simulink model "model"  (R2014a)
(part 7 of 8)

  房総線_CN_151379730_500000_CN_168727982_500000 : powerlib/Elements/Distributed Parameters Line  Phases=3  Frequency=60  Resistance=[0.01273 0.3864]  Inductance="[0.9337e-3  4.1264e-3]"  Capacitance=[12.74e-9 7.751e-9]  Length=39.9619  x1=[0 0 0 0; 0.0001244 0 0 0; 0.0002488 0 0 0; 0.0003733 0 0 0; 0.0004977 0 0 0; 0.0006221 0 0 0]  x2=[0 0 0 0; 0.0001244 0 0 0; 0.0002488 0 0 0; 0.0003733 0 0 0; 0.0004977 0 0 0; 0.0006221 0 0 0]  x3=[0 0 0 0; 0.0001244 0 0 0; 0.0002488 0 0 0; 0.0003733 0 0 0; 0.0004977 0 0 0; 0.0006221 0 0 0]  x4=[0 0 0 0; 0.0001244 0 0 0; 0.0002488 0 0 0; 0.0003733 0 0 0; 0.0004977 0 0 0; 0.0006221 0 0 0]  x5=0  V1=ones(3,3)  V2=ones(3,3)  I1=ones(3,3)  I2=ones(3,3)  nHarmo=1  Measurements=None
  新京葉線_CN_133135172_500000_CN_151706977_500000 : powerlib/Elements/Distributed Parameters Line  Phases=3  Frequency=60  Resistance=[0.01273 0.3864]  Inductance="[0.9337e-3  4.1264e-3]"  Capacitance=[12.74e-9 7.751e-9]  Length=22.6829  x1=[0 0 0 0; 0.0001244 0 0 0; 0.0002488 0 0 0; 0.0003733 0 0 0; 0.0004977 0 0 0; 0.0006221 0 0 0]  x2=[0 0 0 0; 0.0001244 0 0 0; 0.0002488 0 0 0; 0.0003733 0 0 0; 0.0004977 0 0 0; 0.0006221 0 0 0]  x3=[0 0 0 0; 0.0001244 0 0 0; 0.0002488 0 0 0; 0.0003733 0 0 0; 0.0004977 0 0 0; 0.0006221 0 0 0]  x4=[0 0 0 0; 0.0001244 0 0 0; 0.0002488 0 0 0; 0.0003733 0 0 0; 0.0004977 0 0 0; 0.0006221 0 0 0]  x5=0  V1=ones(3,3)  V2=ones(3,3)  I1=ones(3,3)  I2=ones(3,3)  nHarmo=1  Measurements=None
  新京葉線_CN_133135172_500000_CN_168727982_500000 : powerlib/Elements/Distributed Parameters Line  Phases=3  Frequency=60  Resistance=[0.01273 0.3864]  Inductance="[0.9337e-3  4.1264e-3]"  Capacitance=[12.74e-9 7.751e-9]  Length=45.831  x1=[0 0 0 0; 0.0001244 0 0 0; 0.0002488 0 0 0; 0.0003733 0 0 0; 0.0004977 0 0 0; 0.0006221 0 0 0]  x2=[0 0 0 0; 0.0001244 0 0 0; 0.0002488 0 0 0; 0.0003733 0 0 0; 0.0004977 0 0 0; 0.0006221 0 0 0]  x3=[0 0 0 0; 0.0001244 0 0 0; 0.0002488 0 0 0; 0.0003733 0 0 0; 0.0004977 0 0 0; 0.0006221 0 0 0]  x4=[0 0 0 0; 0.0001244 0 0 0; 0.0002488 0 0 0; 0.0003733 0 0 0; 0.0004977 0 0 0; 0.0006221 0 0 0]  x5=0  V1=ones(3,3)  V2=ones(3,3)  I1=ones(3,3)  I2=ones(3,3)  nHarmo=1  Measurements=None
  新京葉線_CN_151706977_275000_CN_168852840_275000 : powerlib/Elements/Distributed Parameters Line  Phases=3  Frequency=60  Resistance=[0.01273 0.3864]  Inductance="[0.9337e-3  4.1264e-3]"  Capacitance=[12.74e-9 7.751e-9]  Length=70.4447  x1=[0 0 0 0; 0.0001244 0 0 0; 0.0002488 0 0 0; 0.0003733 0 0 0; 0.0004977 0 0 0; 0.0006221 0 0 0]  x2=[0 0 0 0; 0.0001244 0 0 0; 0.0002488 0 0 0; 0.0003733 0 0 0; 0.0004977 0 0 0; 0.0006221 0 0 0]  x3=[0 0 0 0; 0.0001244 0 0 0; 0.0002488 0 0 0; 0.0003733 0 0 0; 0.0004977 0 0 0; 0.0006221 0 0 0]  x4=[0 0 0 0; 0.0001244 0 0 0; 0.0002488 0 0 0; 0.0003733 0 0 0; 0.0004977 0 0 0; 0.0006221 0 0 0]  x5=0  V1=ones(3,3)  V2=ones(3,3)  I1=ones(3,3)  I2=ones(3,3)  nHarmo=1  Measurements=None
  新古河線_(Shin_Koga_Sen)_CN_133135172_500000_CN_133641619_500000 : powerlib/Elements/Distributed Parameters Line  Phases=3  Frequency=60  Resistance=[0.01273 0.3864]  Inductance="[0.9337e-3  4.1264e-3]"  Capacitance=[12.74e-9 7.751e-9]  Length=56.7109  x1=[0 0 0 0; 0.0001244 0 0 0; 0.0002488 0 0 0; 0.0003733 0 0 0; 0.0004977 0 0 0; 0.0006221 0 0 0]  x2=[0 0 0 0; 0.0001244 0 0 0; 0.0002488 0 0 0; 0.0003733 0 0 0; 0.0004977 0 0 0; 0.0006221 0 0 0]  x3=[0 0 0 0; 0.0001244 0 0 0; 0.0002488 0 0 0; 0.0003733 0 0 0; 0.0004977 0 0 0; 0.0006221 0 0 0]  x4=[0 0 0 0; 0.0001244 0 0 0; 0.0002488 0 0 0; 0.0003733 0 0 0; 0.0004977 0 0 0; 0.0006221 0 0 0]  x5=0  V1=ones(3,3)  V2=ones(3,3)  I1=ones(3,3)  I2=ones(3,3)  nHarmo=1  Measurements=None
  新吾妻線_CN_169963236_500000_CN_66098469_500000 : powerlib/Elements/Distributed Parameters Line  Phases=3  Frequency=60  Resistance=[0.01273 0.3864]  Inductance="[0.9337e-3  4.1264e-3]"  Capacitance=[12.74e-9 7.751e-9]  Length=6.9915  x1=[0 0 0 0; 0.0001244 0 0 0; 0.0002488 0 0 0; 0.0003733 0 0 0; 0.0004977 0 0 0; 0.0006221 0 0 0]  x2=[0 0 0 0; 0.0001244 0 0 0; 0.0002488 0 0 0; 0.0003733 0 0 0; 0.0004977 0 0 0; 0.0006221 0 0 0]  x3=[0 0 0 0; 0.0001244 0 0 0; 0.0002488 0 0 0; 0.0003733 0 0 0; 0.0004977 0 0 0; 0.0006221 0 0 0]  x4=[0 0 0 0; 0.0001244 0 0 0; 0.0002488 0 0 0; 0.0003733 0 0 0; 0.0004977 0 0 0; 0.0006221 0 0 0]  x5=0  V1=ones(3,3)  V2=ones(3,3)  I1=ones(3,3)  I2=ones(3,3)  nHarmo=1  Measurements=None
  新坂戸線_CN_128581912_500000_CN_133641619_500000 : powerlib/Elements/Distributed Parameters Line  Phases=3  Frequency=60  Resistance=[0.01273 0.3864]  Inductance="[0.9337e-3  4.1264e-3]"  Capacitance=[12.74e-9 7.751e-9]  Length=7.2466  x1=[0 0 0 0; 0.0001244 0 0 0; 0.0002488 0 0 0; 0.0003733 0 0 0; 0.0004977 0 0 0; 0.0006221 0 0 0]  x2=[0 0 0 0; 0.0001244 0 0 0; 0.0002488 0 0 0; 0.0003733 0 0 0; 0.0004977 0 0 0; 0.0006221 0 0 0]  x3=[0 0 0 0; 0.0001244 0 0 0; 0.0002488 0 0 0; 0.0003733 0 0 0; 0.0004977 0 0 0; 0.0006221 0 0 0]  x4=[0 0 0 0; 0.0001244 0 0 0; 0.0002488 0 0 0; 0.0003733 0 0 0; 0.0004977 0 0 0; 0.0006221 0 0 0]  x5=0  V1=ones(3,3)  V2=ones(3,3)  I1=ones(3,3)  I2=ones(3,3)  nHarmo=1  Measurements=None
  新多摩線_(Shin_Tama_Sen)_CN_149843487_500000_CN_145079972_500000 : powerlib/Elements/Distributed Parameters Line  Phases=3  Frequency=60  Resistance=[0.01273 0.3864]  Inductance="[0.9337e-3  4.1264e-3]"  Capacitance=[12.74e-9 7.751e-9]  Length=39.8761  x1=[0 0 0 0; 0.0001244 0 0 0; 0.0002488 0 0 0; 0.0003733 0 0 0; 0.0004977 0 0 0; 0.0006221 0 0 0]  x2=[0 0 0 0; 0.0001244 0 0 0; 0.0002488 0 0 0; 0.0003733 0 0 0; 0.0004977 0 0 0; 0.0006221 0 0 0]  x3=[0 0 0 0; 0.0001244 0 0 0; 0.0002488 0 0 0; 0.0003733 0 0 0; 0.0004977 0 0 0; 0.0006221 0 0 0]  x4=[0 0 0 0; 0.0001244 0 0 0; 0.0002488 0 0 0; 0.0003733 0 0 0; 0.0004977 0 0 0; 0.0006221 0 0 0]  x5=0  V1=ones(3,3)  V2=ones(3,3)  I1=ones(3,3)  I2=ones(3,3)  nHarmo=1  Measurements=None
  新所沢線_(Shin_Tokorozawa_Sen)_CN_145079972_500000_CN_133641619_500000 : powerlib/Elements/Distributed Parameters Line  Phases=3  Frequency=60  Resistance=[0.01273 0.3864]  Inductance="[0.9337e-3  4.1264e-3]"  Capacitance=[12.74e-9 7.751e-9]  Length=34.7552  x1=[0 0 0 0; 0.0001244 0 0 0; 0.0002488 0 0 0; 0.0003733 0 0 0; 0.0004977 0 0 0; 0.0006221 0 0 0]  x2=[0 0 0 0; 0.0001244 0 0 0; 0.0002488 0 0 0; 0.0003733 0 0 0; 0.0004977 0 0 0; 0.0006221 0 0 0]  x3=[0 0 0 0; 0.0001244 0 0 0; 0.0002488 0 0 0; 0.0003733 0 0 0; 0.0004977 0 0 0; 0.0006221 0 0 0]  x4=[0 0 0 0; 0.0001244 0 0 0; 0.0002488 0 0 0; 0.0003733 0 0 0; 0.0004977 0 0 0; 0.0006221 0 0 0]  x5=0  V1=ones(3,3)  V2=ones(3,3)  I1=ones(3,3)  I2=ones(3,3)  nHarmo=1  Measurements=None
  新榛名線_CN_169963227_500000_CN_195615141_500000 : powerlib/Elements/Distributed Parameters Line  Phases=3  Frequency=60  Resistance=[0.01273 0.3864]  Inductance="[0.9337e-3  4.1264e-3]"  Capacitance=[12.74e-9 7.751e-9]  Length=67.752  x1=[0 0 0 0; 0.0001244 0 0 0; 0.0002488 0 0 0; 0.0003733 0 0 0; 0.0004977 0 0 0; 0.0006221 0 0 0]  x2=[0 0 0 0; 0.0001244 0 0 0; 0.0002488 0 0 0; 0.0003733 0 0 0; 0.0004977 0 0 0; 0.0006221 0 0 0]  x3=[0 0 0 0; 0.0001244 0 0 0; 0.0002488 0 0 0; 0.0003733 0 0 0; 0.0004977 0 0 0; 0.0006221 0 0 0]  x4=[0 0 0 0; 0.0001244 0 0 0; 0.0002488 0 0 0; 0.0003733 0 0 0; 0.0004977 0 0 0; 0.0006221 0 0 0]  x5=0  V1=ones(3,3)  V2=ones(3,3)  I1=ones(3,3)  I2=ones(3,3)  nHarmo=1  Measurements=None
  新筑波線_(Shin_Tsukuba_Sen)_CN_133135172_500000_CN_132913106_500000 : powerlib/Elements/Distributed Parameters Line  Phases=3  Frequency=60  Resistance=[0.01273 0.3864]  Inductance="[0.9337e-3  4.1264e-3]"  Capacitance=[12.74e-9 7.751e-9]  Length=9.3755  x1=[0 0 0 0; 0.0001244 0 0 0; 0.0002488 0 0 0; 0.0003733 0 0 0; 0.0004977 0 0 0; 0.0006221 0 0 0]  x2=[0 0 0 0; 0.0001244 0 0 0; 0.0002488 0 0 0; 0.0003733 0 0 0; 0.0004977 0 0 0; 0.0006221 0 0 0]  x3=[0 0 0 0; 0.0001244 0 0 0; 0.0002488 0 0 0; 0.0003733 0 0 0; 0.0004977 0 0 0; 0.0006221 0 0 0]  x4=[0 0 0 0; 0.0001244 0 0 0; 0.0002488 0 0 0; 0.0003733 0 0 0; 0.0004977 0 0 0; 0.0006221 0 0 0]  x5=0  V1=ones(3,3)  V2=ones(3,3)  I1=ones(3,3)  I2=ones(3,3)  nHarmo=1  Measurements=None
  新茂木線_(Shin_Motegi_Sen)_CN_104530060_500000_CN_168839127_500000 : powerlib/Elements/Distributed Parameters Line  Phases=3  Frequency=60  Resistance=[0.01273 0.3864]  Inductance="[0.9337e-3  4.1264e-3]"  Capacitance=[12.74e-9 7.751e-9]  Length=27.1693  x1=[0 0 0 0; 0.0001244 0 0 0; 0.0002488 0 0 0; 0.0003733 0 0 0; 0.0004977 0 0 0; 0.0006221 0 0 0]  x2=[0 0 0 0; 0.0001244 0 0 0; 0.0002488 0 0 0; 0.0003733 0 0 0; 0.0004977 0 0 0; 0.0006221 0 0 0]  x3=[0 0 0 0; 0.0001244 0 0 0; 0.0002488 0 0 0; 0.0003733 0 0 0; 0.0004977 0 0 0; 0.0006221 0 0 0]  x4=[0 0 0 0; 0.0001244 0 0 0; 0.0002488 0 0 0; 0.0003733 0 0 0; 0.0004977 0 0 0; 0.0006221 0 0 0]  x5=0  V1=ones(3,3)  V2=ones(3,3)  I1=ones(3,3)  I2=ones(3,3)  nHarmo=1  Measurements=None
  東京中線_CN_133137636_275000_CN_128581912_275000 : powerlib/Elements/Distributed Parameters Line  Phases=3  Frequency=60  Resistance=[0.01273 0.3864]  Inductance="[0.9337e-3  4.1264e-3]"  Capacitance=[12.74e-9 7.751e-9]  Length=25.3762  x1=[0 0 0 0; 0.0001244 0 0 0; 0.0002488 0 0 0; 0.0003733 0 0 0; 0.0004977 0 0 0; 0.0006221 0 0 0]  x2=[0 0 0 0; 0.0001244 0 0 0; 0.0002488 0 0 0; 0.0003733 0 0 0; 0.0004977 0 0 0; 0.0006221 0 0 0]  x3=[0 0 0 0; 0.0001244 0 0 0; 0.0002488 0 0 0; 0.0003733 0 0 0; 0.0004977 0 0 0; 0.0006221 0 0 0]  x4=[0 0 0 0; 0.0001244 0 0 0; 0.0002488 0 0 0; 0.0003733 0 0 0; 0.0004977 0 0 0; 0.0006221 0 0 0]  x5=0  V1=ones(3,3)  V2=ones(3,3)  I1=ones(3,3)  I2=ones(3,3)  nHarmo=1  Measurements=None
  東京北線_(Tōkyō_Kita_Sen)_CN_133137636_275000_CN_151706977_275000 : powerlib/Elements/Distributed Parameters Line  Phases=3  Frequency=60  Resistance=[0.01273 0.3864]  Inductance="[0.9337e-3  4.1264e-3]"  Capacitance=[12.74e-9 7.751e-9]  Length=25.1708  x1=[0 0 0 0; 0.0001244 0 0 0; 0.0002488 0 0 0; 0.0003733 0 0 0; 0.0004977 0 0 0; 0.0006221 0 0 0]  x2=[0 0 0 0; 0.0001244 0 0 0; 0.0002488 0 0 0; 0.0003733 0 0 0; 0.0004977 0 0 0; 0.0006221 0 0 0]  x3=[0 0 0 0; 0.0001244 0 0 0; 0.0002488 0 0 0; 0.0003733 0 0 0; 0.0004977 0 0 0; 0.0006221 0 0 0]  x4=[0 0 0 0; 0.0001244 0 0 0; 0.0002488 0 0 0; 0.0003733 0 0 0; 0.0004977 0 0 0; 0.0006221 0 0 0]  x5=0  V1=ones(3,3)  V2=ones(3,3)  I1=ones(3,3)  I2=ones(3,3)  nHarmo=1  Measurements=None
  東京南線3;4号線_CN_128364781_275000_CN_379474501_275000 : powerlib/Elements/Distributed Parameters Line  Phases=3  Frequency=60  Resistance=[0.01273 0.3864]  Inductance="[0.9337e-3  4.1264e-3]"  Capacitance=[12.74e-9 7.751e-9]  Length=35.3731  x1=[0 0 0 0; 0.0001244 0 0 0; 0.0002488 0 0 0; 0.0003733 0 0 0; 0.0004977 0 0 0; 0.0006221 0 0 0]  x2=[0 0 0 0; 0.0001244 0 0 0; 0.0002488 0 0 0; 0.0003733 0 0 0; 0.0004977 0 0 0; 0.0006221 0 0 0]  x3=[0 0 0 0; 0.0001244 0 0 0; 0.0002488 0 0 0; 0.0003733 0 0 0; 0.0004977 0 0 0; 0.0006221 0 0 0]  x4=[0 0 0 0; 0.0001244 0 0 0; 0.0002488 0 0 0; 0.0003733 0 0 0; 0.0004977 0 0 0; 0.0006221 0 0 0]  x5=0  V1=ones(3,3)  V2=ones(3,3)  I1=ones(3,3)  I2=ones(3,3)  nHarmo=1  Measurements=None
  東京西線_CN_145080115_275000_CN_47110637_275000 : powerlib/Elements/Distributed Parameters Line  Phases=3  Frequency=60  Resistance=[0.01273 0.3864]  Inductance="[0.9337e-3  4.1264e-3]"  Capacitance=[12.74e-9 7.751e-9]  Length=13.2046  x1=[0 0 0 0; 0.0001244 0 0 0; 0.0002488 0 0 0; 0.0003733 0 0 0; 0.0004977 0 0 0; 0.0006221 0 0 0]  x2=[0 0 0 0; 0.0001244 0 0 0; 0.0002488 0 0 0; 0.0003733 0 0 0; 0.0004977 0 0 0; 0.0006221 0 0 0]  x3=[0 0 0 0; 0.0001244 0 0 0; 0.0002488 0 0 0; 0.0003733 0 0 0; 0.0004977 0 0 0; 0.0006221 0 0 0]  x4=[0 0 0 0; 0.0001244 0 0 0; 0.0002488 0 0 0; 0.0003733 0 0 0; 0.0004977 0 0 0; 0.0006221 0 0 0]  x5=0  V1=ones(3,3)  V2=ones(3,3)  I1=ones(3,3)  I2=ones(3,3)  nHarmo=1  Measurements=None
  東群馬幹線_CN_250540807_500000_CN_66098469_500000 : powerlib/Elements/Distributed Parameters Line  Phases=3  Frequency=60  Resistance=[0.01273 0.3864]  Inductance="[0.9337e-3  4.1264e-3]"  Capacitance=[12.74e-9 7.751e-9]  Length=44.432  x1=[0 0 0 0; 0.0001244 0 0 0; 0.0002488 0 0 0; 0.0003733 0 0 0; 0.0004977 0 0 0; 0.0006221 0 0 0]  x2=[0 0 0 0; 0.0001244 0 0 0; 0.0002488 0 0 0; 0.0003733 0 0 0; 0.0004977 0 0 0; 0.0006221 0 0 0]  x3=[0 0 0 0; 0.0001244 0 0 0; 0.0002488 0 0 0; 0.0003733 0 0 0; 0.0004977 0 0 0; 0.0006221 0 0 0]  x4=[0 0 0 0; 0.0001244 0 0 0; 0.0002488 0 0 0; 0.0003733 0 0 0; 0.0004977 0 0 0; 0.0006221 0 0 0]  x5=0  V1=ones(3,3)  V2=ones(3,3)  I1=ones(3,3)  I2=ones(3,3)  nHarmo=1  Measurements=None
  河北1・2線_(Kahoku_1・2_Sen)_CN_133137636_275000_CN_133135172_275000 : powerlib/Elements/Distributed Parameters Line  Phases=3  Frequency=60  Resistance=[0.01273 0.3864]  Inductance="[0.9337e-3  4.1264e-3]"  Capacitance=[12.74e-9 7.751e-9]  Length=16.922  x1=[0 0 0 0; 0.0001244 0 0 0; 0.0002488 0 0 0; 0.0003733 0 0 0; 0.0004977 0 0 0; 0.0006221 0 0 0]  x2=[0 0 0 0; 0.0001244 0 0 0; 0.0002488 0 0 0; 0.0003733 0 0 0; 0.0004977 0 0 0; 0.0006221 0 0 0]  x3=[0 0 0 0; 0.0001244 0 0 0; 0.0002488 0 0 0; 0.0003733 0 0 0; 0.0004977 0 0 0; 0.0006221 0 0 0]  x4=[0 0 0 0; 0.0001244 0 0 0; 0.0002488 0 0 0; 0.0003733 0 0 0; 0.0004977 0 0 0; 0.0006221 0 0 0]  x5=0  V1=ones(3,3)  V2=ones(3,3)  I1=ones(3,3)  I2=ones(3,3)  nHarmo=1  Measurements=None
  泉南東大阪線_(Sennan_Higashiōsaka_sen)_CN_108199478_275000_CN_158522649_275000 : powerlib/Elements/Distributed Parameters Line  Phases=3  Frequency=60  Resistance=[0.01273 0.3864]  Inductance="[0.9337e-3  4.1264e-3]"  Capacitance=[12.74e-9 7.751e-9]  Length=43.4062  x1=[0 0 0 0; 0.0001244 0 0 0; 0.0002488 0 0 0; 0.0003733 0 0 0; 0.0004977 0 0 0; 0.0006221 0 0 0]  x2=[0 0 0 0; 0.0001244 0 0 0; 0.0002488 0 0 0; 0.0003733 0 0 0; 0.0004977 0 0 0; 0.0006221 0 0 0]  x3=[0 0 0 0; 0.0001244 0 0 0; 0.0002488 0 0 0; 0.0003733 0 0 0; 0.0004977 0 0 0; 0.0006221 0 0 0]  x4=[0 0 0 0; 0.0001244 0 0 0; 0.0002488 0 0 0; 0.0003733 0 0 0; 0.0004977 0 0 0; 0.0006221 0 0 0]  x5=0  V1=ones(3,3)  V2=ones(3,3)  I1=ones(3,3)  I2=ones(3,3)  nHarmo=1  Measurements=None
  湖西三河線_CN_170247308_275000_CN_170260165_275000 : powerlib/Elements/Distributed Parameters Line  Phases=3  Frequency=60  Resistance=[0.01273 0.3864]  Inductance="[0.9337e-3  4.1264e-3]"  Capacitance=[12.74e-9 7.751e-9]  Length=17.3479  x1=[0 0 0 0; 0.0001244 0 0 0; 0.0002488 0 0 0; 0.0003733 0 0 0; 0.0004977 0 0 0; 0.0006221 0 0 0]  x2=[0 0 0 0; 0.0001244 0 0 0; 0.0002488 0 0 0; 0.0003733 0 0 0; 0.0004977 0 0 0; 0.0006221 0 0 0]  x3=[0 0 0 0; 0.0001244 0 0 0; 0.0002488 0 0 0; 0.0003733 0 0 0; 0.0004977 0 0 0; 0.0006221 0 0 0]  x4=[0 0 0 0; 0.0001244 0 0 0; 0.0002488 0 0 0; 0.0003733 0 0 0; 0.0004977 0 0 0; 0.0006221 0 0 0]  x5=0  V1=ones(3,3)  V2=ones(3,3)  I1=ones(3,3)  I2=ones(3,3)  nHarmo=1  Measurements=None
  田原湖西線_CN_170260165_275000_CN_170260169_275000 : powerlib/Elements/Distributed Parameters Line  Phases=3  Frequency=60  Resistance=[0.01273 0.3864]  Inductance="[0.9337e-3  4.1264e-3]"  Capacitance=[12.74e-9 7.751e-9]  Length=20.2601  x1=[0 0 0 0; 0.0001244 0 0 0; 0.0002488 0 0 0; 0.0003733 0 0 0; 0.0004977 0 0 0; 0.0006221 0 0 0]  x2=[0 0 0 0; 0.0001244 0 0 0; 0.0002488 0 0 0; 0.0003733 0 0 0; 0.0004977 0 0 0; 0.0006221 0 0 0]  x3=[0 0 0 0; 0.0001244 0 0 0; 0.0002488 0 0 0; 0.0003733 0 0 0; 0.0004977 0 0 0; 0.0006221 0 0 0]  x4=[0 0 0 0; 0.0001244 0 0 0; 0.0002488 0 0 0; 0.0003733 0 0 0; 0.0004977 0 0 0; 0.0006221 0 0 0]  x5=0  V1=ones(3,3)  V2=ones(3,3)  I1=ones(3,3)  I2=ones(3,3)  nHarmo=1  Measurements=None
  福島幹線_CN_104391636_500000_CN_168839127_500000 : powerlib/Elements/Distributed Parameters Line  Phases=3  Frequency=60  Resistance=[0.01273 0.3864]  Inductance="[0.9337e-3  4.1264e-3]"  Capacitance=[12.74e-9 7.751e-9]  Length=79.9432  x1=[0 0 0 0; 0.0001244 0 0 0; 0.0002488 0 0 0; 0.0003733 0 0 0; 0.0004977 0 0 0; 0.0006221 0 0 0]  x2=[0 0 0 0; 0.0001244 0 0 0; 0.0002488 0 0 0; 0.0003733 0 0 0; 0.0004977 0 0 0; 0.0006221 0 0 0]  x3=[0 0 0 0; 0.0001244 0 0 0; 0.0002488 0 0 0; 0.0003733 0 0 0; 0.0004977 0 0 0; 0.0006221 0 0 0]  x4=[0 0 0 0; 0.0001244 0 0 0; 0.0002488 0 0 0; 0.0003733 0 0 0; 0.0004977 0 0 0; 0.0006221 0 0 0]  x5=0  V1=ones(3,3)  V2=ones(3,3)  I1=ones(3,3)  I2=ones(3,3)  nHarmo=1  Measurements=None
  福島幹線_CN_133135172_500000_CN_168839127_500000 : powerlib/Elements/Distributed Parameters Line  Phases=3  Frequency=60  Resistance=[0.01273 0.3864]  Inductance="[0.9337e-3  4.1264e-3]"  Capacitance=[12.74e-9 7.751e-9]  Length=59.1144  x1=[0 0 0 0; 0.0001244 0 0 0; 0.0002488 0 0 0; 0.0003733 0 0 0; 0.0004977 0 0 0; 0.0006221 0 0 0]  x2=[0 0 0 0; 0.0001244 0 0 0; 0.0002488 0 0 0; 0.0003733 0 0 0; 0.0004977 0 0 0; 0.0006221 0 0 0]  x3=[0 0 0 0; 0.0001244 0 0 0; 0.0002488 0 0 0; 0.0003733 0 0 0; 0.0004977 0 0 0; 0.0006221 0 0 0]  x4=[0 0 0 0; 0.0001244 0 0 0; 0.0002488 0 0 0; 0.0003733 0 0 0; 0.0004977 0 0 0; 0.0006221 0 0 0]  x5=0  V1=ones(3,3)  V2=ones(3,3)  I1=ones(3,3)  I2=ones(3,3)  nHarmo=1  Measurements=None
  福島東幹線2_CN_106309481_500000_CN_104391636_500000 : powerlib/Elements/Distributed Parameters Line  Phases=3  Frequency=60  Resistance=[0.01273 0.3864]  Inductance="[0.9337e-3  4.1264e-3]"  Capacitance=[12.74e-9 7.751e-9]  Length=33.091  x1=[0 0 0 0; 0.0001244 0 0 0; 0.0002488 0 0 0; 0.0003733 0 0 0; 0.0004977 0 0 0; 0.0006221 0 0 0]  x2=[0 0 0 0; 0.0001244 0 0 0; 0.0002488 0 0 0; 0.0003733 0 0 0; 0.0004977 0 0 0; 0.0006221 0 0 0]  x3=[0 0 0 0; 0.0001244 0 0 0; 0.0002488 0 0 0; 0.0003733 0 0 0; 0.0004977 0 0 0; 0.0006221 0 0 0]  x4=[0 0 0 0; 0.0001244 0 0 0; 0.0002488 0 0 0; 0.0003733 0 0 0; 0.0004977 0 0 0; 0.0006221 0 0 0]  x5=0  V1=ones(3,3)  V2=ones(3,3)  I1=ones(3,3)  I2=ones(3,3)  nHarmo=1  Measurements=None
  秦浜線_CN_162844704_275000_CN_128364781_275000 : powerlib/Elements/Distributed Parameters Line  Phases=3  Frequency=60  Resistance=[0.01273 0.3864]  Inductance="[0.9337e-3  4.1264e-3]"  Capacitance=[12.74e-9 7.751e-9]  Length=9.0606  x1=[0 0 0 0; 0.0001244 0 0 0; 0.0002488 0 0 0; 0.0003733 0 0 0; 0.0004977 0 0 0; 0.0006221 0 0 0]  x2=[0 0 0 0; 0.0001244 0 0 0; 0.0002488 0 0 0; 0.0003733 0 0 0; 0.0004977 0 0 0; 0.0006221 0 0 0]  x3=[0 0 0 0; 0.0001244 0 0 0; 0.0002488 0 0 0; 0.0003733 0 0 0; 0.0004977 0 0 0; 0.0006221 0 0 0]  x4=[0 0 0 0; 0.0001244 0 0 0; 0.0002488 0 0 0; 0.0003733 0 0 0; 0.0004977 0 0 0; 0.0006221 0 0 0]  x5=0  V1=ones(3,3)  V2=ones(3,3)  I1=ones(3,3)  I2=ones(3,3)  nHarmo=1  Measurements=None
  脊振鳥栖線_CN_172601929_220000_CN_173793392_220000 : powerlib/Elements/Distributed Parameters Line  Phases=3  Frequency=60  Resistance=[0.01273 0.3864]  Inductance="[0.9337e-3  4.1264e-3]"  Capacitance=[12.74e-9 7.751e-9]  Length=18.4331  x1=[0 0 0 0; 0.0001244 0 0 0; 0.0002488 0 0 0; 0.0003733 0 0 0; 0.0004977 0 0 0; 0.0006221 0 0 0]  x2=[0 0 0 0; 0.0001244 0 0 0; 0.0002488 0 0 0; 0.0003733 0 0 0; 0.0004977 0 0 0; 0.0006221 0 0 0]  x3=[0 0 0 0; 0.0001244 0 0 0; 0.0002488 0 0 0; 0.0003733 0 0 0; 0.0004977 0 0 0; 0.0006221 0 0 0]  x4=[0 0 0 0; 0.0001244 0 0 0; 0.0002488 0 0 0; 0.0003733 0 0 0; 0.0004977 0 0 0; 0.0006221 0 0 0]  x5=0  V1=ones(3,3)  V2=ones(3,3)  I1=ones(3,3)  I2=ones(3,3)  nHarmo=1  Measurements=None
  脊振鳥栖線_CN_172601929_220000_CN_174915836_220000 : powerlib/Elements/Distributed Parameters Line  Phases=3  Frequency=60  Resistance=[0.01273 0.3864]  Inductance="[0.9337e-3  4.1264e-3]"  Capacitance=[12.74e-9 7.751e-9]  Length=42.4891  x1=[0 0 0 0; 0.0001244 0 0 0; 0.0002488 0 0 0; 0.0003733 0 0 0; 0.0004977 0 0 0; 0.0006221 0 0 0]  x2=[0 0 0 0; 0.0001244 0 0 0; 0.0002488 0 0 0; 0.0003733 0 0 0; 0.0004977 0 0 0; 0.0006221 0 0 0]  x3=[0 0 0 0; 0.0001244 0 0 0; 0.0002488 0 0 0; 0.0003733 0 0 0; 0.0004977 0 0 0; 0.0006221 0 0 0]  x4=[0 0 0 0; 0.0001244 0 0 0; 0.0002488 0 0 0; 0.0003733 0 0 0; 0.0004977 0 0 0; 0.0006221 0 0 0]  x5=0  V1=ones(3,3)  V2=ones(3,3)  I1=ones(3,3)  I2=ones(3,3)  nHarmo=1  Measurements=None
  花見川線_CN_210765350_275000_CN_211241774_275000 : powerlib/Elements/Distributed Parameters Line  Phases=3  Frequency=60  Resistance=[0.01273 0.3864]  Inductance="[0.9337e-3  4.1264e-3]"  Capacitance=[12.74e-9 7.751e-9]  Length=41.8493  x1=[0 0 0 0; 0.0001244 0 0 0; 0.0002488 0 0 0; 0.0003733 0 0 0; 0.0004977 0 0 0; 0.0006221 0 0 0]  x2=[0 0 0 0; 0.0001244 0 0 0; 0.0002488 0 0 0; 0.0003733 0 0 0; 0.0004977 0 0 0; 0.0006221 0 0 0]  x3=[0 0 0 0; 0.0001244 0 0 0; 0.0002488 0 0 0; 0.0003733 0 0 0; 0.0004977 0 0 0; 0.0006221 0 0 0]  x4=[0 0 0 0; 0.0001244 0 0 0; 0.0002488 0 0 0; 0.0003733 0 0 0; 0.0004977 0 0 0; 0.0006221 0 0 0]  x5=0  V1=ones(3,3)  V2=ones(3,3)  I1=ones(3,3)  I2=ones(3,3)  nHarmo=1  Measurements=None
  西越谷線_(Nishi_Koshigaya_Sen)_CN_155411568_275000_CN_133137636_275000 : powerlib/Elements/Distributed Parameters Line  Phases=3  Frequency=60  Resistance=[0.01273 0.3864]  Inductance="[0.9337e-3  4.1264e-3]"  Capacitance=[12.74e-9 7.751e-9]  Length=12.7535  x1=[0 0 0 0; 0.0001244 0 0 0; 0.0002488 0 0 0; 0.0003733 0 0 0; 0.0004977 0 0 0; 0.0006221 0 0 0]  x2=[0 0 0 0; 0.0001244 0 0 0; 0.0002488 0 0 0; 0.0003733 0 0 0; 0.0004977 0 0 0; 0.0006221 0 0 0]  x3=[0 0 0 0; 0.0001244 0 0 0; 0.0002488 0 0 0; 0.0003733 0 0 0; 0.0004977 0 0 0; 0.0006221 0 0 0]  x4=[0 0 0 0; 0.0001244 0 0 0; 0.0002488 0 0 0; 0.0003733 0 0 0; 0.0004977 0 0 0; 0.0006221 0 0 0]  x5=0  V1=ones(3,3)  V2=ones(3,3)  I1=ones(3,3)  I2=ones(3,3)  nHarmo=1  Measurements=None
  西越谷線_(Nishi_Koshigaya_Sen)_CN_155411568_275000_CN_153521822_275000 : powerlib/Elements/Distributed Parameters Line  Phases=3  Frequency=60  Resistance=[0.01273 0.3864]  Inductance="[0.9337e-3  4.1264e-3]"  Capacitance=[12.74e-9 7.751e-9]  Length=4.8337  x1=[0 0 0 0; 0.0001244 0 0 0; 0.0002488 0 0 0; 0.0003733 0 0 0; 0.0004977 0 0 0; 0.0006221 0 0 0]  x2=[0 0 0 0; 0.0001244 0 0 0; 0.0002488 0 0 0; 0.0003733 0 0 0; 0.0004977 0 0 0; 0.0006221 0 0 0]  x3=[0 0 0 0; 0.0001244 0 0 0; 0.0002488 0 0 0; 0.0003733 0 0 0; 0.0004977 0 0 0; 0.0006221 0 0 0]  x4=[0 0 0 0; 0.0001244 0 0 0; 0.0002488 0 0 0; 0.0003733 0 0 0; 0.0004977 0 0 0; 0.0006221 0 0 0]  x5=0  V1=ones(3,3)  V2=ones(3,3)  I1=ones(3,3)  I2=ones(3,3)  nHarmo=1  Measurements=None
  西部西濃線_(Seibu_Seinō_Sen)_CN_170537514_275000_CN_161948515_275000 : powerlib/Elements/Distributed Parameters Line  Phases=3  Frequency=60  Resistance=[0.01273 0.3864]  Inductance="[0.9337e-3  4.1264e-3]"  Capacitance=[12.74e-9 7.751e-9]  Length=31.9925  x1=[0 0 0 0; 0.0001244 0 0 0; 0.0002488 0 0 0; 0.0003733 0 0 0; 0.0004977 0 0 0; 0.0006221 0 0 0]  x2=[0 0 0 0; 0.0001244 0 0 0; 0.0002488 0 0 0; 0.0003733 0 0 0; 0.0004977 0 0 0; 0.0006221 0 0 0]  x3=[0 0 0 0; 0.0001244 0 0 0; 0.0002488 0 0 0; 0.0003733 0 0 0; 0.0004977 0 0 0; 0.0006221 0 0 0]  x4=[0 0 0 0; 0.0001244 0 0 0; 0.0002488 0 0 0; 0.0003733 0 0 0; 0.0004977 0 0 0; 0.0006221 0 0 0]  x5=0  V1=ones(3,3)  V2=ones(3,3)  I1=ones(3,3)  I2=ones(3,3)  nHarmo=1  Measurements=None
  豊根幹線_CN_142662111_500000_CN_170850727_500000 : powerlib/Elements/Distributed Parameters Line  Phases=3  Frequency=60  Resistance=[0.01273 0.3864]  Inductance="[0.9337e-3  4.1264e-3]"  Capacitance=[12.74e-9 7.751e-9]  Length=43.3502  x1=[0 0 0 0; 0.0001244 0 0 0; 0.0002488 0 0 0; 0.0003733 0 0 0; 0.0004977 0 0 0; 0.0006221 0 0 0]  x2=[0 0 0 0; 0.0001244 0 0 0; 0.0002488 0 0 0; 0.0003733 0 0 0; 0.0004977 0 0 0; 0.0006221 0 0 0]  x3=[0 0 0 0; 0.0001244 0 0 0; 0.0002488 0 0 0; 0.0003733 0 0 0; 0.0004977 0 0 0; 0.0006221 0 0 0]  x4=[0 0 0 0; 0.0001244 0 0 0; 0.0002488 0 0 0; 0.0003733 0 0 0; 0.0004977 0 0 0; 0.0006221 0 0 0]  x5=0  V1=ones(3,3)  V2=ones(3,3)  I1=ones(3,3)  I2=ones(3,3)  nHarmo=1  Measurements=None
  道央北幹線_CN_179863079_275000_CN_168524732_275000 : powerlib/Elements/Distributed Parameters Line  Phases=3  Frequency=60  Resistance=[0.01273 0.3864]  Inductance="[0.9337e-3  4.1264e-3]"  Capacitance=[12.74e-9 7.751e-9]  Length=32.9195  x1=[0 0 0 0; 0.0001244 0 0 0; 0.0002488 0 0 0; 0.0003733 0 0 0; 0.0004977 0 0 0; 0.0006221 0 0 0]  x2=[0 0 0 0; 0.0001244 0 0 0; 0.0002488 0 0 0; 0.0003733 0 0 0; 0.0004977 0 0 0; 0.0006221 0 0 0]  x3=[0 0 0 0; 0.0001244 0 0 0; 0.0002488 0 0 0; 0.0003733 0 0 0; 0.0004977 0 0 0; 0.0006221 0 0 0]  x4=[0 0 0 0; 0.0001244 0 0 0; 0.0002488 0 0 0; 0.0003733 0 0 0; 0.0004977 0 0 0; 0.0006221 0 0 0]  x5=0  V1=ones(3,3)  V2=ones(3,3)  I1=ones(3,3)  I2=ones(3,3)  nHarmo=1  Measurements=None
  那珂線_(Naka_Sen)_CN_105291887_275000_CN_168839127_275000 : powerlib/Elements/Distributed Parameters Line  Phases=3  Frequency=60  Resistance=[0.01273 0.3864]  Inductance="[0.9337e-3  4.1264e-3]"  Capacitance=[12.74e-9 7.751e-9]  Length=27.9495  x1=[0 0 0 0; 0.0001244 0 0 0; 0.0002488 0 0 0; 0.0003733 0 0 0; 0.0004977 0 0 0; 0.0006221 0 0 0]  x2=[0 0 0 0; 0.0001244 0 0 0; 0.0002488 0 0 0; 0.0003733 0 0 0; 0.0004977 0 0 0; 0.0006221 0 0 0]  x3=[0 0 0 0; 0.0001244 0 0 0; 0.0002488 0 0 0; 0.0003733 0 0 0; 0.0004977 0 0 0; 0.0006221 0 0 0]  x4=[0 0 0 0; 0.0001244 0 0 0; 0.0002488 0 0 0; 0.0003733 0 0 0; 0.0004977 0 0 0; 0.0006221 0 0 0]  x5=0  V1=ones(3,3)  V2=ones(3,3)  I1=ones(3,3)  I2=ones(3,3)  nHarmo=1  Measurements=None
  金剛線_(Kongō_sen)_CN_109834508_275000_CN_291678103_275000 : powerlib/Elements/Distributed Parameters Line  Phases=3  Frequency=60  Resistance=[0.01273 0.3864]  Inductance="[0.9337e-3  4.1264e-3]"  Capacitance=[12.74e-9 7.751e-9]  Length=41.6756  x1=[0 0 0 0; 0.0001244 0 0 0; 0.0002488 0 0 0; 0.0003733 0 0 0; 0.0004977 0 0 0; 0.0006221 0 0 0]  x2=[0 0 0 0; 0.0001244 0 0 0; 0.0002488 0 0 0; 0.0003733 0 0 0; 0.0004977 0 0 0; 0.0006221 0 0 0]  x3=[0 0 0 0; 0.0001244 0 0 0; 0.0002488 0 0 0; 0.0003733 0 0 0; 0.0004977 0 0 0; 0.0006221 0 0 0]  x4=[0 0 0 0; 0.0001244 0 0 0; 0.0002488 0 0 0; 0.0003733 0 0 0; 0.0004977 0 0 0; 0.0006221 0 0 0]  x5=0  V1=ones(3,3)  V2=ones(3,3)  I1=ones(3,3)  I2=ones(3,3)  nHarmo=1  Measurements=None
  関門連系線_CN_204258596_500000_CN_187988970_500000 : powerlib/Elements/Distributed Parameters Line  Phases=3  Frequency=60  Resistance=[0.01273 0.3864]  Inductance="[0.9337e-3  4.1264e-3]"  Capacitance=[12.74e-9 7.751e-9]  Length=64.174  x1=[0 0 0 0; 0.0001244 0 0 0; 0.0002488 0 0 0; 0.0003733 0 0 0; 0.0004977 0 0 0; 0.0006221 0 0 0]  x2=[0 0 0 0; 0.0001244 0 0 0; 0.0002488 0 0 0; 0.0003733 0 0 0; 0.0004977 0 0 0; 0.0006221 0 0 0]  x3=[0 0 0 0; 0.0001244 0 0 0; 0.0002488 0 0 0; 0.0003733 0 0 0; 0.0004977 0 0 0; 0.0006221 0 0 0]  x4=[0 0 0 0; 0.0001244 0 0 0; 0.0002488 0 0 0; 0.0003733 0 0 0; 0.0004977 0 0 0; 0.0006221 0 0 0]  x5=0  V1=ones(3,3)  V2=ones(3,3)  I1=ones(3,3)  I2=ones(3,3)  nHarmo=1  Measurements=None
  阿南紀北直流幹線_CN_109850439_500000_CN_217885658_500000 : powerlib/Elements/Distributed Parameters Line  Phases=3  Frequency=60  Resistance=[0.01273 0.3864]  Inductance="[0.9337e-3  4.1264e-3]"  Capacitance=[12.74e-9 7.751e-9]  Length=50.9846  x1=[0 0 0 0; 0.0001244 0 0 0; 0.0002488 0 0 0; 0.0003733 0 0 0; 0.0004977 0 0 0; 0.0006221 0 0 0]  x2=[0 0 0 0; 0.0001244 0 0 0; 0.0002488 0 0 0; 0.0003733 0 0 0; 0.0004977 0 0 0; 0.0006221 0 0 0]  x3=[0 0 0 0; 0.0001244 0 0 0; 0.0002488 0 0 0; 0.0003733 0 0 0; 0.0004977 0 0 0; 0.0006221 0 0 0]  x4=[0 0 0 0; 0.0001244 0 0 0; 0.0002488 0 0 0; 0.0003733 0 0 0; 0.0004977 0 0 0; 0.0006221 0 0 0]  x5=0  V1=ones(3,3)  V2=ones(3,3)  I1=ones(3,3)  I2=ones(3,3)  nHarmo=1  Measurements=None
  青梅線_(Ōme_Sen)_CN_133644487_275000_CN_145084773_275000 : powerlib/Elements/Distributed Parameters Line  Phases=3  Frequency=60  Resistance=[0.01273 0.3864]  Inductance="[0.9337e-3  4.1264e-3]"  Capacitance=[12.74e-9 7.751e-9]  Length=11.1139  x1=[0 0 0 0; 0.0001244 0 0 0; 0.0002488 0 0 0; 0.0003733 0 0 0; 0.0004977 0 0 0; 0.0006221 0 0 0]  x2=[0 0 0 0; 0.0001244 0 0 0; 0.0002488 0 0 0; 0.0003733 0 0 0; 0.0004977 0 0 0; 0.0006221 0 0 0]  x3=[0 0 0 0; 0.0001244 0 0 0; 0.0002488 0 0 0; 0.0003733 0 0 0; 0.0004977 0 0 0; 0.0006221 0 0 0]  x4=[0 0 0 0; 0.0001244 0 0 0; 0.0002488 0 0 0; 0.0003733 0 0 0; 0.0004977 0 0 0; 0.0006221 0 0 0]  x5=0  V1=ones(3,3)  V2=ones(3,3)  I1=ones(3,3)  I2=ones(3,3)  nHarmo=1  Measurements=None
  駿遠幹線_CN_116559939_500000_CN_210090094_500000 : powerlib/Elements/Distributed Parameters Line  Phases=3  Frequency=60  Resistance=[0.01273 0.3864]  Inductance="[0.9337e-3  4.1264e-3]"  Capacitance=[12.74e-9 7.751e-9]  Length=46.0694  x1=[0 0 0 0; 0.0001244 0 0 0; 0.0002488 0 0 0; 0.0003733 0 0 0; 0.0004977 0 0 0; 0.0006221 0 0 0]  x2=[0 0 0 0; 0.0001244 0 0 0; 0.0002488 0 0 0; 0.0003733 0 0 0; 0.0004977 0 0 0; 0.0006221 0 0 0]  x3=[0 0 0 0; 0.0001244 0 0 0; 0.0002488 0 0 0; 0.0003733 0 0 0; 0.0004977 0 0 0; 0.0006221 0 0 0]  x4=[0 0 0 0; 0.0001244 0 0 0; 0.0002488 0 0 0; 0.0003733 0 0 0; 0.0004977 0 0 0; 0.0006221 0 0 0]  x5=0  V1=ones(3,3)  V2=ones(3,3)  I1=ones(3,3)  I2=ones(3,3)  nHarmo=1  Measurements=None
  connections:
  _CN_201293312_220000_CN_216809817_220000/LConn1 -- T_201293312_500000;220000_/RConn1 -- _CN_201293312_220000_CN_259056356_220000/LConn1 -- _CN_201293312_220000_CN_90806466_220000/LConn1 -- L_201293312/LConn1
  _CN_201293312_220000_CN_216809817_220000/LConn2 -- T_201293312_500000;220000_/RConn2 -- _CN_201293312_220000_CN_259056356_220000/LConn2 -- _CN_201293312_220000_CN_90806466_220000/LConn2 -- L_201293312/LConn2
  _CN_201293312_220000_CN_216809817_220000/LConn3 -- T_201293312_500000;220000_/RConn3 -- _CN_201293312_220000_CN_259056356_220000/LConn3 -- _CN_201293312_220000_CN_90806466_220000/LConn3 -- L_201293312/LConn3 -- bus1/LConn1
  _CN_201293312_220000_CN_216809817_220000/RConn1 -- G_216809817_豊前火力発電所/RConn1 -- _CN_405806514_220000_CN_216809817_220000/LConn1
  _CN_201293312_220000_CN_216809817_220000/RConn2 -- G_216809817_豊前火力発電所/RConn2 -- _CN_405806514_220000_CN_216809817_220000/LConn2
  _CN_201293312_220000_CN_216809817_220000/RConn3 -- G_216809817_豊前火力発電所/RConn3 -- _CN_405806514_220000_CN_216809817_220000/LConn3 -- bus2/LConn1
  T_259056356__/LConn1 -- _CN_201293312_220000_CN_259056356_220000/RConn1
  T_259056356__/LConn2 -- _CN_201293312_220000_CN_259056356_220000/RConn2
  _CN_201293312_220000_CN_259056356_220000/RConn3 -- T_259056356__/LConn3 -- bus3/LConn1
  _CN_201293312_220000_CN_90806466_220000/RConn1 -- T_90806466_220000;66000_/LConn1 -- _CN_90806466_220000_CN_216949339_220000/LConn1
  _CN_201293312_220000_CN_90806466_220000/RConn2 -- T_90806466_220000;66000_/LConn2 -- _CN_90806466_220000_CN_216949339_220000/LConn2
  _CN_201293312_220000_CN_90806466_220000/RConn3 -- T_90806466_220000;66000_/LConn3 -- _CN_90806466_220000_CN_216949339_220000/LConn3 -- bus4/LConn1
  _CN_216498433_220000_CN_405626236_220000/LConn1 -- T_216498433_220000;110000;66000_九州電力_南熊本変電所/LConn1 -- _CN_216498433_220000_CN_203776442_220000/LConn1 -- _CN_216498433_220000_CN_216502300_220000/LConn1 -- _CN_216498433_220000_CN_216496817_220000/LConn1
  _CN_216498433_220000_CN_405626236_220000/LConn2 -- T_216498433_220000;110000;66000_九州電力_南熊本変電所/LConn2 -- _CN_216498433_220000_CN_203776442_220000/LConn2 -- _CN_216498433_220000_CN_216502300_220000/LConn2 -- _CN_216498433_220000_CN_216496817_220000/LConn2
  _CN_216498433_220000_CN_405626236_220000/LConn3 -- T_216498433_220000;110000;66000_九州電力_南熊本変電所/LConn3 -- _CN_216498433_220000_CN_203776442_220000/LConn3 -- _CN_216498433_220000_CN_216502300_220000/LConn3 -- _CN_216498433_220000_CN_216496817_220000/LConn3 -- bus5/LConn1
  _CN_216498433_220000_CN_405626236_220000/RConn1 -- T_405626236_220000_熊本変電所/RConn1 -- L_405626236/LConn1
  _CN_216498433_220000_CN_405626236_220000/RConn2 -- T_405626236_220000_熊本変電所/RConn2 -- L_405626236/LConn2
  _CN_216498433_220000_CN_405626236_220000/RConn3 -- T_405626236_220000_熊本変電所/RConn3 -- L_405626236/LConn3 -- bus6/LConn1
  _CN_216498433_220000_CN_203776442_220000/RConn1 -- T_203776442__/LConn1 -- _CN_203776442_220000_CN_174915836_220000/LConn1
  _CN_216498433_220000_CN_203776442_220000/RConn2 -- T_203776442__/LConn2 -- _CN_203776442_220000_CN_174915836_220000/LConn2
  _CN_216498433_220000_CN_203776442_220000/RConn3 -- T_203776442__/LConn3 -- _CN_203776442_220000_CN_174915836_220000/LConn3 -- bus7/LConn1
  _CN_216498433_220000_CN_216502300_220000/RConn1 -- T_216502300__九州電力_中九州変電所/RConn1 -- L_216502300/LConn1
  _CN_216498433_220000_CN_216502300_220000/RConn2 -- T_216502300__九州電力_中九州変電所/RConn2 -- L_216502300/LConn2
  _CN_216498433_220000_CN_216502300_220000/RConn3 -- T_216502300__九州電力_中九州変電所/RConn3 -- L_216502300/LConn3 -- bus8/LConn1
  _CN_216498433_220000_CN_216496817_220000/RConn1 -- T_216496817_220000;66000_九州電力人吉変電所/LConn1 -- _CN_216496817_220000_CN_216953915_220000/LConn1 -- _CN_216496817_220000_CN_373870139_220000/LConn1 -- _CN_216496817_220000_CN_231759891_220000/LConn1
  _CN_216498433_220000_CN_216496817_220000/RConn2 -- T_216496817_220000;66000_九州電力人吉変電所/LConn2 -- _CN_216496817_220000_CN_216953915_220000/LConn2 -- _CN_216496817_220000_CN_373870139_220000/LConn2 -- _CN_216496817_220000_CN_231759891_220000/LConn2
  _CN_216498433_220000_CN_216496817_220000/RConn3 -- T_216496817_220000;66000_九州電力人吉変電所/LConn3 -- _CN_216496817_220000_CN_216953915_220000/LConn3 -- _CN_216496817_220000_CN_373870139_220000/LConn3 -- _CN_216496817_220000_CN_231759891_220000/LConn3 -- bus9/LConn1
  T_373882198__/LConn1 -- _CN_373882198_220000_CN_218035208_220000/LConn1
  T_373882198__/LConn2 -- _CN_373882198_220000_CN_218035208_220000/LConn2
  _CN_373882198_220000_CN_218035208_220000/LConn3 -- T_373882198__/LConn3 -- bus10/LConn1
  _CN_373882198_220000_CN_218035208_220000/RConn1 -- T_218035208_220000_高野変電所/LConn1 -- _CN_218035208_220000_CN_405705606_220000/LConn1
  _CN_373882198_220000_CN_218035208_220000/RConn2 -- T_218035208_220000_高野変電所/LConn2 -- _CN_218035208_220000_CN_405705606_220000/LConn2
  _CN_373882198_220000_CN_218035208_220000/RConn3 -- T_218035208_220000_高野変電所/LConn3 -- _CN_218035208_220000_CN_405705606_220000/LConn3 -- bus11/LConn1
  T_189776902_220000;66000_九州電力_門司変電所/LConn1 -- _CN_189776902_220000_CN_296958054_220000/LConn1
  T_189776902_220000;66000_九州電力_門司変電所/LConn2 -- _CN_189776902_220000_CN_296958054_220000/LConn2
  _CN_189776902_220000_CN_296958054_220000/LConn3 -- T_189776902_220000;66000_九州電力_門司変電所/LConn3 -- bus12/LConn1
  T_296958054_220000;25000_JR西日本_新門司変電所/LConn1 -- _CN_189776902_220000_CN_296958054_220000/RConn1
  T_296958054_220000;25000_JR西日本_新門司変電所/LConn2 -- _CN_189776902_220000_CN_296958054_220000/RConn2
  _CN_189776902_220000_CN_296958054_220000/RConn3 -- T_296958054_220000;25000_JR西日本_新門司変電所/LConn3 -- bus13/LConn1
  T_405705606_220000;66000_/LConn1 -- _CN_218035208_220000_CN_405705606_220000/RConn1
  T_405705606_220000;66000_/LConn2 -- _CN_218035208_220000_CN_405705606_220000/RConn2
  _CN_218035208_220000_CN_405705606_220000/RConn3 -- T_405705606_220000;66000_/LConn3 -- bus14/LConn1
  T_239024744_220000;110000;66000_九州電力_西谷変電所/LConn1 -- _CN_239024744_220000_CN_187988970_220000/LConn1
  T_239024744_220000;110000;66000_九州電力_西谷変電所/LConn2 -- _CN_239024744_220000_CN_187988970_220000/LConn2
  _CN_239024744_220000_CN_187988970_220000/LConn3 -- T_239024744_220000;110000;66000_九州電力_西谷変電所/LConn3 -- bus15/LConn1
  _CN_239024744_220000_CN_187988970_220000/RConn1 -- T_187988970_500000;220000_/RConn1 -- _CN_187988970_220000_CN_296788490_220000/LConn1 -- L_187988970/LConn1 -- _CN_187988970_220000_CN_297939963_220000/LConn1
  _CN_239024744_220000_CN_187988970_220000/RConn2 -- T_187988970_500000;220000_/RConn2 -- _CN_187988970_220000_CN_296788490_220000/LConn2 -- L_187988970/LConn2 -- _CN_187988970_220000_CN_297939963_220000/LConn2
  _CN_239024744_220000_CN_187988970_220000/RConn3 -- T_187988970_500000;220000_/RConn3 -- _CN_187988970_220000_CN_296788490_220000/LConn3 -- L_187988970/LConn3 -- bus16/LConn1 -- _CN_187988970_220000_CN_297939963_220000/LConn3
  _CN_317951887_220000_CN_170974372_220000/LConn1 -- T_317951887_500000_/LConn1 -- _CN_317951887_220000_CN_317980483_220000/LConn1
  _CN_317951887_220000_CN_170974372_220000/LConn2 -- T_317951887_500000_/LConn2 -- _CN_317951887_220000_CN_317980483_220000/LConn2
  _CN_317951887_220000_CN_170974372_220000/LConn3 -- T_317951887_500000_/LConn3 -- _CN_317951887_220000_CN_317980483_220000/LConn3 -- bus17/LConn1
  _CN_317951887_220000_CN_170974372_220000/RConn1 -- T_170974372_220000;110000_広島変電所/LConn1 -- _CN_170974372_220000_CN_193544791_220000/LConn1
  _CN_317951887_220000_CN_170974372_220000/RConn2 -- T_170974372_220000;110000_広島変電所/LConn2 -- _CN_170974372_220000_CN_193544791_220000/LConn2
  _CN_317951887_220000_CN_170974372_220000/RConn3 -- T_170974372_220000;110000_広島変電所/LConn3 -- _CN_170974372_220000_CN_193544791_220000/LConn3 -- bus18/LConn1
  T_317980483_220000_/LConn1 -- _CN_317951887_220000_CN_317980483_220000/RConn1
  T_317980483_220000_/LConn2 -- _CN_317951887_220000_CN_317980483_220000/RConn2
  _CN_317951887_220000_CN_317980483_220000/RConn3 -- T_317980483_220000_/LConn3 -- bus19/LConn1
  T_319463514_220000;110000_下松発電所/LConn1 -- _CN_319463514_220000_CN_243471278_220000/LConn1
  T_319463514_220000;110000_下松発電所/LConn2 -- _CN_319463514_220000_CN_243471278_220000/LConn2
  _CN_319463514_220000_CN_243471278_220000/LConn3 -- T_319463514_220000;110000_下松発電所/LConn3 -- bus20/LConn1
  _CN_319463514_220000_CN_243471278_220000/RConn1 -- T_243471278_220000_/LConn1 -- _CN_243471278_220000_CN_193544791_220000/LConn1 -- _CN_243471278_220000_CN_242253500_220000/LConn1 -- _CN_243471278_220000_CN_319371122_220000/LConn1 -- _CN_243471278_220000_CN_318438125_220000/LConn1
  _CN_319463514_220000_CN_243471278_220000/RConn2 -- T_243471278_220000_/LConn2 -- _CN_243471278_220000_CN_193544791_220000/LConn2 -- _CN_243471278_220000_CN_242253500_220000/LConn2 -- _CN_243471278_220000_CN_319371122_220000/LConn2 -- _CN_243471278_220000_CN_318438125_220000/LConn2
  _CN_319463514_220000_CN_243471278_220000/RConn3 -- T_243471278_220000_/LConn3 -- _CN_243471278_220000_CN_193544791_220000/LConn3 -- _CN_243471278_220000_CN_242253500_220000/LConn3 -- bus21/LConn1 -- _CN_243471278_220000_CN_319371122_220000/LConn3 -- _CN_243471278_220000_CN_318438125_220000/LConn3
  _CN_215451416_220000_CN_406052986_220000/LConn1 -- T_215451416_500000;220000_九州電力南九州変電所/RConn1 -- L_215451416/LConn1
  _CN_215451416_220000_CN_406052986_220000/LConn2 -- T_215451416_500000;220000_九州電力南九州変電所/RConn2 -- L_215451416/LConn2
  _CN_215451416_220000_CN_406052986_220000/LConn3 -- T_215451416_500000;220000_九州電力南九州変電所/RConn3 -- L_215451416/LConn3 -- bus22/LConn1
  T_406052986_220000_/LConn1 -- _CN_215451416_220000_CN_406052986_220000/RConn1
  T_406052986_220000_/LConn2 -- _CN_215451416_220000_CN_406052986_220000/RConn2
  _CN_215451416_220000_CN_406052986_220000/RConn3 -- T_406052986_220000_/LConn3 -- bus23/LConn1
  _CN_241822623_220000_CN_242159178_220000/LConn1 -- T_241822623_500000;220000;110000_/RConn1 -- L_241822623/LConn1
  _CN_241822623_220000_CN_242159178_220000/LConn2 -- T_241822623_500000;220000;110000_/RConn2 -- L_241822623/LConn2
  _CN_241822623_220000_CN_242159178_220000/LConn3 -- T_241822623_500000;220000;110000_/RConn3 -- L_241822623/LConn3 -- bus24/LConn1
  _CN_241822623_220000_CN_242159178_220000/RConn1 -- T_242159178_220000_/LConn1 -- _CN_242159178_220000_CN_241828221_220000/LConn1
  _CN_241822623_220000_CN_242159178_220000/RConn2 -- T_242159178_220000_/LConn2 -- _CN_242159178_220000_CN_241828221_220000/LConn2
  _CN_241822623_220000_CN_242159178_220000/RConn3 -- T_242159178_220000_/LConn3 -- _CN_242159178_220000_CN_241828221_220000/LConn3 -- bus25/LConn1
  _CN_170974372_220000_CN_193544791_220000/RConn1 -- T_193544791_500000_新西広島変電所_(Shin_Nishi_Hiroshima_Hendensho)/RConn1 -- _CN_243471278_220000_CN_193544791_220000/RConn1 -- L_193544791/LConn1
  _CN_170974372_220000_CN_193544791_220000/RConn2 -- T_193544791_500000_新西広島変電所_(Shin_Nishi_Hiroshima_Hendensho)/RConn2 -- _CN_243471278_220000_CN_193544791_220000/RConn2 -- L_193544791/LConn2
  _CN_170974372_220000_CN_193544791_220000/RConn3 -- T_193544791_500000_新西広島変電所_(Shin_Nishi_Hiroshima_Hendensho)/RConn3 -- _CN_243471278_220000_CN_193544791_220000/RConn3 -- L_193544791/LConn3 -- bus26/LConn1
  _CN_216496817_220000_CN_216953915_220000/RConn1 -- G_216953915_/RConn1 -- 小丸川幹線_CN_216956620_500000_CN_216953915_220000/LConn1
  _CN_216496817_220000_CN_216953915_220000/RConn2 -- G_216953915_/RConn2 -- 小丸川幹線_CN_216956620_500000_CN_216953915_220000/LConn2
  _CN_216496817_220000_CN_216953915_220000/RConn3 -- G_216953915_/RConn3 -- 小丸川幹線_CN_216956620_500000_CN_216953915_220000/LConn3 -- bus27/LConn1
  T_373870139__/LConn1 -- _CN_216496817_220000_CN_373870139_220000/RConn1
  T_373870139__/LConn2 -- _CN_216496817_220000_CN_373870139_220000/RConn2
  _CN_216496817_220000_CN_373870139_220000/RConn3 -- T_373870139__/LConn3 -- bus28/LConn1
  G_231759891_一ツ瀬水力発電所/RConn1 -- _CN_216496817_220000_CN_231759891_220000/RConn1
  G_231759891_一ツ瀬水力発電所/RConn2 -- _CN_216496817_220000_CN_231759891_220000/RConn2
  _CN_216496817_220000_CN_231759891_220000/RConn3 -- G_231759891_一ツ瀬水力発電所/RConn3 -- bus29/LConn1
  T_173152424_220000;66000_九州電力_西福岡変電所/LConn1 -- _CN_173152424_220000_CN_172601929_220000/LConn1
  T_173152424_220000;66000_九州電力_西福岡変電所/LConn2 -- _CN_173152424_220000_CN_172601929_220000/LConn2
  _CN_173152424_220000_CN_172601929_220000/LConn3 -- T_173152424_220000;66000_九州電力_西福岡変電所/LConn3 -- bus30/LConn1
  _CN_173152424_220000_CN_172601929_220000/RConn1 -- T_172601929_500000;220000_/RConn1 -- 脊振鳥栖線_CN_172601929_220000_CN_174915836_220000/LConn1 -- 脊振鳥栖線_CN_172601929_220000_CN_173793392_220000/LConn1 -- L_172601929/LConn1
  _CN_173152424_220000_CN_172601929_220000/RConn2 -- T_172601929_500000;220000_/RConn2 -- 脊振鳥栖線_CN_172601929_220000_CN_174915836_220000/LConn2 -- 脊振鳥栖線_CN_172601929_220000_CN_173793392_220000/LConn2 -- L_172601929/LConn2
  _CN_173152424_220000_CN_172601929_220000/RConn3 -- T_172601929_500000;220000_/RConn3 -- 脊振鳥栖線_CN_172601929_220000_CN_174915836_220000/LConn3 -- 脊振鳥栖線_CN_172601929_220000_CN_173793392_220000/LConn3 -- L_172601929/LConn3 -- bus31/LConn1
  T_238089516_220000_九州新幹線_新鳥栖変電所/LConn1 -- _CN_238089516_220000_CN_173793392_220000/LConn1
  T_238089516_220000_九州新幹線_新鳥栖変電所/LConn2 -- _CN_238089516_220000_CN_173793392_220000/LConn2
  _CN_238089516_220000_CN_173793392_220000/LConn3 -- T_238089516_220000_九州新幹線_新鳥栖変電所/LConn3 -- bus32/LConn1
  _CN_238089516_220000_CN_173793392_220000/RConn1 -- T_173793392__鳥栖変電所/LConn1 -- 脊振鳥栖線_CN_172601929_220000_CN_173793392_220000/RConn1
  _CN_238089516_220000_CN_173793392_220000/RConn2 -- T_173793392__鳥栖変電所/LConn2 -- 脊振鳥栖線_CN_172601929_220000_CN_173793392_220000/RConn2
  _CN_238089516_220000_CN_173793392_220000/RConn3 -- T_173793392__鳥栖変電所/LConn3 -- 脊振鳥栖線_CN_172601929_220000_CN_173793392_220000/RConn3 -- bus33/LConn1
  T_319371122_220000_/LConn1 -- _CN_243471278_220000_CN_319371122_220000/RConn1
  T_319371122_220000_/LConn2 -- _CN_243471278_220000_CN_319371122_220000/RConn2
  _CN_243471278_220000_CN_319371122_220000/RConn3 -- T_319371122_220000_/LConn3 -- bus34/LConn1
  _CN_243471278_220000_CN_318438125_220000/RConn1 -- T_318438125_220000_/LConn1 -- _CN_204258596_220000_CN_318438125_220000/LConn1
  _CN_243471278_220000_CN_318438125_220000/RConn2 -- T_318438125_220000_/LConn2 -- _CN_204258596_220000_CN_318438125_220000/LConn2
  _CN_243471278_220000_CN_318438125_220000/RConn3 -- T_318438125_220000_/LConn3 -- _CN_204258596_220000_CN_318438125_220000/LConn3 -- bus35/LConn1
  _CN_243471278_220000_CN_242253500_220000/RConn1 -- T_242253500_500000_東山口変電所_(Higashi_Yamaguchi_Hendensho)/RConn1 -- L_242253500/LConn1
  _CN_243471278_220000_CN_242253500_220000/RConn2 -- T_242253500_500000_東山口変電所_(Higashi_Yamaguchi_Hendensho)/RConn2 -- L_242253500/LConn2
  _CN_243471278_220000_CN_242253500_220000/RConn3 -- T_242253500_500000_東山口変電所_(Higashi_Yamaguchi_Hendensho)/RConn3 -- L_242253500/LConn3 -- bus36/LConn1
  T_172143432__/LConn1 -- _CN_172143432_220000_CN_184180157_220000/LConn1
  T_172143432__/LConn2 -- _CN_172143432_220000_CN_184180157_220000/LConn2
  _CN_172143432_220000_CN_184180157_220000/LConn3 -- T_172143432__/LConn3 -- bus37/LConn1
  T_184180157_220000;66000_東福岡変電所/LConn1 -- _CN_172143432_220000_CN_184180157_220000/RConn1
  T_184180157_220000;66000_東福岡変電所/LConn2 -- _CN_172143432_220000_CN_184180157_220000/RConn2
  _CN_172143432_220000_CN_184180157_220000/RConn3 -- T_184180157_220000;66000_東福岡変電所/LConn3 -- bus38/LConn1
  T_405806514_220000;66000_/LConn1 -- _CN_405806514_220000_CN_216809817_220000/RConn1
  T_405806514_220000;66000_/LConn2 -- _CN_405806514_220000_CN_216809817_220000/RConn2
  _CN_405806514_220000_CN_216809817_220000/RConn3 -- T_405806514_220000;66000_/LConn3 -- bus39/LConn1
  T_189777972__/LConn1 -- _CN_189777972_220000_CN_296789326_220000/LConn1
  T_189777972__/LConn2 -- _CN_189777972_220000_CN_296789326_220000/LConn2
  _CN_189777972_220000_CN_296789326_220000/LConn3 -- T_189777972__/LConn3 -- bus40/LConn1
  T_296789326__/LConn1 -- _CN_189777972_220000_CN_296789326_220000/RConn1
  T_296789326__/LConn2 -- _CN_189777972_220000_CN_296789326_220000/RConn2
  _CN_189777972_220000_CN_296789326_220000/RConn3 -- T_296789326__/LConn3 -- bus41/LConn1
  T_201289289_220000_九州電力_唐津変電所/LConn1 -- 唐津西九州線_CN_201289289_220000_CN_185029969_220000/LConn1
  T_201289289_220000_九州電力_唐津変電所/LConn2 -- 唐津西九州線_CN_201289289_220000_CN_185029969_220000/LConn2
  唐津西九州線_CN_201289289_220000_CN_185029969_220000/LConn3 -- T_201289289_220000_九州電力_唐津変電所/LConn3 -- bus42/LConn1
  唐津西九州線_CN_201289289_220000_CN_185029969_220000/RConn1 -- T_185029969_500000;220000_/RConn1 -- _CN_185029969_220000_CN_185504478_220000/LConn1 -- _CN_185029969_220000_CN_172644773_220000/LConn1 -- L_185029969/LConn1
  唐津西九州線_CN_201289289_220000_CN_185029969_220000/RConn2 -- T_185029969_500000;220000_/RConn2 -- _CN_185029969_220000_CN_185504478_220000/LConn2 -- _CN_185029969_220000_CN_172644773_220000/LConn2 -- L_185029969/LConn2
  唐津西九州線_CN_201289289_220000_CN_185029969_220000/RConn3 -- T_185029969_500000;220000_/RConn3 -- _CN_185029969_220000_CN_185504478_220000/LConn3 -- _CN_185029969_220000_CN_172644773_220000/LConn3 -- L_185029969/LConn3 -- bus43/LConn1
  _CN_203776442_220000_CN_174915836_220000/RConn1 -- T_174915836_220000;66000_九州電力_木佐木変電所/LConn1 -- 脊振鳥栖線_CN_172601929_220000_CN_174915836_220000/RConn1 -- _CN_185504478_220000_CN_174915836_220000/LConn1
  _CN_203776442_220000_CN_174915836_220000/RConn2 -- T_174915836_220000;66000_九州電力_木佐木変電所/LConn2 -- 脊振鳥栖線_CN_172601929_220000_CN_174915836_220000/RConn2 -- _CN_185504478_220000_CN_174915836_220000/LConn2
  _CN_203776442_220000_CN_174915836_220000/RConn3 -- T_174915836_220000;66000_九州電力_木佐木変電所/LConn3 -- 脊振鳥栖線_CN_172601929_220000_CN_174915836_220000/RConn3 -- _CN_185504478_220000_CN_174915836_220000/LConn3 -- bus44/LConn1
  _CN_90806466_220000_CN_216949339_220000/RConn1 -- T_216949339_220000;110000;66000_/LConn1 -- _CN_216949339_220000_CN_216781917_220000/LConn1
  _CN_90806466_220000_CN_216949339_220000/RConn2 -- T_216949339_220000;110000;66000_/LConn2 -- _CN_216949339_220000_CN_216781917_220000/LConn2
  _CN_90806466_220000_CN_216949339_220000/RConn3 -- T_216949339_220000;110000;66000_/LConn3 -- _CN_216949339_220000_CN_216781917_220000/LConn3 -- bus45/LConn1
  T_186510275_500000_3_4号_開閉所/LConn1 -- 予備電源線_CN_186510275_220000_CN_172644773_220000/LConn1
  T_186510275_500000_3_4号_開閉所/LConn2 -- 予備電源線_CN_186510275_220000_CN_172644773_220000/LConn2
  予備電源線_CN_186510275_220000_CN_172644773_220000/LConn3 -- T_186510275_500000_3_4号_開閉所/LConn3 -- bus46/LConn1
  予備電源線_CN_186510275_220000_CN_172644773_220000/RConn1 -- G_172644773_玄海原子力発電所/RConn1 -- _CN_172601929_500000_CN_172644773_220000/LConn1 -- _CN_185029969_220000_CN_172644773_220000/RConn1
  予備電源線_CN_186510275_220000_CN_172644773_220000/RConn2 -- G_172644773_玄海原子力発電所/RConn2 -- _CN_172601929_500000_CN_172644773_220000/LConn2 -- _CN_185029969_220000_CN_172644773_220000/RConn2
  予備電源線_CN_186510275_220000_CN_172644773_220000/RConn3 -- G_172644773_玄海原子力発電所/RConn3 -- _CN_172601929_500000_CN_172644773_220000/LConn3 -- bus47/LConn1 -- _CN_185029969_220000_CN_172644773_220000/RConn3
  _CN_242159178_220000_CN_241828221_220000/RConn1 -- T_241828221_500000_新岡山変電所_(Shin_Okayama_Hendensho)/RConn1 -- _CN_242389846_220000_CN_241828221_220000/LConn1 -- L_241828221/LConn1
  _CN_242159178_220000_CN_241828221_220000/RConn2 -- T_241828221_500000_新岡山変電所_(Shin_Okayama_Hendensho)/RConn2 -- _CN_242389846_220000_CN_241828221_220000/LConn2 -- L_241828221/LConn2
  _CN_242159178_220000_CN_241828221_220000/RConn3 -- T_241828221_500000_新岡山変電所_(Shin_Okayama_Hendensho)/RConn3 -- _CN_242389846_220000_CN_241828221_220000/LConn3 -- L_241828221/LConn3 -- bus48/LConn1
  _CN_220698807_220000_CN_219579624_220000/LConn1 -- T_220698807__/LConn1 -- _CN_220698807_220000_CN_241875111_220000/LConn1
  _CN_220698807_220000_CN_219579624_220000/LConn2 -- T_220698807__/LConn2 -- _CN_220698807_220000_CN_241875111_220000/LConn2
  _CN_220698807_220000_CN_219579624_220000/LConn3 -- T_220698807__/LConn3 -- _CN_220698807_220000_CN_241875111_220000/LConn3 -- bus49/LConn1
  T_219579624_220000_/LConn1 -- _CN_220698807_220000_CN_219579624_220000/RConn1
  T_219579624_220000_/LConn2 -- _CN_220698807_220000_CN_219579624_220000/RConn2
  _CN_220698807_220000_CN_219579624_220000/RConn3 -- T_219579624_220000_/LConn3 -- bus50/LConn1
  T_241875111_220000_/LConn1 -- _CN_220698807_220000_CN_241875111_220000/RConn1
  T_241875111_220000_/LConn2 -- _CN_220698807_220000_CN_241875111_220000/RConn2
  _CN_220698807_220000_CN_241875111_220000/RConn3 -- T_241875111_220000_/LConn3 -- bus51/LConn1
  _CN_185029969_220000_CN_185504478_220000/RConn1 -- T_185504478_220000;66000_/LConn1 -- _CN_185504478_220000_CN_174915836_220000/RConn1
  _CN_185029969_220000_CN_185504478_220000/RConn2 -- T_185504478_220000;66000_/LConn2 -- _CN_185504478_220000_CN_174915836_220000/RConn2
  _CN_185029969_220000_CN_185504478_220000/RConn3 -- T_185504478_220000;66000_/LConn3 -- _CN_185504478_220000_CN_174915836_220000/RConn3 -- bus52/LConn1
  T_242389846__/LConn1 -- _CN_242389846_220000_CN_241828221_220000/RConn1
  T_242389846__/LConn2 -- _CN_242389846_220000_CN_241828221_220000/RConn2
  _CN_242389846_220000_CN_241828221_220000/RConn3 -- T_242389846__/LConn3 -- bus53/LConn1
  _CN_204258596_220000_CN_318438125_220000/RConn1 -- T_204258596_500000_/RConn1 -- L_204258596/LConn1
  _CN_204258596_220000_CN_318438125_220000/RConn2 -- T_204258596_500000_/RConn2 -- L_204258596/LConn2
  _CN_204258596_220000_CN_318438125_220000/RConn3 -- T_204258596_500000_/RConn3 -- L_204258596/LConn3 -- bus54/LConn1
  G_216781917_新大分火力発電所/RConn1 -- _CN_216949339_220000_CN_216781917_220000/RConn1
  G_216781917_新大分火力発電所/RConn2 -- _CN_216949339_220000_CN_216781917_220000/RConn2
  _CN_216949339_220000_CN_216781917_220000/RConn3 -- G_216781917_新大分火力発電所/RConn3 -- bus55/LConn1
  T_172144358_500000;220000_/LConn1 -- _CN_172144358_220000_CN_172144359_220000/LConn1
  T_172144358_500000;220000_/LConn2 -- _CN_172144358_220000_CN_172144359_220000/LConn2
  _CN_172144358_220000_CN_172144359_220000/LConn3 -- T_172144358_500000;220000_/LConn3 -- bus56/LConn1
  T_172144359_500000;220000_/LConn1 -- _CN_172144358_220000_CN_172144359_220000/RConn1
  T_172144359_500000;220000_/LConn2 -- _CN_172144358_220000_CN_172144359_220000/RConn2
  _CN_172144358_220000_CN_172144359_220000/RConn3 -- T_172144359_500000;220000_/LConn3 -- bus57/LConn1
  T_297939963_220000_/LConn1 -- _CN_187988970_220000_CN_297939963_220000/RConn1
  T_297939963_220000_/LConn2 -- _CN_187988970_220000_CN_297939963_220000/RConn2
  _CN_187988970_220000_CN_297939963_220000/RConn3 -- T_297939963_220000_/LConn3 -- bus58/LConn1
  T_296788490_220000;66000_九州電力_上津役変電所/LConn1 -- _CN_187988970_220000_CN_296788490_220000/RConn1
  T_296788490_220000;66000_九州電力_上津役変電所/LConn2 -- _CN_187988970_220000_CN_296788490_220000/RConn2
  _CN_187988970_220000_CN_296788490_220000/RConn3 -- T_296788490_220000;66000_九州電力_上津役変電所/LConn3 -- bus59/LConn1
  _CN_238813045_220000_CN_238813048_220000/LConn1 -- T_238813045_220000_/LConn1 -- _CN_238813045_220000_CN_365487155_220000/LConn1
  _CN_238813045_220000_CN_238813048_220000/LConn2 -- T_238813045_220000_/LConn2 -- _CN_238813045_220000_CN_365487155_220000/LConn2
  _CN_238813045_220000_CN_238813048_220000/LConn3 -- T_238813045_220000_/LConn3 -- _CN_238813045_220000_CN_365487155_220000/LConn3 -- bus60/LConn1
  T_238813048_220000_出水変電所/LConn1 -- _CN_238813045_220000_CN_238813048_220000/RConn1
  T_238813048_220000_出水変電所/LConn2 -- _CN_238813045_220000_CN_238813048_220000/RConn2
  _CN_238813045_220000_CN_238813048_220000/RConn3 -- T_238813048_220000_出水変電所/LConn3 -- bus61/LConn1
  _CN_238813045_220000_CN_365487155_220000/RConn1 -- G_365487155_川内発電所/RConn1 -- _CN_237475191_220000_CN_365487155_220000/LConn1
  _CN_238813045_220000_CN_365487155_220000/RConn2 -- G_365487155_川内発電所/RConn2 -- _CN_237475191_220000_CN_365487155_220000/LConn2
  _CN_238813045_220000_CN_365487155_220000/RConn3 -- G_365487155_川内発電所/RConn3 -- _CN_237475191_220000_CN_365487155_220000/LConn3 -- bus62/LConn1
  _CN_237475191_220000_CN_365487155_220000/RConn1 -- T_237475191_220000_九州電力_新鹿児島変電所/LConn1 -- _CN_237475191_220000_CN_215429864_220000/LConn1
  _CN_237475191_220000_CN_365487155_220000/RConn2 -- T_237475191_220000_九州電力_新鹿児島変電所/LConn2 -- _CN_237475191_220000_CN_215429864_220000/LConn2
  _CN_237475191_220000_CN_365487155_220000/RConn3 -- T_237475191_220000_九州電力_新鹿児島変電所/LConn3 -- _CN_237475191_220000_CN_215429864_220000/LConn3 -- bus63/LConn1
  _CN_237475191_220000_CN_215429864_220000/RConn1 -- G_215429864_川内原子力発電所/RConn1 -- _CN_215451416_500000_CN_215429864_220000/LConn1
  _CN_237475191_220000_CN_215429864_220000/RConn2 -- G_215429864_川内原子力発電所/RConn2 -- _CN_215451416_500000_CN_215429864_220000/LConn2
  _CN_237475191_220000_CN_215429864_220000/RConn3 -- G_215429864_川内原子力発電所/RConn3 -- _CN_215451416_500000_CN_215429864_220000/LConn3 -- bus64/LConn1
  _CN_169121281_275000_CN_169121284_275000/LConn1 -- T_169121281__北豊田変電所_(Kita_Toyota_Hendensho)/LConn1 -- _CN_169121281_275000_CN_169122898_275000/LConn1
  _CN_169121281_275000_CN_169121284_275000/LConn2 -- T_169121281__北豊田変電所_(Kita_Toyota_Hendensho)/LConn2 -- _CN_169121281_275000_CN_169122898_275000/LConn2
  _CN_169121281_275000_CN_169121284_275000/LConn3 -- T_169121281__北豊田変電所_(Kita_Toyota_Hendensho)/LConn3 -- _CN_169121281_275000_CN_169122898_275000/LConn3 -- bus65/LConn1
  _CN_169121281_275000_CN_169121284_275000/RConn1 -- T_169121284_275000_/LConn1 -- _CN_169121284_275000_CN_170850727_275000/LConn1 -- _CN_169121284_275000_CN_169121278_275000/LConn1
  _CN_169121281_275000_CN_169121284_275000/RConn2 -- T_169121284_275000_/LConn2 -- _CN_169121284_275000_CN_170850727_275000/LConn2 -- _CN_169121284_275000_CN_169121278_275000/LConn2
  _CN_169121281_275000_CN_169121284_275000/RConn3 -- T_169121284_275000_/LConn3 -- _CN_169121284_275000_CN_170850727_275000/LConn3 -- bus66/LConn1 -- _CN_169121284_275000_CN_169121278_275000/LConn3
  _CN_169121281_275000_CN_169122898_275000/RConn1 -- T_169122898_500000_東部変電所/RConn1 -- _CN_169122898_275000_CN_179417733_275000/LConn1 -- L_169122898/LConn1 -- _CN_169122898_275000_CN_134376414_275000/LConn1 -- _CN_169122898_275000_CN_170850727_275000/LConn1 -- _CN_169122898_275000_CN_170247359_275000/LConn1
  _CN_169121281_275000_CN_169122898_275000/RConn2 -- T_169122898_500000_東部変電所/RConn2 -- _CN_169122898_275000_CN_179417733_275000/LConn2 -- L_169122898/LConn2 -- _CN_169122898_275000_CN_134376414_275000/LConn2 -- _CN_169122898_275000_CN_170850727_275000/LConn2 -- _CN_169122898_275000_CN_170247359_275000/LConn2
  _CN_169121281_275000_CN_169122898_275000/RConn3 -- T_169122898_500000_東部変電所/RConn3 -- _CN_169122898_275000_CN_179417733_275000/LConn3 -- L_169122898/LConn3 -- bus67/LConn1 -- _CN_169122898_275000_CN_134376414_275000/LConn3 -- _CN_169122898_275000_CN_170850727_275000/LConn3 -- _CN_169122898_275000_CN_170247359_275000/LConn3
  佐久間東幹線_CN_116828675_275000_CN_150065045_275000/LConn1 -- T_116828675_275000_北相模変電所_(Kita_Sagami_Hendensho)/LConn1 -- 佐久間東幹線_CN_116828675_275000_CN_134376414_275000/LConn1
  佐久間東幹線_CN_116828675_275000_CN_150065045_275000/LConn2 -- T_116828675_275000_北相模変電所_(Kita_Sagami_Hendensho)/LConn2 -- 佐久間東幹線_CN_116828675_275000_CN_134376414_275000/LConn2
  佐久間東幹線_CN_116828675_275000_CN_150065045_275000/LConn3 -- T_116828675_275000_北相模変電所_(Kita_Sagami_Hendensho)/LConn3 -- 佐久間東幹線_CN_116828675_275000_CN_134376414_275000/LConn3 -- bus68/LConn1
  佐久間東幹線_CN_116828675_275000_CN_150065045_275000/RConn1 -- T_150065045_500000_新富士変電所/RConn1 -- L_150065045/LConn1
  佐久間東幹線_CN_116828675_275000_CN_150065045_275000/RConn2 -- T_150065045_500000_新富士変電所/RConn2 -- L_150065045/LConn2
  佐久間東幹線_CN_116828675_275000_CN_150065045_275000/RConn3 -- T_150065045_500000_新富士変電所/RConn3 -- L_150065045/LConn3 -- bus69/LConn1
  佐久間東幹線_CN_116828675_275000_CN_134376414_275000/RConn1 -- G_134376414_佐久間発電所/RConn1 -- _CN_169122898_275000_CN_134376414_275000/RConn1
  佐久間東幹線_CN_116828675_275000_CN_134376414_275000/RConn2 -- G_134376414_佐久間発電所/RConn2 -- _CN_169122898_275000_CN_134376414_275000/RConn2
  佐久間東幹線_CN_116828675_275000_CN_134376414_275000/RConn3 -- G_134376414_佐久間発電所/RConn3 -- _CN_169122898_275000_CN_134376414_275000/RConn3 -- bus70/LConn1
  _CN_169121284_275000_CN_169121278_275000/RConn1 -- T_169121278_275000_電源名古屋/LConn1 -- _CN_170366038_275000_CN_169121278_275000/LConn1
  _CN_169121284_275000_CN_169121278_275000/RConn2 -- T_169121278_275000_電源名古屋/LConn2 -- _CN_170366038_275000_CN_169121278_275000/LConn2
  _CN_169121284_275000_CN_169121278_275000/RConn3 -- T_169121278_275000_電源名古屋/LConn3 -- _CN_170366038_275000_CN_169121278_275000/LConn3 -- bus71/LConn1
  _CN_169121284_275000_CN_170850727_275000/RConn1 -- T_170850727_500000_愛知変電所/RConn1 -- _CN_169122898_275000_CN_170850727_275000/RConn1 -- L_170850727/LConn1
  _CN_169121284_275000_CN_170850727_275000/RConn2 -- T_170850727_500000_愛知変電所/RConn2 -- _CN_169122898_275000_CN_170850727_275000/RConn2 -- L_170850727/LConn2
  _CN_169121284_275000_CN_170850727_275000/RConn3 -- T_170850727_500000_愛知変電所/RConn3 -- _CN_169122898_275000_CN_170850727_275000/RConn3 -- L_170850727/LConn3 -- bus72/LConn1
  _CN_170503689_275000_CN_170436908_275000/LConn1 -- T_170503689__駿遠変電所/LConn1 -- _CN_170503689_275000_CN_210090094_275000/LConn1
  _CN_170503689_275000_CN_170436908_275000/LConn2 -- T_170503689__駿遠変電所/LConn2 -- _CN_170503689_275000_CN_210090094_275000/LConn2
  _CN_170503689_275000_CN_170436908_275000/LConn3 -- T_170503689__駿遠変電所/LConn3 -- _CN_170503689_275000_CN_210090094_275000/LConn3 -- bus73/LConn1
  T_170436908__/LConn1 -- _CN_170503689_275000_CN_170436908_275000/RConn1
  T_170436908__/LConn2 -- _CN_170503689_275000_CN_170436908_275000/RConn2
  _CN_170503689_275000_CN_170436908_275000/RConn3 -- T_170436908__/LConn3 -- bus74/LConn1
  _CN_170503689_275000_CN_210090094_275000/RConn1 -- T_210090094_500000_駿遠変電所/RConn1 -- 三河遠江線_CN_170366039_275000_CN_210090094_275000/LConn1 -- L_210090094/LConn1
  _CN_170503689_275000_CN_210090094_275000/RConn2 -- T_210090094_500000_駿遠変電所/RConn2 -- 三河遠江線_CN_170366039_275000_CN_210090094_275000/LConn2 -- L_210090094/LConn2
  _CN_170503689_275000_CN_210090094_275000/RConn3 -- T_210090094_500000_駿遠変電所/RConn3 -- 三河遠江線_CN_170366039_275000_CN_210090094_275000/LConn3 -- L_210090094/LConn3 -- bus75/LConn1
  _CN_158064651_275000_CN_232998815_275000/LConn1 -- T_158064651_275000_田子倉発電所/LConn1 -- _CN_158064651_275000_CN_319098734_275000/LConn1
  _CN_158064651_275000_CN_232998815_275000/LConn2 -- T_158064651_275000_田子倉発電所/LConn2 -- _CN_158064651_275000_CN_319098734_275000/LConn2
  _CN_158064651_275000_CN_232998815_275000/LConn3 -- T_158064651_275000_田子倉発電所/LConn3 -- _CN_158064651_275000_CN_319098734_275000/LConn3 -- bus76/LConn1
  _CN_158064651_275000_CN_232998815_275000/RConn1 -- T_232998815_275000_/LConn1 -- _CN_232998815_275000_CN_233174201_275000/LConn1 -- 奥只見線_CN_250540807_275000_CN_232998815_275000/LConn1
  _CN_158064651_275000_CN_232998815_275000/RConn2 -- T_232998815_275000_/LConn2 -- _CN_232998815_275000_CN_233174201_275000/LConn2 -- 奥只見線_CN_250540807_275000_CN_232998815_275000/LConn2
  _CN_158064651_275000_CN_232998815_275000/RConn3 -- T_232998815_275000_/LConn3 -- _CN_232998815_275000_CN_233174201_275000/LConn3 -- bus77/LConn1 -- 奥只見線_CN_250540807_275000_CN_232998815_275000/LConn3
  _CN_158064651_275000_CN_319098734_275000/RConn1 -- G_319098734_信濃川水力発電所/RConn1 -- _CN_318302348_275000_CN_319098734_275000/LConn1
  _CN_158064651_275000_CN_319098734_275000/RConn2 -- G_319098734_信濃川水力発電所/RConn2 -- _CN_318302348_275000_CN_319098734_275000/LConn2
  _CN_158064651_275000_CN_319098734_275000/RConn3 -- G_319098734_信濃川水力発電所/RConn3 -- _CN_318302348_275000_CN_319098734_275000/LConn3 -- bus78/LConn1
  伊勢幹線_CN_241956440_275000_CN_170537514_275000/LConn1 -- T_241956440_275000_伊勢開閉所/LConn1 -- _CN_241956440_275000_CN_241923317_275000/LConn1 -- _CN_241956440_275000_CN_214992492_275000/LConn1 -- _CN_241956440_275000_CN_242532736_275000/LConn1
  伊勢幹線_CN_241956440_275000_CN_170537514_275000/LConn2 -- T_241956440_275000_伊勢開閉所/LConn2 -- _CN_241956440_275000_CN_241923317_275000/LConn2 -- _CN_241956440_275000_CN_214992492_275000/LConn2 -- _CN_241956440_275000_CN_242532736_275000/LConn2
  伊勢幹線_CN_241956440_275000_CN_170537514_275000/LConn3 -- T_241956440_275000_伊勢開閉所/LConn3 -- _CN_241956440_275000_CN_241923317_275000/LConn3 -- _CN_241956440_275000_CN_214992492_275000/LConn3 -- _CN_241956440_275000_CN_242532736_275000/LConn3 -- bus79/LConn1
  伊勢幹線_CN_241956440_275000_CN_170537514_275000/RConn1 -- T_170537514_500000_/RConn1 -- _CN_170537514_275000_CN_170793702_275000/LConn1 -- _CN_170537514_275000_CN_170793703_275000/LConn1 -- L_170537514/LConn1 -- 西部西濃線_(Seibu_Seinō_Sen)_CN_170537514_275000_CN_161948515_275000/LConn1
  伊勢幹線_CN_241956440_275000_CN_170537514_275000/RConn2 -- T_170537514_500000_/RConn2 -- _CN_170537514_275000_CN_170793702_275000/LConn2 -- _CN_170537514_275000_CN_170793703_275000/LConn2 -- L_170537514/LConn2 -- 西部西濃線_(Seibu_Seinō_Sen)_CN_170537514_275000_CN_161948515_275000/LConn2
  伊勢幹線_CN_241956440_275000_CN_170537514_275000/RConn3 -- T_170537514_500000_/RConn3 -- _CN_170537514_275000_CN_170793702_275000/LConn3 -- _CN_170537514_275000_CN_170793703_275000/LConn3 -- L_170537514/LConn3 -- bus80/LConn1 -- 西部西濃線_(Seibu_Seinō_Sen)_CN_170537514_275000_CN_161948515_275000/LConn3
  T_241923317_275000_南勢変電所_(Nansei_Hendensho)/LConn1 -- _CN_241956440_275000_CN_241923317_275000/RConn1
  T_241923317_275000_南勢変電所_(Nansei_Hendensho)/LConn2 -- _CN_241956440_275000_CN_241923317_275000/RConn2
  _CN_241956440_275000_CN_241923317_275000/RConn3 -- T_241923317_275000_南勢変電所_(Nansei_Hendensho)/LConn3 -- bus81/LConn1
  G_214992492_/RConn1 -- _CN_241956440_275000_CN_214992492_275000/RConn1
  G_214992492_/RConn2 -- _CN_241956440_275000_CN_214992492_275000/RConn2
  _CN_241956440_275000_CN_214992492_275000/RConn3 -- G_214992492_/RConn3 -- bus82/LConn1
  T_242532736_275000_/LConn1 -- _CN_241956440_275000_CN_242532736_275000/RConn1
  T_242532736_275000_/LConn2 -- _CN_241956440_275000_CN_242532736_275000/RConn2
  _CN_241956440_275000_CN_242532736_275000/RConn3 -- T_242532736_275000_/LConn3 -- bus83/LConn1
  T_162844704_275000_中相模変電所/LConn1 -- 秦浜線_CN_162844704_275000_CN_128364781_275000/LConn1
  T_162844704_275000_中相模変電所/LConn2 -- 秦浜線_CN_162844704_275000_CN_128364781_275000/LConn2
  秦浜線_CN_162844704_275000_CN_128364781_275000/LConn3 -- T_162844704_275000_中相模変電所/LConn3 -- bus84/LConn1
  秦浜線_CN_162844704_275000_CN_128364781_275000/RConn1 -- T_128364781_275000_東京電力_京浜変電所/LConn1 -- 京浜線3;4号線_CN_128364781_275000_CN_47110637_275000/LConn1 -- 東京南線3;4号線_CN_128364781_275000_CN_379474501_275000/LConn1
  秦浜線_CN_162844704_275000_CN_128364781_275000/RConn2 -- T_128364781_275000_東京電力_京浜変電所/LConn2 -- 京浜線3;4号線_CN_128364781_275000_CN_47110637_275000/LConn2 -- 東京南線3;4号線_CN_128364781_275000_CN_379474501_275000/LConn2
  秦浜線_CN_162844704_275000_CN_128364781_275000/RConn3 -- T_128364781_275000_東京電力_京浜変電所/LConn3 -- 京浜線3;4号線_CN_128364781_275000_CN_47110637_275000/LConn3 -- 東京南線3;4号線_CN_128364781_275000_CN_379474501_275000/LConn3 -- bus85/LConn1
  T_210765350__花見川変電所_(Hanamigawa_Hendensho)/LConn1 -- 花見川線_CN_210765350_275000_CN_211241774_275000/LConn1
  T_210765350__花見川変電所_(Hanamigawa_Hendensho)/LConn2 -- 花見川線_CN_210765350_275000_CN_211241774_275000/LConn2
  花見川線_CN_210765350_275000_CN_211241774_275000/LConn3 -- T_210765350__花見川変電所_(Hanamigawa_Hendensho)/LConn3 -- bus86/LConn1
  T_211241774__/LConn1 -- 花見川線_CN_210765350_275000_CN_211241774_275000/RConn1
  T_211241774__/LConn2 -- 花見川線_CN_210765350_275000_CN_211241774_275000/RConn2
  花見川線_CN_210765350_275000_CN_211241774_275000/RConn3 -- T_211241774__/LConn3 -- bus87/LConn1
  _CN_179863079_275000_CN_256894928_275000/LConn1 -- T_179863079_275000_/LConn1 -- 道央北幹線_CN_179863079_275000_CN_168524732_275000/LConn1
  _CN_179863079_275000_CN_256894928_275000/LConn2 -- T_179863079_275000_/LConn2 -- 道央北幹線_CN_179863079_275000_CN_168524732_275000/LConn2
  _CN_179863079_275000_CN_256894928_275000/LConn3 -- T_179863079_275000_/LConn3 -- 道央北幹線_CN_179863079_275000_CN_168524732_275000/LConn3 -- bus88/LConn1
  T_256894928__/LConn1 -- _CN_179863079_275000_CN_256894928_275000/RConn1
  T_256894928__/LConn2 -- _CN_179863079_275000_CN_256894928_275000/RConn2
  _CN_179863079_275000_CN_256894928_275000/RConn3 -- T_256894928__/LConn3 -- bus89/LConn1
  T_168524732__/LConn1 -- 道央北幹線_CN_179863079_275000_CN_168524732_275000/RConn1
  T_168524732__/LConn2 -- 道央北幹線_CN_179863079_275000_CN_168524732_275000/RConn2
  道央北幹線_CN_179863079_275000_CN_168524732_275000/RConn3 -- T_168524732__/LConn3 -- bus90/LConn1
  T_319300956_275000_中越変電所/LConn1 -- _CN_319300956_275000_CN_318218831_275000/LConn1
  T_319300956_275000_中越変電所/LConn2 -- _CN_319300956_275000_CN_318218831_275000/LConn2
  _CN_319300956_275000_CN_318218831_275000/LConn3 -- T_319300956_275000_中越変電所/LConn3 -- bus91/LConn1
  _CN_319300956_275000_CN_318218831_275000/RConn1 -- T_318218831_275000_/LConn1 -- _CN_318218831_275000_CN_169993955_275000/LConn1 -- _CN_318218831_275000_CN_170016148_275000/LConn1 -- _CN_103818820_275000_CN_318218831_275000/LConn1
  _CN_319300956_275000_CN_318218831_275000/RConn2 -- T_318218831_275000_/LConn2 -- _CN_318218831_275000_CN_169993955_275000/LConn2 -- _CN_318218831_275000_CN_170016148_275000/LConn2 -- _CN_103818820_275000_CN_318218831_275000/LConn2
  _CN_319300956_275000_CN_318218831_275000/RConn3 -- T_318218831_275000_/LConn3 -- _CN_318218831_275000_CN_169993955_275000/LConn3 -- _CN_318218831_275000_CN_170016148_275000/LConn3 -- bus92/LConn1 -- _CN_103818820_275000_CN_318218831_275000/LConn3
  西部西濃線_(Seibu_Seinō_Sen)_CN_170537514_275000_CN_161948515_275000/RConn1 -- T_161948515_275000_西濃変電所_(Seinō_Hendensho)/LConn1 -- _CN_161946849_275000_CN_161948515_275000/LConn1
  西部西濃線_(Seibu_Seinō_Sen)_CN_170537514_275000_CN_161948515_275000/RConn2 -- T_161948515_275000_西濃変電所_(Seinō_Hendensho)/LConn2 -- _CN_161946849_275000_CN_161948515_275000/LConn2
  西部西濃線_(Seibu_Seinō_Sen)_CN_170537514_275000_CN_161948515_275000/RConn3 -- T_161948515_275000_西濃変電所_(Seinō_Hendensho)/LConn3 -- _CN_161946849_275000_CN_161948515_275000/LConn3 -- bus93/LConn1
  _CN_170537514_275000_CN_170793702_275000/RConn1 -- T_170793702_275000_西名古屋/LConn1 -- _CN_170793702_275000_CN_170793703_275000/LConn1 -- _CN_170793702_275000_CN_180359727_275000/LConn1
  _CN_170537514_275000_CN_170793702_275000/RConn2 -- T_170793702_275000_西名古屋/LConn2 -- _CN_170793702_275000_CN_170793703_275000/LConn2 -- _CN_170793702_275000_CN_180359727_275000/LConn2
  _CN_170537514_275000_CN_170793702_275000/RConn3 -- T_170793702_275000_西名古屋/LConn3 -- _CN_170793702_275000_CN_170793703_275000/LConn3 -- _CN_170793702_275000_CN_180359727_275000/LConn3 -- bus94/LConn1
  _CN_170537514_275000_CN_170793703_275000/RConn1 -- T_170793703_275000_西尾張/LConn1 -- _CN_170793702_275000_CN_170793703_275000/RConn1 -- _CN_262597734_275000_CN_170793703_275000/LConn1
  _CN_170537514_275000_CN_170793703_275000/RConn2 -- T_170793703_275000_西尾張/LConn2 -- _CN_170793702_275000_CN_170793703_275000/RConn2 -- _CN_262597734_275000_CN_170793703_275000/LConn2
  _CN_170537514_275000_CN_170793703_275000/RConn3 -- T_170793703_275000_西尾張/LConn3 -- _CN_170793702_275000_CN_170793703_275000/RConn3 -- bus95/LConn1 -- _CN_262597734_275000_CN_170793703_275000/LConn3
  _CN_340647468_275000_CN_340648895_275000/LConn1 -- T_340647468__/LConn1 -- _CN_340647468_275000_CN_168852840_275000/LConn1
  _CN_340647468_275000_CN_340648895_275000/LConn2 -- T_340647468__/LConn2 -- _CN_340647468_275000_CN_168852840_275000/LConn2
  _CN_340647468_275000_CN_340648895_275000/LConn3 -- T_340647468__/LConn3 -- _CN_340647468_275000_CN_168852840_275000/LConn3 -- bus96/LConn1
  _CN_340647468_275000_CN_340648895_275000/RConn1 -- T_340648895__/LConn1 -- _CN_105298089_275000_CN_340648895_275000/LConn1
  _CN_340647468_275000_CN_340648895_275000/RConn2 -- T_340648895__/LConn2 -- _CN_105298089_275000_CN_340648895_275000/LConn2
  _CN_340647468_275000_CN_340648895_275000/RConn3 -- T_340648895__/LConn3 -- _CN_105298089_275000_CN_340648895_275000/LConn3 -- bus97/LConn1
  _CN_340647468_275000_CN_168852840_275000/RConn1 -- T_168852840__/LConn1 -- 新京葉線_CN_151706977_275000_CN_168852840_275000/LConn1
  _CN_340647468_275000_CN_168852840_275000/RConn2 -- T_168852840__/LConn2 -- 新京葉線_CN_151706977_275000_CN_168852840_275000/LConn2
  _CN_340647468_275000_CN_168852840_275000/RConn3 -- T_168852840__/LConn3 -- 新京葉線_CN_151706977_275000_CN_168852840_275000/LConn3 -- bus98/LConn1
  T_192745005_275000_丸山変電所_(Maruyama_Hendensho)/LConn1 -- 丸山幹線_(Maruyama_Kansen)_CN_192745005_275000_CN_161946848_275000/LConn1
  T_192745005_275000_丸山変電所_(Maruyama_Hendensho)/LConn2 -- 丸山幹線_(Maruyama_Kansen)_CN_192745005_275000_CN_161946848_275000/LConn2
  丸山幹線_(Maruyama_Kansen)_CN_192745005_275000_CN_161946848_275000/LConn3 -- T_192745005_275000_丸山変電所_(Maruyama_Hendensho)/LConn3 -- bus99/LConn1
  丸山幹線_(Maruyama_Kansen)_CN_192745005_275000_CN_161946848_275000/RConn1 -- T_161946848_275000_関開閉所_(Seki)/LConn1 -- _CN_161946848_275000_CN_190734269_275000/LConn1
  丸山幹線_(Maruyama_Kansen)_CN_192745005_275000_CN_161946848_275000/RConn2 -- T_161946848_275000_関開閉所_(Seki)/LConn2 -- _CN_161946848_275000_CN_190734269_275000/LConn2
  丸山幹線_(Maruyama_Kansen)_CN_192745005_275000_CN_161946848_275000/RConn3 -- T_161946848_275000_関開閉所_(Seki)/LConn3 -- _CN_161946848_275000_CN_190734269_275000/LConn3 -- bus100/LConn1
  _CN_168903220_275000_CN_315434352_275000/LConn1 -- T_168903220_275000_/LConn1 -- _CN_168903220_275000_CN_315434358_275000/LConn1
  _CN_168903220_275000_CN_315434352_275000/LConn2 -- T_168903220_275000_/LConn2 -- _CN_168903220_275000_CN_315434358_275000/LConn2
  _CN_168903220_275000_CN_315434352_275000/LConn3 -- T_168903220_275000_/LConn3 -- _CN_168903220_275000_CN_315434358_275000/LConn3 -- bus101/LConn1
  _CN_168903220_275000_CN_315434352_275000/RConn1 -- T_315434352__/LConn1 -- 中東京幹線_CN_315434352_275000_CN_152991099_275000/LConn1
  _CN_168903220_275000_CN_315434352_275000/RConn2 -- T_315434352__/LConn2 -- 中東京幹線_CN_315434352_275000_CN_152991099_275000/LConn2
  _CN_168903220_275000_CN_315434352_275000/RConn3 -- T_315434352__/LConn3 -- 中東京幹線_CN_315434352_275000_CN_152991099_275000/LConn3 -- bus102/LConn1
  T_315434358_500000_新岡部変電所/LConn1 -- _CN_168903220_275000_CN_315434358_275000/RConn1
  T_315434358_500000_新岡部変電所/LConn2 -- _CN_168903220_275000_CN_315434358_275000/RConn2
  _CN_168903220_275000_CN_315434358_275000/RConn3 -- T_315434358_500000_新岡部変電所/LConn3 -- bus103/LConn1
  泉南東大阪線_(Sennan_Higashiōsaka_sen)_CN_108199478_275000_CN_158522649_275000/LConn1 -- T_108199478_275000_南大阪変電所_(Minamiōsaka_Hendensho)/LConn1 -- _CN_108199478_275000_CN_109834508_275000/LConn1
  泉南東大阪線_(Sennan_Higashiōsaka_sen)_CN_108199478_275000_CN_158522649_275000/LConn2 -- T_108199478_275000_南大阪変電所_(Minamiōsaka_Hendensho)/LConn2 -- _CN_108199478_275000_CN_109834508_275000/LConn2
  泉南東大阪線_(Sennan_Higashiōsaka_sen)_CN_108199478_275000_CN_158522649_275000/LConn3 -- T_108199478_275000_南大阪変電所_(Minamiōsaka_Hendensho)/LConn3 -- _CN_108199478_275000_CN_109834508_275000/LConn3 -- bus104/LConn1
  泉南東大阪線_(Sennan_Higashiōsaka_sen)_CN_108199478_275000_CN_158522649_275000/RConn1 -- T_158522649_275000_東大阪変電所/LConn1 -- _CN_161727149_275000_CN_158522649_275000/LConn1
  泉南東大阪線_(Sennan_Higashiōsaka_sen)_CN_108199478_275000_CN_158522649_275000/RConn2 -- T_158522649_275000_東大阪変電所/LConn2 -- _CN_161727149_275000_CN_158522649_275000/LConn2
  泉南東大阪線_(Sennan_Higashiōsaka_sen)_CN_108199478_275000_CN_158522649_275000/RConn3 -- T_158522649_275000_東大阪変電所/LConn3 -- _CN_161727149_275000_CN_158522649_275000/LConn3 -- bus105/LConn1
  _CN_108199478_275000_CN_109834508_275000/RConn1 -- T_109834508_275000_金剛開閉所_(Kongō_Kaiheisho)/LConn1 -- 北葛城線_(Kita_Katsuragi_Sen)_CN_160374974_275000_CN_109834508_275000/LConn1 -- 金剛線_(Kongō_sen)_CN_109834508_275000_CN_291678103_275000/LConn1
  _CN_108199478_275000_CN_109834508_275000/RConn2 -- T_109834508_275000_金剛開閉所_(Kongō_Kaiheisho)/LConn2 -- 北葛城線_(Kita_Katsuragi_Sen)_CN_160374974_275000_CN_109834508_275000/LConn2 -- 金剛線_(Kongō_sen)_CN_109834508_275000_CN_291678103_275000/LConn2
  _CN_108199478_275000_CN_109834508_275000/RConn3 -- T_109834508_275000_金剛開閉所_(Kongō_Kaiheisho)/LConn3 -- 北葛城線_(Kita_Katsuragi_Sen)_CN_160374974_275000_CN_109834508_275000/LConn3 -- 金剛線_(Kongō_sen)_CN_109834508_275000_CN_291678103_275000/LConn3 -- bus106/LConn1
  T_315614776_275000_/LConn1 -- _CN_315614776_275000_CN_315614783_275000/LConn1
  T_315614776_275000_/LConn2 -- _CN_315614776_275000_CN_315614783_275000/LConn2
  _CN_315614776_275000_CN_315614783_275000/LConn3 -- T_315614776_275000_/LConn3 -- bus107/LConn1
  _CN_315614776_275000_CN_315614783_275000/RConn1 -- T_315614783_275000_/LConn1 -- _CN_315614783_275000_CN_256682313_275000/LConn1
  _CN_315614776_275000_CN_315614783_275000/RConn2 -- T_315614783_275000_/LConn2 -- _CN_315614783_275000_CN_256682313_275000/LConn2
  _CN_315614776_275000_CN_315614783_275000/RConn3 -- T_315614783_275000_/LConn3 -- _CN_315614783_275000_CN_256682313_275000/LConn3 -- bus108/LConn1
  T_316566585_275000_/LConn1 -- _CN_316566585_275000_CN_174636874_275000/LConn1
  T_316566585_275000_/LConn2 -- _CN_316566585_275000_CN_174636874_275000/LConn2
  _CN_316566585_275000_CN_174636874_275000/LConn3 -- T_316566585_275000_/LConn3 -- bus109/LConn1
  _CN_316566585_275000_CN_174636874_275000/RConn1 -- T_174636874_275000_岩手変電所/RConn1 -- _CN_316566588_275000_CN_174636874_275000/LConn1 -- L_174636874/LConn1
  _CN_316566585_275000_CN_174636874_275000/RConn2 -- T_174636874_275000_岩手変電所/RConn2 -- _CN_316566588_275000_CN_174636874_275000/LConn2 -- L_174636874/LConn2
  _CN_316566585_275000_CN_174636874_275000/RConn3 -- T_174636874_275000_岩手変電所/RConn3 -- _CN_316566588_275000_CN_174636874_275000/LConn3 -- L_174636874/LConn3 -- bus110/LConn1
  _CN_316566588_275000_CN_174636874_275000/RConn1 -- T_316566588_275000_/LConn1 -- _CN_316566588_275000_CN_106076988_275000/LConn1 -- _CN_316566588_275000_CN_316581632_275000/LConn1
  _CN_316566588_275000_CN_174636874_275000/RConn2 -- T_316566588_275000_/LConn2 -- _CN_316566588_275000_CN_106076988_275000/LConn2 -- _CN_316566588_275000_CN_316581632_275000/LConn2
  _CN_316566588_275000_CN_174636874_275000/RConn3 -- T_316566588_275000_/LConn3 -- _CN_316566588_275000_CN_106076988_275000/LConn3 -- _CN_316566588_275000_CN_316581632_275000/LConn3 -- bus111/LConn1
  _CN_316566588_275000_CN_106076988_275000/RConn1 -- T_106076988_500000_宮城変電所/RConn1 -- _CN_106076988_275000_CN_308348224_275000/LConn1 -- L_106076988/LConn1 -- _CN_316796028_275000_CN_106076988_275000/LConn1 -- _CN_106076988_275000_CN_316727625_275000/LConn1 -- _CN_103818820_275000_CN_106076988_275000/LConn1
  _CN_316566588_275000_CN_106076988_275000/RConn2 -- T_106076988_500000_宮城変電所/RConn2 -- _CN_106076988_275000_CN_308348224_275000/LConn2 -- L_106076988/LConn2 -- _CN_316796028_275000_CN_106076988_275000/LConn2 -- _CN_106076988_275000_CN_316727625_275000/LConn2 -- _CN_103818820_275000_CN_106076988_275000/LConn2
  _CN_316566588_275000_CN_106076988_275000/RConn3 -- T_106076988_500000_宮城変電所/RConn3 -- _CN_106076988_275000_CN_308348224_275000/LConn3 -- L_106076988/LConn3 -- bus112/LConn1 -- _CN_316796028_275000_CN_106076988_275000/LConn3 -- _CN_106076988_275000_CN_316727625_275000/LConn3 -- _CN_103818820_275000_CN_106076988_275000/LConn3
  T_316581632_275000_/LConn1 -- _CN_316566588_275000_CN_316581632_275000/RConn1
  T_316581632_275000_/LConn2 -- _CN_316566588_275000_CN_316581632_275000/RConn2
  _CN_316566588_275000_CN_316581632_275000/RConn3 -- T_316581632_275000_/LConn3 -- bus113/LConn1
  _CN_315614783_275000_CN_256682313_275000/RConn1 -- T_256682313__/LConn1 -- _CN_315757225_275000_CN_256682313_275000/LConn1
  _CN_315614783_275000_CN_256682313_275000/RConn2 -- T_256682313__/LConn2 -- _CN_315757225_275000_CN_256682313_275000/LConn2
  _CN_315614783_275000_CN_256682313_275000/RConn3 -- T_256682313__/LConn3 -- _CN_315757225_275000_CN_256682313_275000/LConn3 -- bus114/LConn1
  _CN_103818820_275000_CN_318218831_275000/RConn1 -- T_103818820_275000_仙台変電所/LConn1 -- _CN_103818820_275000_CN_250430935_275000/LConn1 -- _CN_103818820_275000_CN_106076988_275000/RConn1
  _CN_103818820_275000_CN_318218831_275000/RConn2 -- T_103818820_275000_仙台変電所/LConn2 -- _CN_103818820_275000_CN_250430935_275000/LConn2 -- _CN_103818820_275000_CN_106076988_275000/RConn2
  _CN_103818820_275000_CN_318218831_275000/RConn3 -- T_103818820_275000_仙台変電所/LConn3 -- _CN_103818820_275000_CN_250430935_275000/LConn3 -- _CN_103818820_275000_CN_106076988_275000/RConn3 -- bus115/LConn1
  _CN_103818820_275000_CN_250430935_275000/RConn1 -- T_250430935_275000_米沢変電所_(Yonezawa_Hendensho)/LConn1 -- _CN_250430935_275000_CN_107262429_275000/LConn1 -- _CN_169993955_275000_CN_250430935_275000/LConn1 -- _CN_250430935_275000_CN_354115662_275000/LConn1
  _CN_103818820_275000_CN_250430935_275000/RConn2 -- T_250430935_275000_米沢変電所_(Yonezawa_Hendensho)/LConn2 -- _CN_250430935_275000_CN_107262429_275000/LConn2 -- _CN_169993955_275000_CN_250430935_275000/LConn2 -- _CN_250430935_275000_CN_354115662_275000/LConn2
  _CN_103818820_275000_CN_250430935_275000/RConn3 -- T_250430935_275000_米沢変電所_(Yonezawa_Hendensho)/LConn3 -- _CN_250430935_275000_CN_107262429_275000/LConn3 -- bus116/LConn1 -- _CN_169993955_275000_CN_250430935_275000/LConn3 -- _CN_250430935_275000_CN_354115662_275000/LConn3
  T_170693194_275000_淀川/LConn1 -- _CN_170693194_275000_CN_169031921_275000/LConn1
  T_170693194_275000_淀川/LConn2 -- _CN_170693194_275000_CN_169031921_275000/LConn2
  _CN_170693194_275000_CN_169031921_275000/LConn3 -- T_170693194_275000_淀川/LConn3 -- bus117/LConn1
  _CN_170693194_275000_CN_169031921_275000/RConn1 -- T_169031921_500000_西京都変電所_(Nishi_Kyōto_Hendensho)/RConn1 -- L_169031921/LConn1
  _CN_170693194_275000_CN_169031921_275000/RConn2 -- T_169031921_500000_西京都変電所_(Nishi_Kyōto_Hendensho)/RConn2 -- L_169031921/LConn2
  _CN_170693194_275000_CN_169031921_275000/RConn3 -- T_169031921_500000_西京都変電所_(Nishi_Kyōto_Hendensho)/RConn3 -- L_169031921/LConn3 -- bus118/LConn1
  _CN_318218831_275000_CN_169993955_275000/RConn1 -- T_169993955_275000_新潟変電所/LConn1 -- _CN_169993955_275000_CN_250430935_275000/RConn1
  _CN_318218831_275000_CN_169993955_275000/RConn2 -- T_169993955_275000_新潟変電所/LConn2 -- _CN_169993955_275000_CN_250430935_275000/RConn2
  _CN_318218831_275000_CN_169993955_275000/RConn3 -- T_169993955_275000_新潟変電所/LConn3 -- _CN_169993955_275000_CN_250430935_275000/RConn3 -- bus119/LConn1
  T_170016148_275000_北新潟変電所/LConn1 -- _CN_318218831_275000_CN_170016148_275000/RConn1
  T_170016148_275000_北新潟変電所/LConn2 -- _CN_318218831_275000_CN_170016148_275000/RConn2
  _CN_318218831_275000_CN_170016148_275000/RConn3 -- T_170016148_275000_北新潟変電所/LConn3 -- bus120/LConn1
  _CN_169122898_275000_CN_170247359_275000/RConn1 -- T_170247359_275000_/LConn1 -- _CN_170247308_275000_CN_170247359_275000/LConn1 -- _CN_170247314_275000_CN_170247359_275000/LConn1
  _CN_169122898_275000_CN_170247359_275000/RConn2 -- T_170247359_275000_/LConn2 -- _CN_170247308_275000_CN_170247359_275000/LConn2 -- _CN_170247314_275000_CN_170247359_275000/LConn2
  _CN_169122898_275000_CN_170247359_275000/RConn3 -- T_170247359_275000_/LConn3 -- _CN_170247308_275000_CN_170247359_275000/LConn3 -- _CN_170247314_275000_CN_170247359_275000/LConn3 -- bus121/LConn1
  _CN_169122898_275000_CN_179417733_275000/RConn1 -- T_179417733_275000_/LConn1 -- _CN_179417733_275000_CN_180359744_275000/LConn1
  _CN_169122898_275000_CN_179417733_275000/RConn2 -- T_179417733_275000_/LConn2 -- _CN_179417733_275000_CN_180359744_275000/LConn2
  _CN_169122898_275000_CN_179417733_275000/RConn3 -- T_179417733_275000_/LConn3 -- _CN_179417733_275000_CN_180359744_275000/LConn3 -- bus122/LConn1
  _CN_170366038_275000_CN_161946849_275000/LConn1 -- T_170366038_275000_/LConn1 -- _CN_170366038_275000_CN_169121278_275000/RConn1
  _CN_170366038_275000_CN_161946849_275000/LConn2 -- T_170366038_275000_/LConn2 -- _CN_170366038_275000_CN_169121278_275000/RConn2
  _CN_170366038_275000_CN_161946849_275000/LConn3 -- T_170366038_275000_/LConn3 -- _CN_170366038_275000_CN_169121278_275000/RConn3 -- bus123/LConn1
  _CN_170366038_275000_CN_161946849_275000/RConn1 -- T_161946849_500000;275000_北部変電所/RConn1 -- _CN_161946849_275000_CN_210658603_275000/LConn1 -- _CN_161946849_275000_CN_161948515_275000/RConn1 -- L_161946849/LConn1
  _CN_170366038_275000_CN_161946849_275000/RConn2 -- T_161946849_500000;275000_北部変電所/RConn2 -- _CN_161946849_275000_CN_210658603_275000/LConn2 -- _CN_161946849_275000_CN_161948515_275000/RConn2 -- L_161946849/LConn2
  _CN_170366038_275000_CN_161946849_275000/RConn3 -- T_161946849_500000;275000_北部変電所/RConn3 -- _CN_161946849_275000_CN_210658603_275000/LConn3 -- _CN_161946849_275000_CN_161948515_275000/RConn3 -- L_161946849/LConn3 -- bus124/LConn1
  T_170366039__中部電力遠江変電所/LConn1 -- 三河遠江線_CN_170366039_275000_CN_210090094_275000/RConn1
  T_170366039__中部電力遠江変電所/LConn2 -- 三河遠江線_CN_170366039_275000_CN_210090094_275000/RConn2
  三河遠江線_CN_170366039_275000_CN_210090094_275000/RConn3 -- T_170366039__中部電力遠江変電所/LConn3 -- bus125/LConn1
  T_104375141_275000_須賀川変電所_(Sukagawa_Hendensho)/LConn1 -- _CN_104375141_275000_CN_107262429_275000/LConn1
  T_104375141_275000_須賀川変電所_(Sukagawa_Hendensho)/LConn2 -- _CN_104375141_275000_CN_107262429_275000/LConn2
  _CN_104375141_275000_CN_107262429_275000/LConn3 -- T_104375141_275000_須賀川変電所_(Sukagawa_Hendensho)/LConn3 -- bus126/LConn1
  _CN_104375141_275000_CN_107262429_275000/RConn1 -- T_107262429_275000_福島変電所/LConn1 -- _CN_316459359_275000_CN_107262429_275000/LConn1 -- _CN_250430935_275000_CN_107262429_275000/RConn1 -- _CN_156208858_275000_CN_107262429_275000/LConn1
  _CN_104375141_275000_CN_107262429_275000/RConn2 -- T_107262429_275000_福島変電所/LConn2 -- _CN_316459359_275000_CN_107262429_275000/LConn2 -- _CN_250430935_275000_CN_107262429_275000/RConn2 -- _CN_156208858_275000_CN_107262429_275000/LConn2
  _CN_104375141_275000_CN_107262429_275000/RConn3 -- T_107262429_275000_福島変電所/LConn3 -- _CN_316459359_275000_CN_107262429_275000/LConn3 -- bus127/LConn1 -- _CN_250430935_275000_CN_107262429_275000/RConn3 -- _CN_156208858_275000_CN_107262429_275000/LConn3
  T_262597734__海部開閉所/LConn1 -- _CN_262597734_275000_CN_170793703_275000/RConn1
  T_262597734__海部開閉所/LConn2 -- _CN_262597734_275000_CN_170793703_275000/RConn2
  _CN_262597734_275000_CN_170793703_275000/RConn3 -- T_262597734__海部開閉所/LConn3 -- bus128/LConn1
  T_315757225_275000_/LConn1 -- _CN_315757225_275000_CN_256682313_275000/RConn1
  T_315757225_275000_/LConn2 -- _CN_315757225_275000_CN_256682313_275000/RConn2
  _CN_315757225_275000_CN_256682313_275000/RConn3 -- T_315757225_275000_/LConn3 -- bus129/LConn1
  _CN_87682157_275000_CN_133641619_275000/LConn1 -- T_87682157_275000_南川越変電所_(Minamikawagoe_Hendensho)/LConn1 -- _CN_87682157_275000_CN_159491797_275000/LConn1 -- _CN_87682157_275000_CN_128581912_275000/LConn1
  _CN_87682157_275000_CN_133641619_275000/LConn2 -- T_87682157_275000_南川越変電所_(Minamikawagoe_Hendensho)/LConn2 -- _CN_87682157_275000_CN_159491797_275000/LConn2 -- _CN_87682157_275000_CN_128581912_275000/LConn2
  _CN_87682157_275000_CN_133641619_275000/LConn3 -- T_87682157_275000_南川越変電所_(Minamikawagoe_Hendensho)/LConn3 -- _CN_87682157_275000_CN_159491797_275000/LConn3 -- _CN_87682157_275000_CN_128581912_275000/LConn3 -- bus130/LConn1
  _CN_87682157_275000_CN_133641619_275000/RConn1 -- T_133641619_500000_新所沢変電所_(Shin_Tokorozawa_Hendensho)/RConn1 -- 南狭山線_CN_159491797_275000_CN_133641619_275000/LConn1 -- 中沢線3;4号線_CN_152991099_275000_CN_133641619_275000/LConn1 -- L_133641619/LConn1
  _CN_87682157_275000_CN_133641619_275000/RConn2 -- T_133641619_500000_新所沢変電所_(Shin_Tokorozawa_Hendensho)/RConn2 -- 南狭山線_CN_159491797_275000_CN_133641619_275000/LConn2 -- 中沢線3;4号線_CN_152991099_275000_CN_133641619_275000/LConn2 -- L_133641619/LConn2
  _CN_87682157_275000_CN_133641619_275000/RConn3 -- T_133641619_500000_新所沢変電所_(Shin_Tokorozawa_Hendensho)/RConn3 -- 南狭山線_CN_159491797_275000_CN_133641619_275000/LConn3 -- 中沢線3;4号線_CN_152991099_275000_CN_133641619_275000/LConn3 -- L_133641619/LConn3 -- bus131/LConn1
  _CN_87682157_275000_CN_159491797_275000/RConn1 -- T_159491797_275000_南狭山変電所_(Minamisayama_Hendensho)/LConn1 -- _CN_159491797_275000_CN_136298957_275000/LConn1 -- 南狭山線_CN_159491797_275000_CN_133641619_275000/RConn1
  _CN_87682157_275000_CN_159491797_275000/RConn2 -- T_159491797_275000_南狭山変電所_(Minamisayama_Hendensho)/LConn2 -- _CN_159491797_275000_CN_136298957_275000/LConn2 -- 南狭山線_CN_159491797_275000_CN_133641619_275000/RConn2
  _CN_87682157_275000_CN_159491797_275000/RConn3 -- T_159491797_275000_南狭山変電所_(Minamisayama_Hendensho)/LConn3 -- _CN_159491797_275000_CN_136298957_275000/LConn3 -- 南狭山線_CN_159491797_275000_CN_133641619_275000/RConn3 -- bus132/LConn1
  _CN_87682157_275000_CN_128581912_275000/RConn1 -- T_128581912_500000;275000;66000_新坂戸変電所/RConn1 -- 東京中線_CN_133137636_275000_CN_128581912_275000/LConn1 -- L_128581912/LConn1
  _CN_87682157_275000_CN_128581912_275000/RConn2 -- T_128581912_500000;275000;66000_新坂戸変電所/RConn2 -- 東京中線_CN_133137636_275000_CN_128581912_275000/LConn2 -- L_128581912/LConn2
  _CN_87682157_275000_CN_128581912_275000/RConn3 -- T_128581912_500000;275000;66000_新坂戸変電所/RConn3 -- 東京中線_CN_133137636_275000_CN_128581912_275000/LConn3 -- L_128581912/LConn3 -- bus133/LConn1
  _CN_105291887_275000_CN_103827577_275000/LConn1 -- T_105291887_275000_那珂変電所_(Naka_Hendensho)/LConn1 -- 那珂線_(Naka_Sen)_CN_105291887_275000_CN_168839127_275000/LConn1
  _CN_105291887_275000_CN_103827577_275000/LConn2 -- T_105291887_275000_那珂変電所_(Naka_Hendensho)/LConn2 -- 那珂線_(Naka_Sen)_CN_105291887_275000_CN_168839127_275000/LConn2
  _CN_105291887_275000_CN_103827577_275000/LConn3 -- T_105291887_275000_那珂変電所_(Naka_Hendensho)/LConn3 -- 那珂線_(Naka_Sen)_CN_105291887_275000_CN_168839127_275000/LConn3 -- bus134/LConn1
  G_103827577_常陸那珂火力発電所/RConn1 -- _CN_105291887_275000_CN_103827577_275000/RConn1
  G_103827577_常陸那珂火力発電所/RConn2 -- _CN_105291887_275000_CN_103827577_275000/RConn2
  _CN_105291887_275000_CN_103827577_275000/RConn3 -- G_103827577_常陸那珂火力発電所/RConn3 -- bus135/LConn1
  那珂線_(Naka_Sen)_CN_105291887_275000_CN_168839127_275000/RConn1 -- T_168839127__新茂木/RConn1 -- L_168839127/LConn1
  那珂線_(Naka_Sen)_CN_105291887_275000_CN_168839127_275000/RConn2 -- T_168839127__新茂木/RConn2 -- L_168839127/LConn2
  那珂線_(Naka_Sen)_CN_105291887_275000_CN_168839127_275000/RConn3 -- T_168839127__新茂木/RConn3 -- L_168839127/LConn3 -- bus136/LConn1
  西越谷線_(Nishi_Koshigaya_Sen)_CN_155411568_275000_CN_153521822_275000/LConn1 -- T_155411568__/LConn1 -- 西越谷線_(Nishi_Koshigaya_Sen)_CN_155411568_275000_CN_133137636_275000/LConn1
  西越谷線_(Nishi_Koshigaya_Sen)_CN_155411568_275000_CN_153521822_275000/LConn2 -- T_155411568__/LConn2 -- 西越谷線_(Nishi_Koshigaya_Sen)_CN_155411568_275000_CN_133137636_275000/LConn2
  西越谷線_(Nishi_Koshigaya_Sen)_CN_155411568_275000_CN_153521822_275000/LConn3 -- T_155411568__/LConn3 -- 西越谷線_(Nishi_Koshigaya_Sen)_CN_155411568_275000_CN_133137636_275000/LConn3 -- bus137/LConn1
  T_153521822_275000_西越谷変電所_(Nishi_Koshigaya_Hendensho)/LConn1 -- 西越谷線_(Nishi_Koshigaya_Sen)_CN_155411568_275000_CN_153521822_275000/RConn1
  T_153521822_275000_西越谷変電所_(Nishi_Koshigaya_Hendensho)/LConn2 -- 西越谷線_(Nishi_Koshigaya_Sen)_CN_155411568_275000_CN_153521822_275000/RConn2
  西越谷線_(Nishi_Koshigaya_Sen)_CN_155411568_275000_CN_153521822_275000/RConn3 -- T_153521822_275000_西越谷変電所_(Nishi_Koshigaya_Hendensho)/LConn3 -- bus138/LConn1
  西越谷線_(Nishi_Koshigaya_Sen)_CN_155411568_275000_CN_133137636_275000/RConn1 -- T_133137636_275000_北東京変電所_(Kita_Tōkyō_Hendensho)/LConn1 -- 東京中線_CN_133137636_275000_CN_128581912_275000/RConn1 -- 河北1・2線_(Kahoku_1・2_Sen)_CN_133137636_275000_CN_133135172_275000/LConn1 -- 東京北線_(Tōkyō_Kita_Sen)_CN_133137636_275000_CN_151706977_275000/LConn1
  西越谷線_(Nishi_Koshigaya_Sen)_CN_155411568_275000_CN_133137636_275000/RConn2 -- T_133137636_275000_北東京変電所_(Kita_Tōkyō_Hendensho)/LConn2 -- 東京中線_CN_133137636_275000_CN_128581912_275000/RConn2 -- 河北1・2線_(Kahoku_1・2_Sen)_CN_133137636_275000_CN_133135172_275000/LConn2 -- 東京北線_(Tōkyō_Kita_Sen)_CN_133137636_275000_CN_151706977_275000/LConn2
  西越谷線_(Nishi_Koshigaya_Sen)_CN_155411568_275000_CN_133137636_275000/RConn3 -- T_133137636_275000_北東京変電所_(Kita_Tōkyō_Hendensho)/LConn3 -- 東京中線_CN_133137636_275000_CN_128581912_275000/RConn3 -- bus139/LConn1 -- 河北1・2線_(Kahoku_1・2_Sen)_CN_133137636_275000_CN_133135172_275000/LConn3 -- 東京北線_(Tōkyō_Kita_Sen)_CN_133137636_275000_CN_151706977_275000/LConn3
  T_316796028_275000_/LConn1 -- _CN_316796028_275000_CN_106076988_275000/RConn1
  T_316796028_275000_/LConn2 -- _CN_316796028_275000_CN_106076988_275000/RConn2
  _CN_316796028_275000_CN_106076988_275000/RConn3 -- T_316796028_275000_/LConn3 -- bus140/LConn1
  G_180359744_知多火力発電所/RConn1 -- _CN_179417733_275000_CN_180359744_275000/RConn1
  G_180359744_知多火力発電所/RConn2 -- _CN_179417733_275000_CN_180359744_275000/RConn2
  _CN_179417733_275000_CN_180359744_275000/RConn3 -- G_180359744_知多火力発電所/RConn3 -- bus141/LConn1
  _CN_170247308_275000_CN_170247312_275000/LConn1 -- T_170247308_275000_三河変電所/LConn1 -- _CN_170247308_275000_CN_170247359_275000/RConn1 -- 湖西三河線_CN_170247308_275000_CN_170260165_275000/LConn1
  _CN_170247308_275000_CN_170247312_275000/LConn2 -- T_170247308_275000_三河変電所/LConn2 -- _CN_170247308_275000_CN_170247359_275000/RConn2 -- 湖西三河線_CN_170247308_275000_CN_170260165_275000/LConn2
  _CN_170247308_275000_CN_170247312_275000/LConn3 -- T_170247308_275000_三河変電所/LConn3 -- _CN_170247308_275000_CN_170247359_275000/RConn3 -- 湖西三河線_CN_170247308_275000_CN_170260165_275000/LConn3 -- bus142/LConn1
  _CN_170247308_275000_CN_170247312_275000/RConn1 -- T_170247312_500000_新三河変電所/RConn1 -- 幸田新三河線_CN_170247312_275000_CN_170247314_275000/LConn1 -- L_170247312/LConn1
  _CN_170247308_275000_CN_170247312_275000/RConn2 -- T_170247312_500000_新三河変電所/RConn2 -- 幸田新三河線_CN_170247312_275000_CN_170247314_275000/LConn2 -- L_170247312/LConn2
  _CN_170247308_275000_CN_170247312_275000/RConn3 -- T_170247312_500000_新三河変電所/RConn3 -- 幸田新三河線_CN_170247312_275000_CN_170247314_275000/LConn3 -- L_170247312/LConn3 -- bus143/LConn1
  湖西三河線_CN_170247308_275000_CN_170260165_275000/RConn1 -- T_170260165_275000_中部電力湖西変電所/LConn1 -- 田原湖西線_CN_170260165_275000_CN_170260169_275000/LConn1
  湖西三河線_CN_170247308_275000_CN_170260165_275000/RConn2 -- T_170260165_275000_中部電力湖西変電所/LConn2 -- 田原湖西線_CN_170260165_275000_CN_170260169_275000/LConn2
  湖西三河線_CN_170247308_275000_CN_170260165_275000/RConn3 -- T_170260165_275000_中部電力湖西変電所/LConn3 -- 田原湖西線_CN_170260165_275000_CN_170260169_275000/LConn3 -- bus144/LConn1
  幸田新三河線_CN_170247312_275000_CN_170247314_275000/RConn1 -- T_170247314_275000_額田開閉所/LConn1 -- _CN_170247314_275000_CN_170247359_275000/RConn1
  幸田新三河線_CN_170247312_275000_CN_170247314_275000/RConn2 -- T_170247314_275000_額田開閉所/LConn2 -- _CN_170247314_275000_CN_170247359_275000/RConn2
  幸田新三河線_CN_170247312_275000_CN_170247314_275000/RConn3 -- T_170247314_275000_額田開閉所/LConn3 -- _CN_170247314_275000_CN_170247359_275000/RConn3 -- bus145/LConn1
  _CN_315461272_275000_CN_151379730_275000/LConn1 -- T_315461272_500000_新木更津変電所/RConn1 -- L_315461272/LConn1
  _CN_315461272_275000_CN_151379730_275000/LConn2 -- T_315461272_500000_新木更津変電所/RConn2 -- L_315461272/LConn2
  _CN_315461272_275000_CN_151379730_275000/LConn3 -- T_315461272_500000_新木更津変電所/RConn3 -- L_315461272/LConn3 -- bus146/LConn1
  _CN_315461272_275000_CN_151379730_275000/RConn1 -- T_151379730_500000_房総変電所_(Bōsō_Hendensho)/RConn1 -- L_151379730/LConn1
  _CN_315461272_275000_CN_151379730_275000/RConn2 -- T_151379730_500000_房総変電所_(Bōsō_Hendensho)/RConn2 -- L_151379730/LConn2
  _CN_315461272_275000_CN_151379730_275000/RConn3 -- T_151379730_500000_房総変電所_(Bōsō_Hendensho)/RConn3 -- L_151379730/LConn3 -- bus147/LConn1
  _CN_302164677_275000_CN_302164679_275000/LConn1 -- T_302164677__秋田変電所/LConn1 -- _CN_302164677_275000_CN_316727625_275000/LConn1
  _CN_302164677_275000_CN_302164679_275000/LConn2 -- T_302164677__秋田変電所/LConn2 -- _CN_302164677_275000_CN_316727625_275000/LConn2
  _CN_302164677_275000_CN_302164679_275000/LConn3 -- T_302164677__秋田変電所/LConn3 -- _CN_302164677_275000_CN_316727625_275000/LConn3 -- bus148/LConn1
  _CN_302164677_275000_CN_302164679_275000/RConn1 -- T_302164679_275000_能代変電所/LConn1 -- _CN_302164679_275000_CN_316581637_275000/LConn1
  _CN_302164677_275000_CN_302164679_275000/RConn2 -- T_302164679_275000_能代変電所/LConn2 -- _CN_302164679_275000_CN_316581637_275000/LConn2
  _CN_302164677_275000_CN_302164679_275000/RConn3 -- T_302164679_275000_能代変電所/LConn3 -- _CN_302164679_275000_CN_316581637_275000/LConn3 -- bus149/LConn1
  _CN_302164677_275000_CN_316727625_275000/RConn1 -- T_316727625_275000_/LConn1 -- _CN_106076988_275000_CN_316727625_275000/RConn1
  _CN_302164677_275000_CN_316727625_275000/RConn2 -- T_316727625_275000_/LConn2 -- _CN_106076988_275000_CN_316727625_275000/RConn2
  _CN_302164677_275000_CN_316727625_275000/RConn3 -- T_316727625_275000_/LConn3 -- _CN_106076988_275000_CN_316727625_275000/RConn3 -- bus150/LConn1
  _CN_105298089_275000_CN_340648895_275000/RConn1 -- T_105298089_500000_新佐原変電所/RConn1 -- L_105298089/LConn1
  _CN_105298089_275000_CN_340648895_275000/RConn2 -- T_105298089_500000_新佐原変電所/RConn2 -- L_105298089/LConn2
  _CN_105298089_275000_CN_340648895_275000/RConn3 -- T_105298089_500000_新佐原変電所/RConn3 -- L_105298089/LConn3 -- bus151/LConn1
  T_316581637_275000_青森変電所/LConn1 -- _CN_302164679_275000_CN_316581637_275000/RConn1
  T_316581637_275000_青森変電所/LConn2 -- _CN_302164679_275000_CN_316581637_275000/RConn2
  _CN_302164679_275000_CN_316581637_275000/RConn3 -- T_316581637_275000_青森変電所/LConn3 -- bus152/LConn1
  _CN_161727149_275000_CN_158522649_275000/RConn1 -- T_161727149_500000_新生駒変電所_(Shin_Ikoma_Hendensho)/RConn1 -- _CN_161727149_275000_CN_110682951_275000/LConn1 -- L_161727149/LConn1
  _CN_161727149_275000_CN_158522649_275000/RConn2 -- T_161727149_500000_新生駒変電所_(Shin_Ikoma_Hendensho)/RConn2 -- _CN_161727149_275000_CN_110682951_275000/LConn2 -- L_161727149/LConn2
  _CN_161727149_275000_CN_158522649_275000/RConn3 -- T_161727149_500000_新生駒変電所_(Shin_Ikoma_Hendensho)/RConn3 -- _CN_161727149_275000_CN_110682951_275000/LConn3 -- L_161727149/LConn3 -- bus153/LConn1
  _CN_161727149_275000_CN_110682951_275000/RConn1 -- T_110682951_275000_宝塚開閉所_(Takarazuka_Kaiheisho)/LConn1 -- _CN_325868333_275000_CN_110682951_275000/LConn1 -- _CN_110682951_275000_CN_110682956_275000/LConn1 -- _CN_110682951_275000_CN_110682955_275000/LConn1
  _CN_161727149_275000_CN_110682951_275000/RConn2 -- T_110682951_275000_宝塚開閉所_(Takarazuka_Kaiheisho)/LConn2 -- _CN_325868333_275000_CN_110682951_275000/LConn2 -- _CN_110682951_275000_CN_110682956_275000/LConn2 -- _CN_110682951_275000_CN_110682955_275000/LConn2
  _CN_161727149_275000_CN_110682951_275000/RConn3 -- T_110682951_275000_宝塚開閉所_(Takarazuka_Kaiheisho)/LConn3 -- _CN_325868333_275000_CN_110682951_275000/LConn3 -- _CN_110682951_275000_CN_110682956_275000/LConn3 -- _CN_110682951_275000_CN_110682955_275000/LConn3 -- bus154/LConn1
  _CN_242253497_275000_CN_185032690_275000/LConn1 -- T_242253497_275000_姫路変電所_(Himeji_Hendensho)/LConn1 -- _CN_242253497_275000_CN_241822631_275000/LConn1
  _CN_242253497_275000_CN_185032690_275000/LConn2 -- T_242253497_275000_姫路変電所_(Himeji_Hendensho)/LConn2 -- _CN_242253497_275000_CN_241822631_275000/LConn2
  _CN_242253497_275000_CN_185032690_275000/LConn3 -- T_242253497_275000_姫路変電所_(Himeji_Hendensho)/LConn3 -- _CN_242253497_275000_CN_241822631_275000/LConn3 -- bus155/LConn1
  _CN_242253497_275000_CN_185032690_275000/RConn1 -- T_185032690_275000_西神戸変電所/LConn1 -- _CN_185032690_275000_CN_110340505_275000/LConn1
  _CN_242253497_275000_CN_185032690_275000/RConn2 -- T_185032690_275000_西神戸変電所/LConn2 -- _CN_185032690_275000_CN_110340505_275000/LConn2
  _CN_242253497_275000_CN_185032690_275000/RConn3 -- T_185032690_275000_西神戸変電所/LConn3 -- _CN_185032690_275000_CN_110340505_275000/LConn3 -- bus156/LConn1
  _CN_242253497_275000_CN_241822631_275000/RConn1 -- T_241822631__/RConn1 -- _CN_241822631_275000_CN_242706111_275000/LConn1 -- L_241822631/LConn1
  _CN_242253497_275000_CN_241822631_275000/RConn2 -- T_241822631__/RConn2 -- _CN_241822631_275000_CN_242706111_275000/LConn2 -- L_241822631/LConn2
  _CN_242253497_275000_CN_241822631_275000/RConn3 -- T_241822631__/RConn3 -- _CN_241822631_275000_CN_242706111_275000/LConn3 -- L_241822631/LConn3 -- bus157/LConn1
  T_160374974_275000;77000_北葛城変電所_(Kita_Katsuragi_Hendensho)/LConn1 -- 北葛城線_(Kita_Katsuragi_Sen)_CN_160374974_275000_CN_109834508_275000/RConn1
  T_160374974_275000;77000_北葛城変電所_(Kita_Katsuragi_Hendensho)/LConn2 -- 北葛城線_(Kita_Katsuragi_Sen)_CN_160374974_275000_CN_109834508_275000/RConn2
  北葛城線_(Kita_Katsuragi_Sen)_CN_160374974_275000_CN_109834508_275000/RConn3 -- T_160374974_275000;77000_北葛城変電所_(Kita_Katsuragi_Hendensho)/LConn3 -- bus158/LConn1
  T_170260161_275000_/LConn1 -- _CN_170260161_275000_CN_170260169_275000/LConn1
  T_170260161_275000_/LConn2 -- _CN_170260161_275000_CN_170260169_275000/LConn2
  _CN_170260161_275000_CN_170260169_275000/LConn3 -- T_170260161_275000_/LConn3 -- bus159/LConn1
  _CN_170260161_275000_CN_170260169_275000/RConn1 -- T_170260169_275000_田原/LConn1 -- 田原湖西線_CN_170260165_275000_CN_170260169_275000/RConn1
  _CN_170260161_275000_CN_170260169_275000/RConn2 -- T_170260169_275000_田原/LConn2 -- 田原湖西線_CN_170260165_275000_CN_170260169_275000/RConn2
  _CN_170260161_275000_CN_170260169_275000/RConn3 -- T_170260169_275000_田原/LConn3 -- 田原湖西線_CN_170260165_275000_CN_170260169_275000/RConn3 -- bus160/LConn1
  T_133644487__/LConn1 -- 青梅線_(Ōme_Sen)_CN_133644487_275000_CN_145084773_275000/LConn1
  T_133644487__/LConn2 -- 青梅線_(Ōme_Sen)_CN_133644487_275000_CN_145084773_275000/LConn2
  青梅線_(Ōme_Sen)_CN_133644487_275000_CN_145084773_275000/LConn3 -- T_133644487__/LConn3 -- bus161/LConn1
  T_145084773_275000_青梅変電所/LConn1 -- 青梅線_(Ōme_Sen)_CN_133644487_275000_CN_145084773_275000/RConn1
  T_145084773_275000_青梅変電所/LConn2 -- 青梅線_(Ōme_Sen)_CN_133644487_275000_CN_145084773_275000/RConn2
  青梅線_(Ōme_Sen)_CN_133644487_275000_CN_145084773_275000/RConn3 -- T_145084773_275000_青梅変電所/LConn3 -- bus162/LConn1
  T_159191758_275000_北松本変電所/LConn1 -- _CN_159191758_275000_CN_211258348_275000/LConn1
  T_159191758_275000_北松本変電所/LConn2 -- _CN_159191758_275000_CN_211258348_275000/LConn2
  _CN_159191758_275000_CN_211258348_275000/LConn3 -- T_159191758_275000_北松本変電所/LConn3 -- bus163/LConn1
  _CN_159191758_275000_CN_211258348_275000/RConn1 -- T_211258348_275000_東信変電所/LConn1 -- _CN_199544541_275000_CN_211258348_275000/LConn1
  _CN_159191758_275000_CN_211258348_275000/RConn2 -- T_211258348_275000_東信変電所/LConn2 -- _CN_199544541_275000_CN_211258348_275000/LConn2
  _CN_159191758_275000_CN_211258348_275000/RConn3 -- T_211258348_275000_東信変電所/LConn3 -- _CN_199544541_275000_CN_211258348_275000/LConn3 -- bus164/LConn1
  T_136298957__新座変電所/LConn1 -- _CN_159491797_275000_CN_136298957_275000/RConn1
  T_136298957__新座変電所/LConn2 -- _CN_159491797_275000_CN_136298957_275000/RConn2
  _CN_159491797_275000_CN_136298957_275000/RConn3 -- T_136298957__新座変電所/LConn3 -- bus165/LConn1
  _CN_156208858_275000_CN_107262429_275000/RConn1 -- T_156208858_500000_南相馬変電所/RConn1 -- L_156208858/LConn1
  _CN_156208858_275000_CN_107262429_275000/RConn2 -- T_156208858_500000_南相馬変電所/RConn2 -- L_156208858/LConn2
  _CN_156208858_275000_CN_107262429_275000/RConn3 -- T_156208858_500000_南相馬変電所/RConn3 -- L_156208858/LConn3 -- bus166/LConn1
  T_199544541_275000_新北信変電所/LConn1 -- _CN_199544541_275000_CN_211258348_275000/RConn1
  T_199544541_275000_新北信変電所/LConn2 -- _CN_199544541_275000_CN_211258348_275000/RConn2
  _CN_199544541_275000_CN_211258348_275000/RConn3 -- T_199544541_275000_新北信変電所/LConn3 -- bus167/LConn1
  _CN_161946848_275000_CN_190734269_275000/RConn1 -- T_190734269_275000_/LConn1 -- _CN_161870227_275000_CN_190734269_275000/LConn1
  _CN_161946848_275000_CN_190734269_275000/RConn2 -- T_190734269_275000_/LConn2 -- _CN_161870227_275000_CN_190734269_275000/LConn2
  _CN_161946848_275000_CN_190734269_275000/RConn3 -- T_190734269_275000_/LConn3 -- _CN_161870227_275000_CN_190734269_275000/LConn3 -- bus168/LConn1
  _CN_161946849_275000_CN_210658603_275000/RConn1 -- G_210658603_高根第一水力発電所/RConn1 -- _CN_315662816_275000_CN_210658603_275000/LConn1
  _CN_161946849_275000_CN_210658603_275000/RConn2 -- G_210658603_高根第一水力発電所/RConn2 -- _CN_315662816_275000_CN_210658603_275000/LConn2
  _CN_161946849_275000_CN_210658603_275000/RConn3 -- G_210658603_高根第一水力発電所/RConn3 -- _CN_315662816_275000_CN_210658603_275000/LConn3 -- bus169/LConn1
  河北1・2線_(Kahoku_1・2_Sen)_CN_133137636_275000_CN_133135172_275000/RConn1 -- T_133135172_500000_新古河変電所/RConn1 -- L_133135172/LConn1
  河北1・2線_(Kahoku_1・2_Sen)_CN_133137636_275000_CN_133135172_275000/RConn2 -- T_133135172_500000_新古河変電所/RConn2 -- L_133135172/LConn2
  河北1・2線_(Kahoku_1・2_Sen)_CN_133137636_275000_CN_133135172_275000/RConn3 -- T_133135172_500000_新古河変電所/RConn3 -- L_133135172/LConn3 -- bus170/LConn1
  東京北線_(Tōkyō_Kita_Sen)_CN_133137636_275000_CN_151706977_275000/RConn1 -- T_151706977__新野田変電所_(Shin_Noda_Hendensho)/RConn1 -- 新京葉線_CN_151706977_275000_CN_168852840_275000/RConn1 -- _CN_151706977_275000_CN_168727982_275000/LConn1 -- _CN_151706977_275000_CN_144077272_275000/LConn1 -- L_151706977/LConn1
  東京北線_(Tōkyō_Kita_Sen)_CN_133137636_275000_CN_151706977_275000/RConn2 -- T_151706977__新野田変電所_(Shin_Noda_Hendensho)/RConn2 -- 新京葉線_CN_151706977_275000_CN_168852840_275000/RConn2 -- _CN_151706977_275000_CN_168727982_275000/LConn2 -- _CN_151706977_275000_CN_144077272_275000/LConn2 -- L_151706977/LConn2
  東京北線_(Tōkyō_Kita_Sen)_CN_133137636_275000_CN_151706977_275000/RConn3 -- T_151706977__新野田変電所_(Shin_Noda_Hendensho)/RConn3 -- 新京葉線_CN_151706977_275000_CN_168852840_275000/RConn3 -- _CN_151706977_275000_CN_168727982_275000/LConn3 -- _CN_151706977_275000_CN_144077272_275000/LConn3 -- L_151706977/LConn3 -- bus171/LConn1
  G_180359727_川越火力発電所/RConn1 -- _CN_170793702_275000_CN_180359727_275000/RConn1
  G_180359727_川越火力発電所/RConn2 -- _CN_170793702_275000_CN_180359727_275000/RConn2
  _CN_170793702_275000_CN_180359727_275000/RConn3 -- G_180359727_川越火力発電所/RConn3 -- bus172/LConn1
  京浜線3;4号線_CN_128364781_275000_CN_47110637_275000/RConn1 -- T_47110637_275000_西東京変電所/LConn1 -- 東京西線_CN_145080115_275000_CN_47110637_275000/LConn1 -- 只見幹線_CN_153760214_275000_CN_47110637_275000/LConn1
  京浜線3;4号線_CN_128364781_275000_CN_47110637_275000/RConn2 -- T_47110637_275000_西東京変電所/LConn2 -- 東京西線_CN_145080115_275000_CN_47110637_275000/LConn2 -- 只見幹線_CN_153760214_275000_CN_47110637_275000/LConn2
  京浜線3;4号線_CN_128364781_275000_CN_47110637_275000/RConn3 -- T_47110637_275000_西東京変電所/LConn3 -- 東京西線_CN_145080115_275000_CN_47110637_275000/LConn3 -- 只見幹線_CN_153760214_275000_CN_47110637_275000/LConn3 -- bus173/LConn1
  G_379474501_/RConn1 -- 東京南線3;4号線_CN_128364781_275000_CN_379474501_275000/RConn1
  G_379474501_/RConn2 -- 東京南線3;4号線_CN_128364781_275000_CN_379474501_275000/RConn2
  東京南線3;4号線_CN_128364781_275000_CN_379474501_275000/RConn3 -- G_379474501_/RConn3 -- bus174/LConn1
  奥只見線_CN_250540807_275000_CN_232998815_275000/RConn1 -- T_250540807_500000_東群馬変電所_(Higashi_Gunma_Substation)/RConn1 -- L_250540807/LConn1
  奥只見線_CN_250540807_275000_CN_232998815_275000/RConn2 -- T_250540807_500000_東群馬変電所_(Higashi_Gunma_Substation)/RConn2 -- L_250540807/LConn2
  奥只見線_CN_250540807_275000_CN_232998815_275000/RConn3 -- T_250540807_500000_東群馬変電所_(Higashi_Gunma_Substation)/RConn3 -- L_250540807/LConn3 -- bus175/LConn1
  G_354115662_沼沢発電所/RConn1 -- _CN_250430935_275000_CN_354115662_275000/RConn1
  G_354115662_沼沢発電所/RConn2 -- _CN_250430935_275000_CN_354115662_275000/RConn2
  _CN_250430935_275000_CN_354115662_275000/RConn3 -- G_354115662_沼沢発電所/RConn3 -- bus176/LConn1
  T_291678103_275000_紀の川変電所_(Kinokawa_Hendensho)/LConn1 -- 金剛線_(Kongō_sen)_CN_109834508_275000_CN_291678103_275000/RConn1
  T_291678103_275000_紀の川変電所_(Kinokawa_Hendensho)/LConn2 -- 金剛線_(Kongō_sen)_CN_109834508_275000_CN_291678103_275000/RConn2
  金剛線_(Kongō_sen)_CN_109834508_275000_CN_291678103_275000/RConn3 -- T_291678103_275000_紀の川変電所_(Kinokawa_Hendensho)/LConn3 -- bus177/LConn1
  T_325868333_275000_/LConn1 -- _CN_325868333_275000_CN_110682951_275000/RConn1
  T_325868333_275000_/LConn2 -- _CN_325868333_275000_CN_110682951_275000/RConn2
  _CN_325868333_275000_CN_110682951_275000/RConn3 -- T_325868333_275000_/LConn3 -- bus178/LConn1
  T_145080115_275000_/LConn1 -- 東京西線_CN_145080115_275000_CN_47110637_275000/RConn1
  T_145080115_275000_/LConn2 -- 東京西線_CN_145080115_275000_CN_47110637_275000/RConn2
  東京西線_CN_145080115_275000_CN_47110637_275000/RConn3 -- T_145080115_275000_/LConn3 -- bus179/LConn1
  T_308348224_275000_新庄変電所/LConn1 -- _CN_106076988_275000_CN_308348224_275000/RConn1
  T_308348224_275000_新庄変電所/LConn2 -- _CN_106076988_275000_CN_308348224_275000/RConn2
  _CN_106076988_275000_CN_308348224_275000/RConn3 -- T_308348224_275000_新庄変電所/LConn3 -- bus180/LConn1
  _CN_110682951_275000_CN_110682956_275000/RConn1 -- T_110682956_500000_猪名川変電所/RConn1 -- L_110682956/LConn1
  _CN_110682951_275000_CN_110682956_275000/RConn2 -- T_110682956_500000_猪名川変電所/RConn2 -- L_110682956/LConn2
  _CN_110682951_275000_CN_110682956_275000/RConn3 -- T_110682956_500000_猪名川変電所/RConn3 -- L_110682956/LConn3 -- bus181/LConn1
  T_110682955_275000;154000;77000_伊丹変電所_(Itami_Hendensho)/LConn1 -- _CN_110682951_275000_CN_110682955_275000/RConn1
  T_110682955_275000;154000;77000_伊丹変電所_(Itami_Hendensho)/LConn2 -- _CN_110682951_275000_CN_110682955_275000/RConn2
  _CN_110682951_275000_CN_110682955_275000/RConn3 -- T_110682955_275000;154000;77000_伊丹変電所_(Itami_Hendensho)/LConn3 -- bus182/LConn1
  T_320724312_275000_/LConn1 -- _CN_320724312_275000_CN_317416612_275000/LConn1
  T_320724312_275000_/LConn2 -- _CN_320724312_275000_CN_317416612_275000/LConn2
  _CN_320724312_275000_CN_317416612_275000/LConn3 -- T_320724312_275000_/LConn3 -- bus183/LConn1
  _CN_320724312_275000_CN_317416612_275000/RConn1 -- T_317416612_500000_西島根変電所/RConn1 -- L_317416612/LConn1
  _CN_320724312_275000_CN_317416612_275000/RConn2 -- T_317416612_500000_西島根変電所/RConn2 -- L_317416612/LConn2
  _CN_320724312_275000_CN_317416612_275000/RConn3 -- T_317416612_500000_西島根変電所/RConn3 -- L_317416612/LConn3 -- bus184/LConn1
  T_316459359_275000_/LConn1 -- _CN_316459359_275000_CN_107262429_275000/RConn1
  T_316459359_275000_/LConn2 -- _CN_316459359_275000_CN_107262429_275000/RConn2
  _CN_316459359_275000_CN_107262429_275000/RConn3 -- T_316459359_275000_/LConn3 -- bus185/LConn1
  _CN_151706977_275000_CN_168727982_275000/RConn1 -- T_168727982_500000_新京葉変電所/RConn1 -- L_168727982/LConn1
  _CN_151706977_275000_CN_168727982_275000/RConn2 -- T_168727982_500000_新京葉変電所/RConn2 -- L_168727982/LConn2
  _CN_151706977_275000_CN_168727982_275000/RConn3 -- T_168727982_500000_新京葉変電所/RConn3 -- L_168727982/LConn3 -- bus186/LConn1
  T_144077272__/LConn1 -- _CN_151706977_275000_CN_144077272_275000/RConn1
  T_144077272__/LConn2 -- _CN_151706977_275000_CN_144077272_275000/RConn2
  _CN_151706977_275000_CN_144077272_275000/RConn3 -- T_144077272__/LConn3 -- bus187/LConn1
  _CN_106309481_275000_CN_103783431_275000/LConn1 -- T_106309481_500000_新福島変電所/RConn1 -- L_106309481/LConn1
  _CN_106309481_275000_CN_103783431_275000/LConn2 -- T_106309481_500000_新福島変電所/RConn2 -- L_106309481/LConn2
  _CN_106309481_275000_CN_103783431_275000/LConn3 -- T_106309481_500000_新福島変電所/RConn3 -- L_106309481/LConn3 -- bus188/LConn1
  _CN_106309481_275000_CN_103783431_275000/RConn1 -- G_103783431_福島第一_原子力発電所/RConn1 -- _CN_106309481_500000_CN_103783431_275000/LConn1
  _CN_106309481_275000_CN_103783431_275000/RConn2 -- G_103783431_福島第一_原子力発電所/RConn2 -- _CN_106309481_500000_CN_103783431_275000/LConn2
  _CN_106309481_275000_CN_103783431_275000/RConn3 -- G_103783431_福島第一_原子力発電所/RConn3 -- _CN_106309481_500000_CN_103783431_275000/LConn3 -- bus189/LConn1
  中東京幹線_CN_315434352_275000_CN_152991099_275000/RConn1 -- T_152991099__中東京変電所/LConn1 -- 中沢線3;4号線_CN_152991099_275000_CN_133641619_275000/RConn1
  中東京幹線_CN_315434352_275000_CN_152991099_275000/RConn2 -- T_152991099__中東京変電所/LConn2 -- 中沢線3;4号線_CN_152991099_275000_CN_133641619_275000/RConn2
  中東京幹線_CN_315434352_275000_CN_152991099_275000/RConn3 -- T_152991099__中東京変電所/LConn3 -- 中沢線3;4号線_CN_152991099_275000_CN_133641619_275000/RConn3 -- bus190/LConn1
  _CN_161870227_275000_CN_190734269_275000/RConn1 -- T_161870227_500000_南京都変電所_(Minami_Kyōto_Hendensho)/RConn1 -- _CN_161870227_275000_CN_191382966_275000/LConn1 -- L_161870227/LConn1
  _CN_161870227_275000_CN_190734269_275000/RConn2 -- T_161870227_500000_南京都変電所_(Minami_Kyōto_Hendensho)/RConn2 -- _CN_161870227_275000_CN_191382966_275000/LConn2 -- L_161870227/LConn2
  _CN_161870227_275000_CN_190734269_275000/RConn3 -- T_161870227_500000_南京都変電所_(Minami_Kyōto_Hendensho)/RConn3 -- _CN_161870227_275000_CN_191382966_275000/LConn3 -- L_161870227/LConn3 -- bus191/LConn1
  _CN_161870227_275000_CN_191382966_275000/RConn1 -- G_191382966_喜撰山水力発電所/RConn1 -- _CN_190984572_275000_CN_191382966_275000/LConn1
  _CN_161870227_275000_CN_191382966_275000/RConn2 -- G_191382966_喜撰山水力発電所/RConn2 -- _CN_190984572_275000_CN_191382966_275000/LConn2
  _CN_161870227_275000_CN_191382966_275000/RConn3 -- G_191382966_喜撰山水力発電所/RConn3 -- _CN_190984572_275000_CN_191382966_275000/LConn3 -- bus192/LConn1
  T_190984572_275000_/LConn1 -- _CN_190984572_275000_CN_191382966_275000/RConn1
  T_190984572_275000_/LConn2 -- _CN_190984572_275000_CN_191382966_275000/RConn2
  _CN_190984572_275000_CN_191382966_275000/RConn3 -- T_190984572_275000_/LConn3 -- bus193/LConn1
  G_233174201_/RConn1 -- _CN_232998815_275000_CN_233174201_275000/RConn1
  G_233174201_/RConn2 -- _CN_232998815_275000_CN_233174201_275000/RConn2
  _CN_232998815_275000_CN_233174201_275000/RConn3 -- G_233174201_/RConn3 -- bus194/LConn1
  T_318302348_275000_東上越変電所/LConn1 -- _CN_318302348_275000_CN_319098734_275000/RConn1
  T_318302348_275000_東上越変電所/LConn2 -- _CN_318302348_275000_CN_319098734_275000/RConn2
  _CN_318302348_275000_CN_319098734_275000/RConn3 -- T_318302348_275000_東上越変電所/LConn3 -- bus195/LConn1
  T_153760214__多摩変電所/LConn1 -- 只見幹線_CN_153760214_275000_CN_47110637_275000/RConn1
  T_153760214__多摩変電所/LConn2 -- 只見幹線_CN_153760214_275000_CN_47110637_275000/RConn2
  只見幹線_CN_153760214_275000_CN_47110637_275000/RConn3 -- T_153760214__多摩変電所/LConn3 -- bus196/LConn1
  T_315662816__/LConn1 -- _CN_315662816_275000_CN_210658603_275000/RConn1
  T_315662816__/LConn2 -- _CN_315662816_275000_CN_210658603_275000/RConn2
  _CN_315662816_275000_CN_210658603_275000/RConn3 -- T_315662816__/LConn3 -- bus197/LConn1
  G_242706111_/RConn1 -- _CN_241822631_275000_CN_242706111_275000/RConn1
  G_242706111_/RConn2 -- _CN_241822631_275000_CN_242706111_275000/RConn2
  _CN_241822631_275000_CN_242706111_275000/RConn3 -- G_242706111_/RConn3 -- bus198/LConn1
  G_110340505_新神戸変電所/RConn1 -- _CN_185032690_275000_CN_110340505_275000/RConn1
  G_110340505_新神戸変電所/RConn2 -- _CN_185032690_275000_CN_110340505_275000/RConn2
  _CN_185032690_275000_CN_110340505_275000/RConn3 -- G_110340505_新神戸変電所/RConn3 -- bus199/LConn1
  _CN_201293312_500000_CN_216778426_500000/LConn1 -- T_201293312_500000;220000_/LConn1 -- _CN_201293312_500000_CN_187988970_500000/LConn1
  _CN_201293312_500000_CN_216778426_500000/LConn2 -- T_201293312_500000;220000_/LConn2 -- _CN_201293312_500000_CN_187988970_500000/LConn2
  _CN_201293312_500000_CN_216778426_500000/LConn3 -- T_201293312_500000;220000_/LConn3 -- _CN_201293312_500000_CN_187988970_500000/LConn3 -- bus200/LConn1
  T_216778426_500000;220000_/LConn1 -- _CN_201293312_500000_CN_216778426_500000/RConn1
  T_216778426_500000;220000_/LConn2 -- _CN_201293312_500000_CN_216778426_500000/RConn2
  _CN_201293312_500000_CN_216778426_500000/RConn3 -- T_216778426_500000;220000_/LConn3 -- bus201/LConn1
  _CN_201293312_500000_CN_187988970_500000/RConn1 -- T_187988970_500000;220000_/LConn1 -- 関門連系線_CN_204258596_500000_CN_187988970_500000/LConn1
  _CN_201293312_500000_CN_187988970_500000/RConn2 -- T_187988970_500000;220000_/LConn2 -- 関門連系線_CN_204258596_500000_CN_187988970_500000/LConn2
  _CN_201293312_500000_CN_187988970_500000/RConn3 -- T_187988970_500000;220000_/LConn3 -- 関門連系線_CN_204258596_500000_CN_187988970_500000/LConn3 -- bus202/LConn1
  T_104173570_500000_/LConn1 -- _CN_104173570_500000_CN_106309481_500000/LConn1
  T_104173570_500000_/LConn2 -- _CN_104173570_500000_CN_106309481_500000/LConn2
  _CN_104173570_500000_CN_106309481_500000/LConn3 -- T_104173570_500000_/LConn3 -- bus203/LConn1
  _CN_104173570_500000_CN_106309481_500000/RConn1 -- T_106309481_500000_新福島変電所/LConn1 -- _CN_106309481_500000_CN_103783431_275000/RConn1 -- 福島東幹線2_CN_106309481_500000_CN_104391636_500000/LConn1
  _CN_104173570_500000_CN_106309481_500000/RConn2 -- T_106309481_500000_新福島変電所/LConn2 -- _CN_106309481_500000_CN_103783431_275000/RConn2 -- 福島東幹線2_CN_106309481_500000_CN_104391636_500000/LConn2
  _CN_104173570_500000_CN_106309481_500000/RConn3 -- T_106309481_500000_新福島変電所/LConn3 -- _CN_106309481_500000_CN_103783431_275000/RConn3 -- 福島東幹線2_CN_106309481_500000_CN_104391636_500000/LConn3 -- bus204/LConn1
  T_168857610__/LConn1 -- _CN_168857610_500000_CN_104530060_500000/LConn1
  T_168857610__/LConn2 -- _CN_168857610_500000_CN_104530060_500000/LConn2
  _CN_168857610_500000_CN_104530060_500000/LConn3 -- T_168857610__/LConn3 -- bus205/LConn1
  _CN_168857610_500000_CN_104530060_500000/RConn1 -- T_104530060__新栃木変電所/LConn1 -- 新茂木線_(Shin_Motegi_Sen)_CN_104530060_500000_CN_168839127_500000/LConn1
  _CN_168857610_500000_CN_104530060_500000/RConn2 -- T_104530060__新栃木変電所/LConn2 -- 新茂木線_(Shin_Motegi_Sen)_CN_104530060_500000_CN_168839127_500000/LConn2
  _CN_168857610_500000_CN_104530060_500000/RConn3 -- T_104530060__新栃木変電所/LConn3 -- 新茂木線_(Shin_Motegi_Sen)_CN_104530060_500000_CN_168839127_500000/LConn3 -- bus206/LConn1
  _CN_87538349_500000_CN_171066843_500000/LConn1 -- T_87538349_500000_讃岐変電所/LConn1 -- _CN_87538349_500000_CN_102958903_500000/LConn1
  _CN_87538349_500000_CN_171066843_500000/LConn2 -- T_87538349_500000_讃岐変電所/LConn2 -- _CN_87538349_500000_CN_102958903_500000/LConn2
  _CN_87538349_500000_CN_171066843_500000/LConn3 -- T_87538349_500000_讃岐変電所/LConn3 -- _CN_87538349_500000_CN_102958903_500000/LConn3 -- bus207/LConn1
  T_171066843_500000_四国電力東予変電所/LConn1 -- _CN_87538349_500000_CN_171066843_500000/RConn1
  T_171066843_500000_四国電力東予変電所/LConn2 -- _CN_87538349_500000_CN_171066843_500000/RConn2
  _CN_87538349_500000_CN_171066843_500000/RConn3 -- T_171066843_500000_四国電力東予変電所/LConn3 -- bus208/LConn1
  T_102958903_500000_/LConn1 -- _CN_87538349_500000_CN_102958903_500000/RConn1
  T_102958903_500000_/LConn2 -- _CN_87538349_500000_CN_102958903_500000/RConn2
  _CN_87538349_500000_CN_102958903_500000/RConn3 -- T_102958903_500000_/LConn3 -- bus209/LConn1
  南九州幹線_CN_216502300_500000_CN_215451416_500000/LConn1 -- T_216502300__九州電力_中九州変電所/LConn1 -- 中九州幹線_CN_216502300_500000_CN_405626236_500000/LConn1
  南九州幹線_CN_216502300_500000_CN_215451416_500000/LConn2 -- T_216502300__九州電力_中九州変電所/LConn2 -- 中九州幹線_CN_216502300_500000_CN_405626236_500000/LConn2
  南九州幹線_CN_216502300_500000_CN_215451416_500000/LConn3 -- T_216502300__九州電力_中九州変電所/LConn3 -- 中九州幹線_CN_216502300_500000_CN_405626236_500000/LConn3 -- bus210/LConn1
  南九州幹線_CN_216502300_500000_CN_215451416_500000/RConn1 -- T_215451416_500000;220000_九州電力南九州変電所/LConn1 -- _CN_215451416_500000_CN_215429864_220000/RConn1
  南九州幹線_CN_216502300_500000_CN_215451416_500000/RConn2 -- T_215451416_500000;220000_九州電力南九州変電所/LConn2 -- _CN_215451416_500000_CN_215429864_220000/RConn2
  南九州幹線_CN_216502300_500000_CN_215451416_500000/RConn3 -- T_215451416_500000;220000_九州電力南九州変電所/LConn3 -- _CN_215451416_500000_CN_215429864_220000/RConn3 -- bus211/LConn1
  T_405626236_220000_熊本変電所/LConn1 -- 中九州幹線_CN_216502300_500000_CN_405626236_500000/RConn1
  T_405626236_220000_熊本変電所/LConn2 -- 中九州幹線_CN_216502300_500000_CN_405626236_500000/RConn2
  中九州幹線_CN_216502300_500000_CN_405626236_500000/RConn3 -- T_405626236_220000_熊本変電所/LConn3 -- bus212/LConn1
  新多摩線_(Shin_Tama_Sen)_CN_149843487_500000_CN_145079972_500000/LConn1 -- T_149843487_500000_新秦野変電所_(Shin_Hatano_Hendensho)/LConn1 -- _CN_149843487_500000_CN_150065045_500000/LConn1
  新多摩線_(Shin_Tama_Sen)_CN_149843487_500000_CN_145079972_500000/LConn2 -- T_149843487_500000_新秦野変電所_(Shin_Hatano_Hendensho)/LConn2 -- _CN_149843487_500000_CN_150065045_500000/LConn2
  新多摩線_(Shin_Tama_Sen)_CN_149843487_500000_CN_145079972_500000/LConn3 -- T_149843487_500000_新秦野変電所_(Shin_Hatano_Hendensho)/LConn3 -- _CN_149843487_500000_CN_150065045_500000/LConn3 -- bus213/LConn1
  新多摩線_(Shin_Tama_Sen)_CN_149843487_500000_CN_145079972_500000/RConn1 -- T_145079972_500000_新多摩変電所_(Shin_Tama_Substation)/LConn1 -- 新所沢線_(Shin_Tokorozawa_Sen)_CN_145079972_500000_CN_133641619_500000/LConn1
  新多摩線_(Shin_Tama_Sen)_CN_149843487_500000_CN_145079972_500000/RConn2 -- T_145079972_500000_新多摩変電所_(Shin_Tama_Substation)/LConn2 -- 新所沢線_(Shin_Tokorozawa_Sen)_CN_145079972_500000_CN_133641619_500000/LConn2
  新多摩線_(Shin_Tama_Sen)_CN_149843487_500000_CN_145079972_500000/RConn3 -- T_145079972_500000_新多摩変電所_(Shin_Tama_Substation)/LConn3 -- 新所沢線_(Shin_Tokorozawa_Sen)_CN_145079972_500000_CN_133641619_500000/LConn3 -- bus214/LConn1
  _CN_149843487_500000_CN_150065045_500000/RConn1 -- T_150065045_500000_新富士変電所/LConn1 -- _CN_150035494_500000_CN_150065045_500000/LConn1
  _CN_149843487_500000_CN_150065045_500000/RConn2 -- T_150065045_500000_新富士変電所/LConn2 -- _CN_150035494_500000_CN_150065045_500000/LConn2
  _CN_149843487_500000_CN_150065045_500000/RConn3 -- T_150065045_500000_新富士変電所/LConn3 -- _CN_150035494_500000_CN_150065045_500000/LConn3 -- bus215/LConn1
  _CN_150035494_500000_CN_341208725_500000/LConn1 -- T_150035494_500000_/LConn1 -- _CN_150035494_500000_CN_150065045_500000/RConn1 -- _CN_150035494_500000_CN_66098469_500000/LConn1 -- _CN_150035494_500000_CN_216480979_500000/LConn1
  _CN_150035494_500000_CN_341208725_500000/LConn2 -- T_150035494_500000_/LConn2 -- _CN_150035494_500000_CN_150065045_500000/RConn2 -- _CN_150035494_500000_CN_66098469_500000/LConn2 -- _CN_150035494_500000_CN_216480979_500000/LConn2
  _CN_150035494_500000_CN_341208725_500000/LConn3 -- T_150035494_500000_/LConn3 -- _CN_150035494_500000_CN_150065045_500000/RConn3 -- _CN_150035494_500000_CN_66098469_500000/LConn3 -- _CN_150035494_500000_CN_216480979_500000/LConn3 -- bus216/LConn1
  T_341208725__/LConn1 -- _CN_150035494_500000_CN_341208725_500000/RConn1
  T_341208725__/LConn2 -- _CN_150035494_500000_CN_341208725_500000/RConn2
  _CN_150035494_500000_CN_341208725_500000/RConn3 -- T_341208725__/LConn3 -- bus217/LConn1
  _CN_150035494_500000_CN_66098469_500000/RConn1 -- T_66098469_500000_西群馬開閉所/LConn1 -- 東群馬幹線_CN_250540807_500000_CN_66098469_500000/LConn1 -- _CN_66098469_500000_CN_216480979_500000/LConn1 -- 新吾妻線_CN_169963236_500000_CN_66098469_500000/LConn1
  _CN_150035494_500000_CN_66098469_500000/RConn2 -- T_66098469_500000_西群馬開閉所/LConn2 -- 東群馬幹線_CN_250540807_500000_CN_66098469_500000/LConn2 -- _CN_66098469_500000_CN_216480979_500000/LConn2 -- 新吾妻線_CN_169963236_500000_CN_66098469_500000/LConn2
  _CN_150035494_500000_CN_66098469_500000/RConn3 -- T_66098469_500000_西群馬開閉所/LConn3 -- 東群馬幹線_CN_250540807_500000_CN_66098469_500000/LConn3 -- _CN_66098469_500000_CN_216480979_500000/LConn3 -- bus218/LConn1 -- 新吾妻線_CN_169963236_500000_CN_66098469_500000/LConn3
  _CN_150035494_500000_CN_216480979_500000/RConn1 -- G_216480979_柏崎刈羽原子力発電所/RConn1 -- _CN_66098469_500000_CN_216480979_500000/RConn1
  _CN_150035494_500000_CN_216480979_500000/RConn2 -- G_216480979_柏崎刈羽原子力発電所/RConn2 -- _CN_66098469_500000_CN_216480979_500000/RConn2
  _CN_150035494_500000_CN_216480979_500000/RConn3 -- G_216480979_柏崎刈羽原子力発電所/RConn3 -- _CN_66098469_500000_CN_216480979_500000/RConn3 -- bus219/LConn1
  _CN_170589736_500000_CN_161870227_500000/LConn1 -- T_170589736_500000_東近江/LConn1 -- _CN_170589736_500000_CN_170568495_500000/LConn1
  _CN_170589736_500000_CN_161870227_500000/LConn2 -- T_170589736_500000_東近江/LConn2 -- _CN_170589736_500000_CN_170568495_500000/LConn2
  _CN_170589736_500000_CN_161870227_500000/LConn3 -- T_170589736_500000_東近江/LConn3 -- _CN_170589736_500000_CN_170568495_500000/LConn3 -- bus220/LConn1
  _CN_170589736_500000_CN_161870227_500000/RConn1 -- T_161870227_500000_南京都変電所_(Minami_Kyōto_Hendensho)/LConn1 -- _CN_161727149_500000_CN_161870227_500000/LConn1 -- _CN_169031998_500000_CN_161870227_500000/LConn1
  _CN_170589736_500000_CN_161870227_500000/RConn2 -- T_161870227_500000_南京都変電所_(Minami_Kyōto_Hendensho)/LConn2 -- _CN_161727149_500000_CN_161870227_500000/LConn2 -- _CN_169031998_500000_CN_161870227_500000/LConn2
  _CN_170589736_500000_CN_161870227_500000/RConn3 -- T_161870227_500000_南京都変電所_(Minami_Kyōto_Hendensho)/LConn3 -- _CN_161727149_500000_CN_161870227_500000/LConn3 -- _CN_169031998_500000_CN_161870227_500000/LConn3 -- bus221/LConn1
  _CN_170589736_500000_CN_170568495_500000/RConn1 -- T_170568495_500000_三重開閉所/LConn1 -- _CN_170537514_500000_CN_170568495_500000/LConn1 -- _CN_170366035_500000_CN_170568495_500000/LConn1
  _CN_170589736_500000_CN_170568495_500000/RConn2 -- T_170568495_500000_三重開閉所/LConn2 -- _CN_170537514_500000_CN_170568495_500000/LConn2 -- _CN_170366035_500000_CN_170568495_500000/LConn2
  _CN_170589736_500000_CN_170568495_500000/RConn3 -- T_170568495_500000_三重開閉所/LConn3 -- _CN_170537514_500000_CN_170568495_500000/LConn3 -- _CN_170366035_500000_CN_170568495_500000/LConn3 -- bus222/LConn1
  _CN_170537514_500000_CN_161946849_500000/LConn1 -- T_170537514_500000_/LConn1 -- _CN_170537514_500000_CN_170568495_500000/RConn1
  _CN_170537514_500000_CN_161946849_500000/LConn2 -- T_170537514_500000_/LConn2 -- _CN_170537514_500000_CN_170568495_500000/RConn2
  _CN_170537514_500000_CN_161946849_500000/LConn3 -- T_170537514_500000_/LConn3 -- _CN_170537514_500000_CN_170568495_500000/RConn3 -- bus223/LConn1
  _CN_170537514_500000_CN_161946849_500000/RConn1 -- T_161946849_500000;275000_北部変電所/LConn1 -- _CN_169122898_500000_CN_161946849_500000/LConn1 -- _CN_170366035_500000_CN_161946849_500000/LConn1
  _CN_170537514_500000_CN_161946849_500000/RConn2 -- T_161946849_500000;275000_北部変電所/LConn2 -- _CN_169122898_500000_CN_161946849_500000/LConn2 -- _CN_170366035_500000_CN_161946849_500000/LConn2
  _CN_170537514_500000_CN_161946849_500000/RConn3 -- T_161946849_500000;275000_北部変電所/LConn3 -- _CN_169122898_500000_CN_161946849_500000/LConn3 -- _CN_170366035_500000_CN_161946849_500000/LConn3 -- bus224/LConn1
  T_116559939_500000_/LConn1 -- 駿遠幹線_CN_116559939_500000_CN_210090094_500000/LConn1
  T_116559939_500000_/LConn2 -- 駿遠幹線_CN_116559939_500000_CN_210090094_500000/LConn2
  駿遠幹線_CN_116559939_500000_CN_210090094_500000/LConn3 -- T_116559939_500000_/LConn3 -- bus225/LConn1
  T_210090094_500000_駿遠変電所/LConn1 -- 駿遠幹線_CN_116559939_500000_CN_210090094_500000/RConn1
  T_210090094_500000_駿遠変電所/LConn2 -- 駿遠幹線_CN_116559939_500000_CN_210090094_500000/RConn2
  駿遠幹線_CN_116559939_500000_CN_210090094_500000/RConn3 -- T_210090094_500000_駿遠変電所/LConn3 -- bus226/LConn1
  T_172601929_500000;220000_/LConn1 -- _CN_172601929_500000_CN_172644773_220000/RConn1
  T_172601929_500000;220000_/LConn2 -- _CN_172601929_500000_CN_172644773_220000/RConn2
  _CN_172601929_500000_CN_172644773_220000/RConn3 -- T_172601929_500000;220000_/LConn3 -- bus227/LConn1
  _CN_169122898_500000_CN_161946849_500000/RConn1 -- T_169122898_500000_東部変電所/LConn1 -- _CN_169122898_500000_CN_142662111_500000/LConn1 -- _CN_169122898_500000_CN_170247312_500000/LConn1
  _CN_169122898_500000_CN_161946849_500000/RConn2 -- T_169122898_500000_東部変電所/LConn2 -- _CN_169122898_500000_CN_142662111_500000/LConn2 -- _CN_169122898_500000_CN_170247312_500000/LConn2
  _CN_169122898_500000_CN_161946849_500000/RConn3 -- T_169122898_500000_東部変電所/LConn3 -- _CN_169122898_500000_CN_142662111_500000/LConn3 -- bus228/LConn1 -- _CN_169122898_500000_CN_170247312_500000/LConn3
  T_170247312_500000_新三河変電所/LConn1 -- _CN_169122898_500000_CN_170247312_500000/RConn1
  T_170247312_500000_新三河変電所/LConn2 -- _CN_169122898_500000_CN_170247312_500000/RConn2
  _CN_169122898_500000_CN_170247312_500000/RConn3 -- T_170247312_500000_新三河変電所/LConn3 -- bus229/LConn1
  _CN_169122898_500000_CN_142662111_500000/RConn1 -- T_142662111_500000_中部電力㈱豊根開閉所/LConn1 -- 豊根幹線_CN_142662111_500000_CN_170850727_500000/LConn1 -- 南信幹線_CN_142662111_500000_CN_209429410_500000/LConn1
  _CN_169122898_500000_CN_142662111_500000/RConn2 -- T_142662111_500000_中部電力㈱豊根開閉所/LConn2 -- 豊根幹線_CN_142662111_500000_CN_170850727_500000/LConn2 -- 南信幹線_CN_142662111_500000_CN_209429410_500000/LConn2
  _CN_169122898_500000_CN_142662111_500000/RConn3 -- T_142662111_500000_中部電力㈱豊根開閉所/LConn3 -- 豊根幹線_CN_142662111_500000_CN_170850727_500000/LConn3 -- 南信幹線_CN_142662111_500000_CN_209429410_500000/LConn3 -- bus230/LConn1
  _CN_170366035_500000_CN_170568495_500000/RConn1 -- T_170366035_500000_/LConn1 -- _CN_170366035_500000_CN_170850727_500000/LConn1 -- _CN_170366035_500000_CN_161946849_500000/RConn1
  _CN_170366035_500000_CN_170568495_500000/RConn2 -- T_170366035_500000_/LConn2 -- _CN_170366035_500000_CN_170850727_500000/LConn2 -- _CN_170366035_500000_CN_161946849_500000/RConn2
  _CN_170366035_500000_CN_170568495_500000/RConn3 -- T_170366035_500000_/LConn3 -- _CN_170366035_500000_CN_170850727_500000/LConn3 -- _CN_170366035_500000_CN_161946849_500000/RConn3 -- bus231/LConn1
  _CN_170366035_500000_CN_170850727_500000/RConn1 -- T_170850727_500000_愛知変電所/LConn1 -- 豊根幹線_CN_142662111_500000_CN_170850727_500000/RConn1
  _CN_170366035_500000_CN_170850727_500000/RConn2 -- T_170850727_500000_愛知変電所/LConn2 -- 豊根幹線_CN_142662111_500000_CN_170850727_500000/RConn2
  _CN_170366035_500000_CN_170850727_500000/RConn3 -- T_170850727_500000_愛知変電所/LConn3 -- 豊根幹線_CN_142662111_500000_CN_170850727_500000/RConn3 -- bus232/LConn1
  _CN_193544791_500000_CN_170974371_500000/LConn1 -- T_193544791_500000_新西広島変電所_(Shin_Nishi_Hiroshima_Hendensho)/LConn1 -- _CN_193544791_500000_CN_242253500_500000/LConn1 -- _CN_193544791_500000_CN_317416612_500000/LConn1
  _CN_193544791_500000_CN_170974371_500000/LConn2 -- T_193544791_500000_新西広島変電所_(Shin_Nishi_Hiroshima_Hendensho)/LConn2 -- _CN_193544791_500000_CN_242253500_500000/LConn2 -- _CN_193544791_500000_CN_317416612_500000/LConn2
  _CN_193544791_500000_CN_170974371_500000/LConn3 -- T_193544791_500000_新西広島変電所_(Shin_Nishi_Hiroshima_Hendensho)/LConn3 -- _CN_193544791_500000_CN_242253500_500000/LConn3 -- _CN_193544791_500000_CN_317416612_500000/LConn3 -- bus233/LConn1
  _CN_193544791_500000_CN_170974371_500000/RConn1 -- T_170974371_500000_新広島変電所_(Shin_Hiroshima_Hendensho)/LConn1 -- _CN_170974371_500000_CN_241828221_500000/LConn1
  _CN_193544791_500000_CN_170974371_500000/RConn2 -- T_170974371_500000_新広島変電所_(Shin_Hiroshima_Hendensho)/LConn2 -- _CN_170974371_500000_CN_241828221_500000/LConn2
  _CN_193544791_500000_CN_170974371_500000/RConn3 -- T_170974371_500000_新広島変電所_(Shin_Hiroshima_Hendensho)/LConn3 -- _CN_170974371_500000_CN_241828221_500000/LConn3 -- bus234/LConn1
  _CN_193544791_500000_CN_242253500_500000/RConn1 -- T_242253500_500000_東山口変電所_(Higashi_Yamaguchi_Hendensho)/LConn1 -- _CN_242253500_500000_CN_204258596_500000/LConn1
  _CN_193544791_500000_CN_242253500_500000/RConn2 -- T_242253500_500000_東山口変電所_(Higashi_Yamaguchi_Hendensho)/LConn2 -- _CN_242253500_500000_CN_204258596_500000/LConn2
  _CN_193544791_500000_CN_242253500_500000/RConn3 -- T_242253500_500000_東山口変電所_(Higashi_Yamaguchi_Hendensho)/LConn3 -- _CN_242253500_500000_CN_204258596_500000/LConn3 -- bus235/LConn1
  _CN_193544791_500000_CN_317416612_500000/RConn1 -- T_317416612_500000_西島根変電所/LConn1 -- _CN_204258596_500000_CN_317416612_500000/LConn1 -- _CN_242103481_500000_CN_317416612_500000/LConn1
  _CN_193544791_500000_CN_317416612_500000/RConn2 -- T_317416612_500000_西島根変電所/LConn2 -- _CN_204258596_500000_CN_317416612_500000/LConn2 -- _CN_242103481_500000_CN_317416612_500000/LConn2
  _CN_193544791_500000_CN_317416612_500000/RConn3 -- T_317416612_500000_西島根変電所/LConn3 -- _CN_204258596_500000_CN_317416612_500000/LConn3 -- bus236/LConn1 -- _CN_242103481_500000_CN_317416612_500000/LConn3
  _CN_242253537_500000_CN_242103481_500000/LConn1 -- T_242253537__開閉所/LConn1 -- _CN_242253537_500000_CN_241822621_500000/LConn1
  _CN_242253537_500000_CN_242103481_500000/LConn2 -- T_242253537__開閉所/LConn2 -- _CN_242253537_500000_CN_241822621_500000/LConn2
  _CN_242253537_500000_CN_242103481_500000/LConn3 -- T_242253537__開閉所/LConn3 -- _CN_242253537_500000_CN_241822621_500000/LConn3 -- bus237/LConn1
  _CN_242253537_500000_CN_242103481_500000/RConn1 -- T_242103481_500000_日野変電所/LConn1 -- _CN_242103481_500000_CN_317416612_500000/RConn1 -- _CN_242103481_500000_CN_241828221_500000/LConn1 -- _CN_242103481_500000_CN_317511904_500000/LConn1
  _CN_242253537_500000_CN_242103481_500000/RConn2 -- T_242103481_500000_日野変電所/LConn2 -- _CN_242103481_500000_CN_317416612_500000/RConn2 -- _CN_242103481_500000_CN_241828221_500000/LConn2 -- _CN_242103481_500000_CN_317511904_500000/LConn2
  _CN_242253537_500000_CN_242103481_500000/RConn3 -- T_242103481_500000_日野変電所/LConn3 -- _CN_242103481_500000_CN_317416612_500000/RConn3 -- _CN_242103481_500000_CN_241828221_500000/LConn3 -- _CN_242103481_500000_CN_317511904_500000/LConn3 -- bus238/LConn1
  _CN_242253537_500000_CN_241822621_500000/RConn1 -- T_241822621_500000_/LConn1 -- _CN_241822621_500000_CN_241822631_500000/LConn1 -- _CN_320438391_500000_CN_241822621_500000/LConn1
  _CN_242253537_500000_CN_241822621_500000/RConn2 -- T_241822621_500000_/LConn2 -- _CN_241822621_500000_CN_241822631_500000/LConn2 -- _CN_320438391_500000_CN_241822621_500000/LConn2
  _CN_242253537_500000_CN_241822621_500000/RConn3 -- T_241822621_500000_/LConn3 -- _CN_241822621_500000_CN_241822631_500000/LConn3 -- bus239/LConn1 -- _CN_320438391_500000_CN_241822621_500000/LConn3
  _CN_320438391_500000_CN_241822621_500000/RConn1 -- T_320438391_500000_/LConn1 -- _CN_320438391_500000_CN_169031921_500000/LConn1 -- _CN_320438391_500000_CN_110682956_500000/LConn1 -- _CN_320438391_500000_CN_320444665_500000/LConn1
  _CN_320438391_500000_CN_241822621_500000/RConn2 -- T_320438391_500000_/LConn2 -- _CN_320438391_500000_CN_169031921_500000/LConn2 -- _CN_320438391_500000_CN_110682956_500000/LConn2 -- _CN_320438391_500000_CN_320444665_500000/LConn2
  _CN_320438391_500000_CN_241822621_500000/RConn3 -- T_320438391_500000_/LConn3 -- _CN_320438391_500000_CN_169031921_500000/LConn3 -- bus240/LConn1 -- _CN_320438391_500000_CN_110682956_500000/LConn3 -- _CN_320438391_500000_CN_320444665_500000/LConn3
  _CN_320438391_500000_CN_110682956_500000/RConn1 -- T_110682956_500000_猪名川変電所/LConn1 -- _CN_170605907_500000_CN_110682956_500000/LConn1
  _CN_320438391_500000_CN_110682956_500000/RConn2 -- T_110682956_500000_猪名川変電所/LConn2 -- _CN_170605907_500000_CN_110682956_500000/LConn2
  _CN_320438391_500000_CN_110682956_500000/RConn3 -- T_110682956_500000_猪名川変電所/LConn3 -- _CN_170605907_500000_CN_110682956_500000/LConn3 -- bus241/LConn1
  T_320444665_500000_/LConn1 -- _CN_320438391_500000_CN_320444665_500000/RConn1
  T_320444665_500000_/LConn2 -- _CN_320438391_500000_CN_320444665_500000/RConn2
  _CN_320438391_500000_CN_320444665_500000/RConn3 -- T_320444665_500000_/LConn3 -- bus242/LConn1
  _CN_320438391_500000_CN_169031921_500000/RConn1 -- T_169031921_500000_西京都変電所_(Nishi_Kyōto_Hendensho)/LConn1 -- _CN_161727149_500000_CN_169031921_500000/LConn1
  _CN_320438391_500000_CN_169031921_500000/RConn2 -- T_169031921_500000_西京都変電所_(Nishi_Kyōto_Hendensho)/LConn2 -- _CN_161727149_500000_CN_169031921_500000/LConn2
  _CN_320438391_500000_CN_169031921_500000/RConn3 -- T_169031921_500000_西京都変電所_(Nishi_Kyōto_Hendensho)/LConn3 -- _CN_161727149_500000_CN_169031921_500000/LConn3 -- bus243/LConn1
  T_315461259_500000_/LConn1 -- 富津火力線_CN_315461259_500000_CN_315461272_500000/LConn1
  T_315461259_500000_/LConn2 -- 富津火力線_CN_315461259_500000_CN_315461272_500000/LConn2
  富津火力線_CN_315461259_500000_CN_315461272_500000/LConn3 -- T_315461259_500000_/LConn3 -- bus244/LConn1
  富津火力線_CN_315461259_500000_CN_315461272_500000/RConn1 -- T_315461272_500000_新木更津変電所/LConn1 -- _CN_315461272_500000_CN_105298089_500000/LConn1
  富津火力線_CN_315461259_500000_CN_315461272_500000/RConn2 -- T_315461272_500000_新木更津変電所/LConn2 -- _CN_315461272_500000_CN_105298089_500000/LConn2
  富津火力線_CN_315461259_500000_CN_315461272_500000/RConn3 -- T_315461272_500000_新木更津変電所/LConn3 -- _CN_315461272_500000_CN_105298089_500000/LConn3 -- bus245/LConn1
  新茂木線_(Shin_Motegi_Sen)_CN_104530060_500000_CN_168839127_500000/RConn1 -- T_168839127__新茂木/LConn1 -- 福島幹線_CN_133135172_500000_CN_168839127_500000/LConn1 -- 福島幹線_CN_104391636_500000_CN_168839127_500000/LConn1
  新茂木線_(Shin_Motegi_Sen)_CN_104530060_500000_CN_168839127_500000/RConn2 -- T_168839127__新茂木/LConn2 -- 福島幹線_CN_133135172_500000_CN_168839127_500000/LConn2 -- 福島幹線_CN_104391636_500000_CN_168839127_500000/LConn2
  新茂木線_(Shin_Motegi_Sen)_CN_104530060_500000_CN_168839127_500000/RConn3 -- T_168839127__新茂木/LConn3 -- 福島幹線_CN_133135172_500000_CN_168839127_500000/LConn3 -- 福島幹線_CN_104391636_500000_CN_168839127_500000/LConn3 -- bus246/LConn1
  T_128581912_500000;275000;66000_新坂戸変電所/LConn1 -- 新坂戸線_CN_128581912_500000_CN_133641619_500000/LConn1
  T_128581912_500000;275000;66000_新坂戸変電所/LConn2 -- 新坂戸線_CN_128581912_500000_CN_133641619_500000/LConn2
  新坂戸線_CN_128581912_500000_CN_133641619_500000/LConn3 -- T_128581912_500000;275000;66000_新坂戸変電所/LConn3 -- bus247/LConn1
  新坂戸線_CN_128581912_500000_CN_133641619_500000/RConn1 -- T_133641619_500000_新所沢変電所_(Shin_Tokorozawa_Hendensho)/LConn1 -- 新古河線_(Shin_Koga_Sen)_CN_133135172_500000_CN_133641619_500000/LConn1 -- 新所沢線_(Shin_Tokorozawa_Sen)_CN_145079972_500000_CN_133641619_500000/RConn1
  新坂戸線_CN_128581912_500000_CN_133641619_500000/RConn2 -- T_133641619_500000_新所沢変電所_(Shin_Tokorozawa_Hendensho)/LConn2 -- 新古河線_(Shin_Koga_Sen)_CN_133135172_500000_CN_133641619_500000/LConn2 -- 新所沢線_(Shin_Tokorozawa_Sen)_CN_145079972_500000_CN_133641619_500000/RConn2
  新坂戸線_CN_128581912_500000_CN_133641619_500000/RConn3 -- T_133641619_500000_新所沢変電所_(Shin_Tokorozawa_Hendensho)/LConn3 -- 新古河線_(Shin_Koga_Sen)_CN_133135172_500000_CN_133641619_500000/LConn3 -- bus248/LConn1 -- 新所沢線_(Shin_Tokorozawa_Sen)_CN_145079972_500000_CN_133641619_500000/RConn3
  _CN_315608215_500000_CN_169249243_500000/LConn1 -- T_315608215_500000_/LConn1 -- 志賀中能登線_CN_315608215_500000_CN_255763556_500000/LConn1 -- _CN_315608215_500000_CN_169249247_500000/LConn1
  _CN_315608215_500000_CN_169249243_500000/LConn2 -- T_315608215_500000_/LConn2 -- 志賀中能登線_CN_315608215_500000_CN_255763556_500000/LConn2 -- _CN_315608215_500000_CN_169249247_500000/LConn2
  _CN_315608215_500000_CN_169249243_500000/LConn3 -- T_315608215_500000_/LConn3 -- 志賀中能登線_CN_315608215_500000_CN_255763556_500000/LConn3 -- _CN_315608215_500000_CN_169249247_500000/LConn3 -- bus249/LConn1
  _CN_315608215_500000_CN_169249243_500000/RConn1 -- T_169249243_500000_南福光変電所/LConn1 -- 加賀福光線_CN_169249243_500000_CN_169249247_500000/LConn1
  _CN_315608215_500000_CN_169249243_500000/RConn2 -- T_169249243_500000_南福光変電所/LConn2 -- 加賀福光線_CN_169249243_500000_CN_169249247_500000/LConn2
  _CN_315608215_500000_CN_169249243_500000/RConn3 -- T_169249243_500000_南福光変電所/LConn3 -- 加賀福光線_CN_169249243_500000_CN_169249247_500000/LConn3 -- bus250/LConn1
  G_255763556_志賀原子力発電所/RConn1 -- 志賀中能登線_CN_315608215_500000_CN_255763556_500000/RConn1
  G_255763556_志賀原子力発電所/RConn2 -- 志賀中能登線_CN_315608215_500000_CN_255763556_500000/RConn2
  志賀中能登線_CN_315608215_500000_CN_255763556_500000/RConn3 -- G_255763556_志賀原子力発電所/RConn3 -- bus251/LConn1
  _CN_315608215_500000_CN_169249247_500000/RConn1 -- T_169249247_500000_加賀変電所/LConn1 -- 加賀福光線_CN_169249243_500000_CN_169249247_500000/RConn1
  _CN_315608215_500000_CN_169249247_500000/RConn2 -- T_169249247_500000_加賀変電所/LConn2 -- 加賀福光線_CN_169249243_500000_CN_169249247_500000/RConn2
  _CN_315608215_500000_CN_169249247_500000/RConn3 -- T_169249247_500000_加賀変電所/LConn3 -- 加賀福光線_CN_169249243_500000_CN_169249247_500000/RConn3 -- bus252/LConn1
  _CN_315461272_500000_CN_105298089_500000/RConn1 -- T_105298089_500000_新佐原変電所/LConn1 -- _CN_105298089_500000_CN_132913106_500000/LConn1 -- _CN_105298089_500000_CN_168727982_500000/LConn1
  _CN_315461272_500000_CN_105298089_500000/RConn2 -- T_105298089_500000_新佐原変電所/LConn2 -- _CN_105298089_500000_CN_132913106_500000/LConn2 -- _CN_105298089_500000_CN_168727982_500000/LConn2
  _CN_315461272_500000_CN_105298089_500000/RConn3 -- T_105298089_500000_新佐原変電所/LConn3 -- _CN_105298089_500000_CN_132913106_500000/LConn3 -- _CN_105298089_500000_CN_168727982_500000/LConn3 -- bus253/LConn1
  _CN_170974371_500000_CN_241828221_500000/RConn1 -- T_241828221_500000_新岡山変電所_(Shin_Okayama_Hendensho)/LConn1 -- _CN_241828221_500000_CN_241822623_500000/LConn1 -- _CN_242103481_500000_CN_241828221_500000/RConn1
  _CN_170974371_500000_CN_241828221_500000/RConn2 -- T_241828221_500000_新岡山変電所_(Shin_Okayama_Hendensho)/LConn2 -- _CN_241828221_500000_CN_241822623_500000/LConn2 -- _CN_242103481_500000_CN_241828221_500000/RConn2
  _CN_170974371_500000_CN_241828221_500000/RConn3 -- T_241828221_500000_新岡山変電所_(Shin_Okayama_Hendensho)/LConn3 -- _CN_241828221_500000_CN_241822623_500000/LConn3 -- bus254/LConn1 -- _CN_242103481_500000_CN_241828221_500000/RConn3
  _CN_105298089_500000_CN_132913106_500000/RConn1 -- T_132913106_500000_新筑波変電所_(Shin_Tsukuba_Hendensho)/LConn1 -- 新筑波線_(Shin_Tsukuba_Sen)_CN_133135172_500000_CN_132913106_500000/LConn1 -- _CN_132913106_500000_CN_104391636_500000/LConn1
  _CN_105298089_500000_CN_132913106_500000/RConn2 -- T_132913106_500000_新筑波変電所_(Shin_Tsukuba_Hendensho)/LConn2 -- 新筑波線_(Shin_Tsukuba_Sen)_CN_133135172_500000_CN_132913106_500000/LConn2 -- _CN_132913106_500000_CN_104391636_500000/LConn2
  _CN_105298089_500000_CN_132913106_500000/RConn3 -- T_132913106_500000_新筑波変電所_(Shin_Tsukuba_Hendensho)/LConn3 -- 新筑波線_(Shin_Tsukuba_Sen)_CN_133135172_500000_CN_132913106_500000/LConn3 -- _CN_132913106_500000_CN_104391636_500000/LConn3 -- bus255/LConn1
  _CN_105298089_500000_CN_168727982_500000/RConn1 -- T_168727982_500000_新京葉変電所/LConn1 -- 房総線_CN_151379730_500000_CN_168727982_500000/LConn1 -- 新京葉線_CN_133135172_500000_CN_168727982_500000/LConn1
  _CN_105298089_500000_CN_168727982_500000/RConn2 -- T_168727982_500000_新京葉変電所/LConn2 -- 房総線_CN_151379730_500000_CN_168727982_500000/LConn2 -- 新京葉線_CN_133135172_500000_CN_168727982_500000/LConn2
  _CN_105298089_500000_CN_168727982_500000/RConn3 -- T_168727982_500000_新京葉変電所/LConn3 -- 房総線_CN_151379730_500000_CN_168727982_500000/LConn3 -- 新京葉線_CN_133135172_500000_CN_168727982_500000/LConn3 -- bus256/LConn1
  _CN_161727149_500000_CN_169031921_500000/RConn1 -- T_161727149_500000_新生駒変電所_(Shin_Ikoma_Hendensho)/LConn1 -- _CN_161727149_500000_CN_161870227_500000/RConn1 -- _CN_161727149_500000_CN_169359724_500000/LConn1
  _CN_161727149_500000_CN_169031921_500000/RConn2 -- T_161727149_500000_新生駒変電所_(Shin_Ikoma_Hendensho)/LConn2 -- _CN_161727149_500000_CN_161870227_500000/RConn2 -- _CN_161727149_500000_CN_169359724_500000/LConn2
  _CN_161727149_500000_CN_169031921_500000/RConn3 -- T_161727149_500000_新生駒変電所_(Shin_Ikoma_Hendensho)/LConn3 -- _CN_161727149_500000_CN_161870227_500000/RConn3 -- bus257/LConn1 -- _CN_161727149_500000_CN_169359724_500000/LConn3
  T_169359724_500000_信貴変電所_(Shingi_Hendensho)/LConn1 -- _CN_161727149_500000_CN_169359724_500000/RConn1
  T_169359724_500000_信貴変電所_(Shingi_Hendensho)/LConn2 -- _CN_161727149_500000_CN_169359724_500000/RConn2
  _CN_161727149_500000_CN_169359724_500000/RConn3 -- T_169359724_500000_信貴変電所_(Shingi_Hendensho)/LConn3 -- bus258/LConn1
  T_317511904_500000_北松江変電所/LConn1 -- _CN_242103481_500000_CN_317511904_500000/RConn1
  T_317511904_500000_北松江変電所/LConn2 -- _CN_242103481_500000_CN_317511904_500000/RConn2
  _CN_242103481_500000_CN_317511904_500000/RConn3 -- T_317511904_500000_北松江変電所/LConn3 -- bus259/LConn1
  _CN_242253500_500000_CN_204258596_500000/RConn1 -- T_204258596_500000_/LConn1 -- 関門連系線_CN_204258596_500000_CN_187988970_500000/RConn1 -- _CN_204258596_500000_CN_317416612_500000/RConn1
  _CN_242253500_500000_CN_204258596_500000/RConn2 -- T_204258596_500000_/LConn2 -- 関門連系線_CN_204258596_500000_CN_187988970_500000/RConn2 -- _CN_204258596_500000_CN_317416612_500000/RConn2
